simulink model "simulator_prototype_v2"  (R2021b)
(part 6 of 12)

t2391 = ct{934};
t2393 = ct{935};
t2394 = ct{936};
t2395 = ct{937};
t2396 = ct{938};
t2397 = ct{939};
t2398 = ct{940};
t2399 = ct{941};
t24 = ct{942};
t2400 = ct{943};
t2401 = ct{944};
t2402 = ct{945};
t2403 = ct{946};
t2404 = ct{947};
t2405 = ct{948};
t2408 = ct{949};
t2409 = ct{950};
t241 = ct{951};
t2410 = ct{952};
t2411 = ct{953};
t2412 = ct{954};
t2413 = ct{955};
t2414 = ct{956};
t2416 = ct{957};
t2417 = ct{958};
t2418 = ct{959};
t2419 = ct{960};
t2421 = ct{961};
t2422 = ct{962};
t2423 = ct{963};
t2425 = ct{964};
t2426 = ct{965};
t2427 = ct{966};
t2431 = ct{967};
t2432 = ct{968};
t2433 = ct{969};
t2434 = ct{970};
t2438 = ct{971};
t2440 = ct{972};
t2441 = ct{973};
t2444 = ct{974};
t2446 = ct{975};
t2447 = ct{976};
t2448 = ct{977};
t2449 = ct{978};
t2450 = ct{979};
t2451 = ct{980};
t2455 = ct{981};
t2457 = ct{982};
t2458 = ct{983};
t2459 = ct{984};
t2460 = ct{985};
t2461 = ct{986};
t2463 = ct{987};
t2465 = ct{988};
t2466 = ct{989};
t2467 = ct{990};
t2468 = ct{991};
t2470 = ct{992};
t2471 = ct{993};
t2472 = ct{994};
t2473 = ct{995};
t2474 = ct{996};
t2476 = ct{997};
t2477 = ct{998};
t2478 = ct{999};
t2479 = ct{1000};
t2480 = ct{1001};
t2481 = ct{1002};
t2484 = ct{1003};
t2485 = ct{1004};
t2487 = ct{1005};
t2488 = ct{1006};
t2489 = ct{1007};
t2490 = ct{1008};
t2491 = ct{1009};
t2492 = ct{1010};
t2493 = ct{1011};
t2494 = ct{1012};
t2496 = ct{1013};
t2497 = ct{1014};
t2498 = ct{1015};
t2499 = ct{1016};
t25 = ct{1017};
t2500 = ct{1018};
t2502 = ct{1019};
t2503 = ct{1020};
t2504 = ct{1021};
t2505 = ct{1022};
t2507 = ct{1023};
t2508 = ct{1024};
t2509 = ct{1025};
t2510 = ct{1026};
t2511 = ct{1027};
t2512 = ct{1028};
t2514 = ct{1029};
t2515 = ct{1030};
t2516 = ct{1031};
t2517 = ct{1032};
t2520 = ct{1033};
t2521 = ct{1034};
t2522 = ct{1035};
t2524 = ct{1036};
t2525 = ct{1037};
t2526 = ct{1038};
t2527 = ct{1039};
t2528 = ct{1040};
t2529 = ct{1041};
t2530 = ct{1042};
t2531 = ct{1043};
t2532 = ct{1044};
t2534 = ct{1045};
t2535 = ct{1046};
t2539 = ct{1047};
t2541 = ct{1048};
t2542 = ct{1049};
t2548 = ct{1050};
t2549 = ct{1051};
t2550 = ct{1052};
t2552 = ct{1053};
t2554 = ct{1054};
t2555 = ct{1055};
t2556 = ct{1056};
t2557 = ct{1057};
t2558 = ct{1058};
t2559 = ct{1059};
t2560 = ct{1060};
t2564 = ct{1061};
t2565 = ct{1062};
t2566 = ct{1063};
t2569 = ct{1064};
t257 = ct{1065};
t2570 = ct{1066};
t2571 = ct{1067};
t2572 = ct{1068};
t2575 = ct{1069};
t2577 = ct{1070};
t2578 = ct{1071};
t2579 = ct{1072};
t2580 = ct{1073};
t2581 = ct{1074};
t2582 = ct{1075};
t2583 = ct{1076};
t2584 = ct{1077};
t2585 = ct{1078};
t2586 = ct{1079};
t2587 = ct{1080};
t2589 = ct{1081};
t259 = ct{1082};
t2595 = ct{1083};
t2597 = ct{1084};
t2599 = ct{1085};
t26 = ct{1086};
t2600 = ct{1087};
t2601 = ct{1088};
t2603 = ct{1089};
t2604 = ct{1090};
t2605 = ct{1091};
t2606 = ct{1092};
t261 = ct{1093};
t2610 = ct{1094};
t2611 = ct{1095};
t2612 = ct{1096};
t2613 = ct{1097};
t2614 = ct{1098};
t2616 = ct{1099};
t2618 = ct{1100};
t2619 = ct{1101};
t262 = ct{1102};
t2620 = ct{1103};
t2621 = ct{1104};
t2622 = ct{1105};
t2623 = ct{1106};
t2624 = ct{1107};
t2626 = ct{1108};
t2627 = ct{1109};
t2628 = ct{1110};
t2629 = ct{1111};
t2630 = ct{1112};
t2632 = ct{1113};
t2633 = ct{1114};
t2634 = ct{1115};
t2635 = ct{1116};
t2638 = ct{1117};
t264 = ct{1118};
t2640 = ct{1119};
t2641 = ct{1120};
t2642 = ct{1121};
t2643 = ct{1122};
t2644 = ct{1123};
t2645 = ct{1124};
t2646 = ct{1125};
t2647 = ct{1126};
t2648 = ct{1127};
t2649 = ct{1128};
t2650 = ct{1129};
t2651 = ct{1130};
t2652 = ct{1131};
t2653 = ct{1132};
t2654 = ct{1133};
t2655 = ct{1134};
t2657 = ct{1135};
t2658 = ct{1136};
t2659 = ct{1137};
t2660 = ct{1138};
t2661 = ct{1139};
t2662 = ct{1140};
t2664 = ct{1141};
t2665 = ct{1142};
t2666 = ct{1143};
t2667 = ct{1144};
t2668 = ct{1145};
t2670 = ct{1146};
t2671 = ct{1147};
t2672 = ct{1148};
t2673 = ct{1149};
t2674 = ct{1150};
t2675 = ct{1151};
t2676 = ct{1152};
t2678 = ct{1153};
t2679 = ct{1154};
t2680 = ct{1155};
t2681 = ct{1156};
t2682 = ct{1157};
t2683 = ct{1158};
t2684 = ct{1159};
t2685 = ct{1160};
t2686 = ct{1161};
t2687 = ct{1162};
t2688 = ct{1163};
t2691 = ct{1164};
t2692 = ct{1165};
t2694 = ct{1166};
t2695 = ct{1167};
t2697 = ct{1168};
t2698 = ct{1169};
t2699 = ct{1170};
t27 = ct{1171};
t2701 = ct{1172};
t2703 = ct{1173};
t2707 = ct{1174};
t2708 = ct{1175};
t2709 = ct{1176};
t271 = ct{1177};
t2710 = ct{1178};
t2711 = ct{1179};
t2712 = ct{1180};
t2714 = ct{1181};
t2716 = ct{1182};
t2732 = ct{1183};
t2733 = ct{1184};
t2735 = ct{1185};
t2736 = ct{1186};
t2737 = ct{1187};
t2738 = ct{1188};
t2739 = ct{1189};
t2740 = ct{1190};
t2742 = ct{1191};
t2743 = ct{1192};
t2744 = ct{1193};
t2745 = ct{1194};
t2748 = ct{1195};
t2749 = ct{1196};
t2750 = ct{1197};
t2753 = ct{1198};
t2754 = ct{1199};
t2757 = ct{1200};
t2759 = ct{1201};
t276 = ct{1202};
t2762 = ct{1203};
t2765 = ct{1204};
t2769 = ct{1205};
t2771 = ct{1206};
t2773 = ct{1207};
t2774 = ct{1208};
t2775 = ct{1209};
t2777 = ct{1210};
t2778 = ct{1211};
t2779 = ct{1212};
t2781 = ct{1213};
t2785 = ct{1214};
t2786 = ct{1215};
t2787 = ct{1216};
t2788 = ct{1217};
t279 = ct{1218};
t2790 = ct{1219};
t2791 = ct{1220};
t2792 = ct{1221};
t2793 = ct{1222};
t2795 = ct{1223};
t2796 = ct{1224};
t2797 = ct{1225};
t2798 = ct{1226};
t2799 = ct{1227};
t28 = ct{1228};
t280 = ct{1229};
t2801 = ct{1230};
t2802 = ct{1231};
t2803 = ct{1232};
t2804 = ct{1233};
t2805 = ct{1234};
t2806 = ct{1235};
t2807 = ct{1236};
t2808 = ct{1237};
t2810 = ct{1238};
t2811 = ct{1239};
t2812 = ct{1240};
t2813 = ct{1241};
t2814 = ct{1242};
t2817 = ct{1243};
t2818 = ct{1244};
t2819 = ct{1245};
t2820 = ct{1246};
t2823 = ct{1247};
t2825 = ct{1248};
t2831 = ct{1249};
t2832 = ct{1250};
t2835 = ct{1251};
t2838 = ct{1252};
t2850 = ct{1253};
t2851 = ct{1254};
t2857 = ct{1255};
t2858 = ct{1256};
t2859 = ct{1257};
t286 = ct{1258};
t2865 = ct{1259};
t2867 = ct{1260};
t2868 = ct{1261};
t2870 = ct{1262};
t2875 = ct{1263};
t2883 = ct{1264};
t2884 = ct{1265};
t2886 = ct{1266};
t2890 = ct{1267};
t2893 = ct{1268};
t2894 = ct{1269};
t2895 = ct{1270};
t2898 = ct{1271};
t29 = ct{1272};
t2900 = ct{1273};
t2901 = ct{1274};
t2903 = ct{1275};
t2905 = ct{1276};
t2909 = ct{1277};
t2911 = ct{1278};
t2914 = ct{1279};
t2917 = ct{1280};
t2918 = ct{1281};
t2919 = ct{1282};
t2920 = ct{1283};
t2922 = ct{1284};
t2923 = ct{1285};
t2925 = ct{1286};
t2926 = ct{1287};
t2927 = ct{1288};
t293 = ct{1289};
t2930 = ct{1290};
t2931 = ct{1291};
t2933 = ct{1292};
t2935 = ct{1293};
t2937 = ct{1294};
t2941 = ct{1295};
t2942 = ct{1296};
t2943 = ct{1297};
t2944 = ct{1298};
t2947 = ct{1299};
t2948 = ct{1300};
t2949 = ct{1301};
t2950 = ct{1302};
t2951 = ct{1303};
t2952 = ct{1304};
t2955 = ct{1305};
t2956 = ct{1306};
t2961 = ct{1307};
t2962 = ct{1308};
t2963 = ct{1309};
t2964 = ct{1310};
t2965 = ct{1311};
t2966 = ct{1312};
t2969 = ct{1313};
t2970 = ct{1314};
t2971 = ct{1315};
t2972 = ct{1316};
t2973 = ct{1317};
t2975 = ct{1318};
t2976 = ct{1319};
t2977 = ct{1320};
t2978 = ct{1321};
t2979 = ct{1322};
t2981 = ct{1323};
t2982 = ct{1324};
t2983 = ct{1325};
t2984 = ct{1326};
t2986 = ct{1327};
t2987 = ct{1328};
t2990 = ct{1329};
t2991 = ct{1330};
t2993 = ct{1331};
t2999 = ct{1332};
t30 = ct{1333};
t3000 = ct{1334};
t3004 = ct{1335};
t3005 = ct{1336};
t3008 = ct{1337};
t3010 = ct{1338};
t3011 = ct{1339};
t3012 = ct{1340};
t3015 = ct{1341};
t3017 = ct{1342};
t3018 = ct{1343};
t3019 = ct{1344};
t3022 = ct{1345};
t3023 = ct{1346};
t3026 = ct{1347};
t3027 = ct{1348};
t3029 = ct{1349};
t3030 = ct{1350};
t3036 = ct{1351};
t3037 = ct{1352};
t3042 = ct{1353};
t3043 = ct{1354};
t3044 = ct{1355};
t3045 = ct{1356};
t3049 = ct{1357};
t305 = ct{1358};
t3050 = ct{1359};
t3051 = ct{1360};
t3054 = ct{1361};
t3057 = ct{1362};
t3058 = ct{1363};
t306 = ct{1364};
t3064 = ct{1365};
t3065 = ct{1366};
t3066 = ct{1367};
t3067 = ct{1368};
t3068 = ct{1369};
t3069 = ct{1370};
t3072 = ct{1371};
t3074 = ct{1372};
t3075 = ct{1373};
t3076 = ct{1374};
t3077 = ct{1375};
t3079 = ct{1376};
t308 = ct{1377};
t3080 = ct{1378};
t3081 = ct{1379};
t3082 = ct{1380};
t3083 = ct{1381};
t3085 = ct{1382};
t3086 = ct{1383};
t3087 = ct{1384};
t3088 = ct{1385};
t31 = ct{1386};
t310 = ct{1387};
t3119 = ct{1388};
t312 = ct{1389};
t3120 = ct{1390};
t313 = ct{1391};
t3130 = ct{1392};
t314 = ct{1393};
t3154 = ct{1394};
t3155 = ct{1395};
t316 = ct{1396};
t3160 = ct{1397};
t3166 = ct{1398};
t3172 = ct{1399};
t3173 = ct{1400};
t319 = ct{1401};
t32 = ct{1402};
t321 = ct{1403};
t322 = ct{1404};
t326 = ct{1405};
t328 = ct{1406};
t329 = ct{1407};
t33 = ct{1408};
t330 = ct{1409};
t331 = ct{1410};
t3313 = ct{1411};
t3315 = ct{1412};
t332 = ct{1413};
t3320 = ct{1414};
t3327 = ct{1415};
t333 = ct{1416};
t335 = ct{1417};
t336 = ct{1418};
t338 = ct{1419};
t3381 = ct{1420};
t3382 = ct{1421};
t3384 = ct{1422};
t3385 = ct{1423};
t339 = ct{1424};
t3390 = ct{1425};
t3391 = ct{1426};
t34 = ct{1427};
t341 = ct{1428};
t343 = ct{1429};
t346 = ct{1430};
t347 = ct{1431};
t3470 = ct{1432};
t3471 = ct{1433};
t35 = ct{1434};
t350 = ct{1435};
t351 = ct{1436};
t352 = ct{1437};
t3523 = ct{1438};
t3533 = ct{1439};
t354 = ct{1440};
t356 = ct{1441};
t358 = ct{1442};
t359 = ct{1443};
t36 = ct{1444};
t360 = ct{1445};
t362 = ct{1446};
t363 = ct{1447};
t3638 = ct{1448};
t364 = ct{1449};
t3649 = ct{1450};
t365 = ct{1451};
t366 = ct{1452};
t369 = ct{1453};
t370 = ct{1454};
t371 = ct{1455};
t372 = ct{1456};
t3767 = ct{1457};
t378 = ct{1458};
t38 = ct{1459};
t380 = ct{1460};
t3806 = ct{1461};
t3807 = ct{1462};
t382 = ct{1463};
t3837 = ct{1464};
t3838 = ct{1465};
t387 = ct{1466};
t3875 = ct{1467};
t3876 = ct{1468};
t3877 = ct{1469};
t3878 = ct{1470};
t3879 = ct{1471};
t39 = ct{1472};
t393 = ct{1473};
t3974 = ct{1474};
t3995 = ct{1475};
t4035 = ct{1476};
t410 = ct{1477};
t4147 = ct{1478};
t4153 = ct{1479};
t4154 = ct{1480};
t42 = ct{1481};
t4260 = ct{1482};
t428 = ct{1483};
t429 = ct{1484};
t43 = ct{1485};
t4314 = ct{1486};
t4325 = ct{1487};
t4327 = ct{1488};
t4334 = ct{1489};
t4338 = ct{1490};
t4343 = ct{1491};
t4476 = ct{1492};
t4563 = ct{1493};
t46 = ct{1494};
t461 = ct{1495};
t4683 = ct{1496};
t47 = ct{1497};
t4705 = ct{1498};
t4716 = ct{1499};
t473 = ct{1500};
t474 = ct{1501};
t4762 = ct{1502};
t4763 = ct{1503};
t480 = ct{1504};
t4847 = ct{1505};
t4850 = ct{1506};
t498 = ct{1507};
t50 = ct{1508};
t5025 = ct{1509};
t5027 = ct{1510};
t503 = ct{1511};
t5036 = ct{1512};
t504 = ct{1513};
t506 = ct{1514};
t510 = ct{1515};
t514 = ct{1516};
t516 = ct{1517};
t521 = ct{1518};
t522 = ct{1519};
t523 = ct{1520};
t524 = ct{1521};
t528 = ct{1522};
t5296 = ct{1523};
t530 = ct{1524};
t535 = ct{1525};
t5370 = ct{1526};
t538 = ct{1527};
t539 = ct{1528};
t542 = ct{1529};
t543 = ct{1530};
t5437 = ct{1531};
t549 = ct{1532};
t56 = ct{1533};
t562 = ct{1534};
t563 = ct{1535};
t564 = ct{1536};
t573 = ct{1537};
t575 = ct{1538};
t577 = ct{1539};
t579 = ct{1540};
t58 = ct{1541};
t580 = ct{1542};
t581 = ct{1543};
t587 = ct{1544};
t59 = ct{1545};
t593 = ct{1546};
t594 = ct{1547};
t598 = ct{1548};
t60 = ct{1549};
t610 = ct{1550};
t611 = ct{1551};
t612 = ct{1552};
t614 = ct{1553};
t615 = ct{1554};
t616 = ct{1555};
t623 = ct{1556};
t624 = ct{1557};
t628 = ct{1558};
t635 = ct{1559};
t636 = ct{1560};
t638 = ct{1561};
t640 = ct{1562};
t641 = ct{1563};
t642 = ct{1564};
t643 = ct{1565};
t644 = ct{1566};
t645 = ct{1567};
t646 = ct{1568};
t648 = ct{1569};
t649 = ct{1570};
t654 = ct{1571};
t655 = ct{1572};
t656 = ct{1573};
t657 = ct{1574};
t658 = ct{1575};
t659 = ct{1576};
t660 = ct{1577};
t662 = ct{1578};
t663 = ct{1579};
t664 = ct{1580};
t665 = ct{1581};
t666 = ct{1582};
t667 = ct{1583};
t668 = ct{1584};
t669 = ct{1585};
t67 = ct{1586};
t670 = ct{1587};
t672 = ct{1588};
t673 = ct{1589};
t674 = ct{1590};
t675 = ct{1591};
t676 = ct{1592};
t677 = ct{1593};
t678 = ct{1594};
t679 = ct{1595};
t68 = ct{1596};
t680 = ct{1597};
t681 = ct{1598};
t682 = ct{1599};
t683 = ct{1600};
t684 = ct{1601};
t685 = ct{1602};
t686 = ct{1603};
t687 = ct{1604};
t689 = ct{1605};
t691 = ct{1606};
t692 = ct{1607};
t693 = ct{1608};
t694 = ct{1609};
t696 = ct{1610};
t698 = ct{1611};
t70 = ct{1612};
t702 = ct{1613};
t704 = ct{1614};
t705 = ct{1615};
t707 = ct{1616};
t708 = ct{1617};
t71 = ct{1618};
t710 = ct{1619};
t711 = ct{1620};
t712 = ct{1621};
t713 = ct{1622};
t714 = ct{1623};
t715 = ct{1624};
t716 = ct{1625};
t717 = ct{1626};
t718 = ct{1627};
t719 = ct{1628};
t720 = ct{1629};
t721 = ct{1630};
t722 = ct{1631};
t723 = ct{1632};
t724 = ct{1633};
t725 = ct{1634};
t726 = ct{1635};
t728 = ct{1636};
t73 = ct{1637};
t733 = ct{1638};
t736 = ct{1639};
t738 = ct{1640};
t740 = ct{1641};
t741 = ct{1642};
t742 = ct{1643};
t743 = ct{1644};
t744 = ct{1645};
t745 = ct{1646};
t746 = ct{1647};
t747 = ct{1648};
t749 = ct{1649};
t750 = ct{1650};
t751 = ct{1651};
t755 = ct{1652};
t756 = ct{1653};
t757 = ct{1654};
t758 = ct{1655};
t759 = ct{1656};
t76 = ct{1657};
t762 = ct{1658};
t763 = ct{1659};
t764 = ct{1660};
t766 = ct{1661};
t767 = ct{1662};
t768 = ct{1663};
t770 = ct{1664};
t771 = ct{1665};
t772 = ct{1666};
t773 = ct{1667};
t774 = ct{1668};
t775 = ct{1669};
t776 = ct{1670};
t777 = ct{1671};
t778 = ct{1672};
t781 = ct{1673};
t782 = ct{1674};
t783 = ct{1675};
t784 = ct{1676};
t785 = ct{1677};
t786 = ct{1678};
t787 = ct{1679};
t789 = ct{1680};
t790 = ct{1681};
t791 = ct{1682};
t792 = ct{1683};
t793 = ct{1684};
t794 = ct{1685};
t796 = ct{1686};
t797 = ct{1687};
t798 = ct{1688};
t799 = ct{1689};
t8 = ct{1690};
t800 = ct{1691};
t801 = ct{1692};
t802 = ct{1693};
t806 = ct{1694};
t807 = ct{1695};
t808 = ct{1696};
t809 = ct{1697};
t812 = ct{1698};
t813 = ct{1699};
t816 = ct{1700};
t817 = ct{1701};
t818 = ct{1702};
t819 = ct{1703};
t820 = ct{1704};
t821 = ct{1705};
t822 = ct{1706};
t823 = ct{1707};
t824 = ct{1708};
t825 = ct{1709};
t826 = ct{1710};
t827 = ct{1711};
t828 = ct{1712};
t829 = ct{1713};
t830 = ct{1714};
t831 = ct{1715};
t832 = ct{1716};
t833 = ct{1717};
t850 = ct{1718};
t855 = ct{1719};
t856 = ct{1720};
t874 = ct{1721};
t878 = ct{1722};
t89 = ct{1723};
t893 = ct{1724};
t9 = ct{1725};
t90 = ct{1726};
t91 = ct{1727};
t911 = ct{1728};
t92 = ct{1729};
t925 = ct{1730};
t926 = ct{1731};
t936 = ct{1732};
t937 = ct{1733};
t940 = ct{1734};
t941 = ct{1735};
t942 = ct{1736};
t944 = ct{1737};
t945 = ct{1738};
t948 = ct{1739};
t949 = ct{1740};
t950 = ct{1741};
t951 = ct{1742};
t959 = ct{1743};
t961 = ct{1744};
t965 = ct{1745};
t966 = ct{1746};
t97 = ct{1747};
t974 = ct{1748};
t978 = ct{1749};
t983 = ct{1750};
t987 = ct{1751};
t989 = ct{1752};
t99 = ct{1753};
t990 = ct{1754};
t991 = ct{1755};
t992 = ct{1756};
t993 = ct{1757};
t995 = ct{1758};
t996 = ct{1759};
t998 = ct{1760};
t3121 = t35.*t991.*t2699.*2.196325630278387e-1;
t3122 = t36.*t991.*t2699.*2.196325630278387e-1;
t3126 = t50.*t202.*t2981.*4.771516396025243e-17;
t3127 = t50.*t202.*t2981.*9.543032792050485e-17;
t3131 = (t2307.*t2363)./1.0e+8;
t3132 = (t2297.*t2388)./1.0e+8;
t3134 = t2363.*t2554;
t3137 = t38.*t1022.*(t855-t878).*(-2.196325630278387e-1);
t3138 = t39.*t1022.*(t855-t878).*(-2.196325630278387e-1);
t3140 = (t2297.*t2419)./1.0e+8;
t3141 = (t2338.*t2363)./1.0e+8;
t3144 = t35.*t991.*t2699.*1.122398993609262e-1;
t3145 = t36.*t991.*t2699.*1.122398993609262e-1;
t3148 = t35.*t991.*t2699.*1.887873611596568e-1;
t3149 = t36.*t991.*t2699.*1.887873611596568e-1;
t3150 = t35.*t991.*t2699.*5.076068728976717e-3;
t3151 = t36.*t991.*t2699.*5.076068728976717e-3;
t3157 = t2307.*t2363.*6.2e-7;
t3158 = t2297.*t2388.*6.2e-7;
t3159 = t2363.*t2801;
t3163 = t2297.*t2419.*6.2e-7;
t3164 = t2338.*t2363.*6.2e-7;
t3165 = t2363.*t2831;
t3168 = t38.*t1022.*(t855-t878).*(-1.122398993609262e-1);
t3169 = t39.*t1022.*(t855-t878).*(-1.122398993609262e-1);
t3170 = t2363.*t2850;
t3171 = t2363.*t2851;
t3174 = t38.*t1022.*(t855-t878).*(-1.887873611596568e-1);
t3175 = t39.*t1022.*(t855-t878).*(-1.887873611596568e-1);
t3176 = t39.*t1022.*(t855-t878).*1.887873611596568e-1;
t3177 = t38.*t1022.*(t855-t878).*(-5.076068728976717e-3);
t3178 = t39.*t1022.*(t855-t878).*(-5.076068728976717e-3);
t3179 = t38.*t1022.*(t855-t878).*5.076068728976717e-3;
t3180 = t39.*t1022.*(t855-t878).*5.076068728976717e-3;
t3182 = t2363.*t2973;
t3183 = t2388.*t2971;
t3184 = t2388.*t2972;
t3186 = t2388.*t2973;
t3191 = t2399.*t2973;
t3204 = t2363.*t2976;
t3210 = t38.*t1022.*(t855-t878).*(-1.46680315462752e-4);
t3211 = t39.*t1022.*(t855-t878).*(-1.46680315462752e-4);
t3212 = t39.*t1022.*(t855-t878).*1.46680315462752e-4;
t3213 = t598+t1904+t2554;
t3274 = t35.*t941.*t948.*(t850-t874).*(-4.392651260556773e-1);
t3275 = t36.*t941.*t948.*(t850-t874).*(-4.392651260556773e-1);
t3276 = t35.*t941.*t948.*(t850-t874).*4.392651260556773e-1;
t3277 = t36.*t941.*t948.*(t850-t874).*4.392651260556773e-1;
t3318 = t201.*t3166.*4.297799892626299e-1;
t3319 = t201.*t3166.*8.595599785252598e-1;
t3322 = t535+t577+t1887+t1940;
t3369 = t564+t611+t1929+t1967;
t3371 = t35.*t941.*t948.*(t850-t874).*(-2.244797987218524e-1);
t3372 = t36.*t941.*t948.*(t850-t874).*(-2.244797987218524e-1);
t3373 = t36.*t941.*t948.*(t850-t874).*(-3.775747223193135e-1);
t3374 = t35.*t941.*t948.*(t850-t874).*(-3.775747223193135e-1);
t3375 = t36.*t941.*t948.*(t850-t874).*3.775747223193135e-1;
t3377 = t35.*t941.*t948.*(t850-t874).*(-1.015213745795343e-2);
t3378 = t36.*t941.*t948.*(t850-t874).*(-1.015213745795343e-2);
t3379 = t35.*t941.*t948.*(t850-t874).*1.015213745795343e-2;
t3380 = t36.*t941.*t948.*(t850-t874).*1.015213745795343e-2;
t3388 = -t3385;
t3393 = -t3390;
t3394 = -t3391;
t3427 = t50.*t202.*t3166.*9.543032792050485e-17;
t3472 = -t3471;
t3484 = t2363.*t3155;
t3485 = t2388.*t3155;
t3487 = t2419.*t3155;
t3499 = t998+t1036+t1059+t1481+t1519;
t3517 = t1019+t1060+t1072+t1503+t1537;
t3805 = t1021+t1024+t1053+t1490+t1498+t1512;
t3809 = t1582+t1647+t1769+t1961+t2034;
t3880 = t1619+t1739+t1774+t1991+t2057+t2079;
t3897 = t58+t59+t3878;
t3898 = t56+t73+t3879;
t3901 = t539+t577+t581+t593+t1909+t1937+t1939+t1940;
t3902 = t538+t573+t575+t579+t1924+t1935+t1936+t1957;
t3903 = t1038+t1043+t1056+t1057+t1501+t1507+t1517+t1531;
t3944 = -t20.*(t1941-t3315+t39.*t1022.*(t855-t878).*2.196325630278387e-1);
t3945 = -t26.*(t1941-t3315+t39.*t1022.*(t855-t878).*2.196325630278387e-1);
t3947 = -t21.*(t1959-t3313+t38.*t1022.*(t855-t878).*2.196325630278387e-1);
t3948 = -t27.*(t1959-t3313+t38.*t1022.*(t855-t878).*2.196325630278387e-1);
t3950 = t21.*(t1959-t3313+t38.*t1022.*(t855-t878).*2.196325630278387e-1).*(-3.0./5.0e+2);
t3982 = t27.*(t1959-t3313+t38.*t1022.*(t855-t878).*2.196325630278387e-1).*(-1.247162e-2);
t3989 = t20.*(t1941-t3315+t39.*t1022.*(t855-t878).*2.196325630278387e-1).*(-5.84482e-3);
t3990 = t27.*(t1959-t3313+t38.*t1022.*(t855-t878).*2.196325630278387e-1).*1.247162e-2;
t3994 = t20.*(t1941-t3315+t39.*t1022.*(t855-t878).*2.196325630278387e-1).*(-6.48e-5);
t4000 = t21.*(t1959-t3313+t38.*t1022.*(t855-t878).*2.196325630278387e-1).*(-3.131399999999998e-4);
t4003 = t26.*(t1941-t3315+t39.*t1022.*(t855-t878).*2.196325630278387e-1).*(-6.47e-6);
t4004 = t21.*(t1959-t3313+t38.*t1022.*(t855-t878).*2.196325630278387e-1).*(-4.36041e-5);
t4005 = t26.*(t1941-t3315+t39.*t1022.*(t855-t878).*2.196325630278387e-1).*6.47e-6;
t4008 = t1000+t1002+t1006+t1028+t1040+t1054+t1493+t1500+t1506;
t4038 = t20.*(t1941-t3315+t39.*t1022.*(t855-t878).*2.196325630278387e-1).*(-1.688944904408e-4);
t4040 = t21.*(t1959-t3313+t38.*t1022.*(t855-t878).*2.196325630278387e-1).*(-6.1855407534e-5);
t4043 = t27.*(t1959-t3313+t38.*t1022.*(t855-t878).*2.196325630278387e-1).*(-1.35652563578e-4);
t4044 = t20.*(t1941-t3315+t39.*t1022.*(t855-t878).*2.196325630278387e-1).*1.688944904408e-4;
t4050 = t20.*(t1941-t3315+t39.*t1022.*(t855-t878).*2.196325630278387e-1).*(-7.0482312e-7);
t4055 = t26.*(t1941-t3315+t39.*t1022.*(t855-t878).*2.196325630278387e-1).*(-1.869599668e-7);
t4057 = t20.*(t1941-t3315+t39.*t1022.*(t855-t878).*2.196325630278387e-1).*7.0482312e-7;
t4167 = -t28.*(t1005+t20.*(t1941-t3315+t39.*t1022.*(t855-t878).*2.196325630278387e-1));
t4170 = -t22.*(t1005+t20.*(t1941-t3315+t39.*t1022.*(t855-t878).*2.196325630278387e-1));
t4177 = t22.*(t1005+t20.*(t1941-t3315+t39.*t1022.*(t855-t878).*2.196325630278387e-1));
t4222 = t28.*(t1005+t20.*(t1941-t3315+t39.*t1022.*(t855-t878).*2.196325630278387e-1)).*(-1.838876e-2);
t4232 = t50.*t189.*(t1941-t3315+t39.*t1022.*(t855-t878).*2.196325630278387e-1).*(-4.306286555174926e-24);
t4234 = t50.*t189.*(t1959-t3313+t38.*t1022.*(t855-t878).*2.196325630278387e-1).*(-7.660522649005482e-24);
t4255 = t28.*(t1005+t20.*(t1941-t3315+t39.*t1022.*(t855-t878).*2.196325630278387e-1)).*(-1.33637554986e-4);
t4273 = t1098+t1129+t1142+t1156+t2455+t2484+t2490+t2524;
t4274 = t1099+t1135+t1160+t1169+t2451+t2457+t2511+t2512;
t4275 = t1699+t1745+t1767+t1768+t2039+t2093+t2095+t2107;
t4313 = t312+t316+t4153;
t4315 = t314+t319+t4154;
t4324 = t1593+t1621+t1625+t1632+t1743+t1778+t1997+t2035+t2094;
t4326 = t1592+t1603+t1610+t1875+t1883+t1891+t1910+t1925+t1934;
t4348 = -t3166.*(t1959-t3313+t38.*t1022.*(t855-t878).*2.196325630278387e-1);
t4349 = t99+t107+t108+t124+t130+t139+t280+t286+t305+t310+t614+t623+t624+t658+t698+t767+t993+t995+t1011+t1033;
t4351 = t216+t230+t261+t276+t474+t480+t503+t510+t926+t936+t961+t987+t1432+t1439+t1464+t1465;
t4375 = t100+t101+t126+t128+t134+t257+t279+t293+t306+t308+t615+t616+t662+t696+t733+t978+t990+t992+t1034+t1037;
t4421 = -t3155.*(t1005+t20.*(t1941-t3315+t39.*t1022.*(t855-t878).*2.196325630278387e-1));
t4424 = t3155.*(t1005+t20.*(t1941-t3315+t39.*t1022.*(t855-t878).*2.196325630278387e-1));
t4501 = t2143+t2161+t2163+t2340+t2409+t2411+t2425+t2485+t2489;
t4502 = t1444+t1462+t1476+t1487+t1489+t1495+t1534+t1540+t1850+t1857+t1867+t1869;
t4652 = t680+t942+t965+t1103+t1133+t1200+t1211+t1510+t1551+t1555+t1556+t1557+t1574+t1575;
t4663 = (t3837.*t3876)./2.0;
t4664 = (t3838.*t3877)./2.0;
t4704 = (t3806.*t4147)./2.0;
t4707 = t3807.*(t1089-t1104-t1105-t1121-t2117+t2120+t2122+t2123).*(-1.0./2.0);
t4708 = (t3807.*(t1089-t1104-t1105-t1121-t2117+t2120+t2122+t2123))./2.0;
t4709 = t925+t1331+t1372+t1453+t1457+t1472+t1502+t1508+t1786+t1801+t1803+t1818+t1856+t1858;
t4729 = t3807.*(t313-t314-t1108+t1115-t1158-t1159-t2117+t2120+t2122+t2123).*(-1.0./2.0);
t4730 = (t3807.*(t313-t314-t1108+t1115-t1158-t1159-t2117+t2120+t2122+t2123))./2.0;
t4900 = t3878.*(t313-t314-t1108+t1115-t1158-t1159-t2117+t2120+t2122+t2123).*(-1.0./2.0);
t4902 = (t3878.*(t313-t314-t1108+t1115-t1158-t1159-t2117+t2120+t2122+t2123))./2.0;
t5037 = t151+t182+t203+t231+t239+t259+t271+t393+t428+t461+t473+t498+t504+t506+t856+t893+t911+t937+t940+t959+t966+t1195+t1266+t1377+t1388+t1431+t1466+t1467;
t5278 = t704+t705+t726+t728+t755+t778+t781+t797+t1670+t1675+t1713+t1714+t1718+t1719+t1733+t1734+t1988+t1990+t2009+t2010+t2017+t2027+t2036+t2074;
t5279 = t719+t742+t747+t750+t751+t763+t773+t775+t1642+t1655+t1657+t1662+t1663+t1684+t1709+t1724+t1984+t2005+t2031+t2033+t2052+t2059+t2067+t2068;
t5282 = t236.*t241.*t4035.*t4705.*1.16903445774439e-94;
t5308 = t236.*t241.*t3974.*t4716.*1.16903445774439e-94;
t5309 = t236.*t241.*t3995.*t4716.*2.394182569460511e-91;
t5361 = t236.*t241.*t4314.*t4705.*2.156487945535858e-75;
t5363 = t236.*t241.*t4260.*t4716.*2.156487945535858e-75;
t5372 = t236.*t241.*t3995.*t4850.*2.658076613771277e-107;
t5381 = t236.*t241.*t4334.*t4705.*2.394182569460511e-91;
t5391 = t236.*t241.*t4325.*t4716.*2.394182569460511e-91;
t5395 = t236.*t241.*t4327.*t4716.*2.156487945535858e-75;
t5402 = t236.*t241.*t4343.*t4716.*2.156487945535858e-75;
t5404 = t236.*t241.*t4338.*t4716.*1.16903445774439e-94;
t5433 = t236.*t241.*t4334.*t4763.*2.658076613771277e-107;
t5434 = t236.*t241.*t4325.*t4850.*2.658076613771277e-107;
t5435 = t236.*t241.*t4035.*t5025.*6.337348493984406e-114;
t5439 = t236.*t241.*t4327.*t4850.*2.394182569460511e-91;
t5450 = t236.*t241.*t3974.*t5036.*6.337348493984406e-114;
t5457 = t236.*t241.*t3995.*t5036.*1.297888971568006e-110;
t5459 = t236.*t241.*t4343.*t4850.*2.394182569460511e-91;
t5463 = t236.*t241.*t4338.*t4850.*1.297888971568006e-110;
t5481 = t236.*t241.*t4314.*t5025.*1.16903445774439e-94;
t5499 = t236.*t241.*t4260.*t5036.*1.16903445774439e-94;
t5540 = t1305+t1307+t1316+t1317+t1342+t1399+t1404+t1436+t2184+t2202+t2207+t2258+t2274+t2275+t2277+t2278+t2541+t2560+t2589+t2595+t2597+t2623+t2624+t2634;
t5541 = t1300+t1311+t1337+t1338+t1379+t1392+t1394+t1398+t2179+t2181+t2200+t2201+t2232+t2241+t2271+t2276+t2580+t2582+t2587+t2611+t2629+t2630+t2655+t2662;
t5542 = t236.*t241.*t4476.*t4850.*2.658076613771277e-107;
t5545 = t236.*t241.*t4327.*t5036.*1.16903445774439e-94;
t5550 = t236.*t241.*t4338.*t5036.*6.337348493984406e-114;
t5570 = t236.*t241.*t4683.*t4850.*1.297888971568006e-110;
t5604 = t236.*t241.*t4476.*t5036.*1.297888971568006e-110;
t5684 = t236.*t241.*t4683.*t5036.*6.337348493984406e-114;
t5782 = t1076+t1078+t1079+t1097+t1119+t1120+t1125+t1127+t1128+t1136+t1140+t1144+t1152+t1153+t1164+t1175+t2417+t2418+t2426+t2431+t2432+t2444+t2466+t2467+t2476+t2477+t2480+t2481+t2491+t2505+t2514+t2516;
t5783 = t1074+t1075+t1077+t1088+t1109+t1111+t1116+t1130+t1131+t1138+t1139+t1151+t1163+t1165+t1172+t1173+t2416+t2427+t2440+t2441+t2446+t2458+t2463+t2473+t2474+t2478+t2479+t2487+t2488+t2498+t2499+t2504;
t5901 = t1811+t1812+t1821+t1822+t1823+t1824+t1825+t1830+t1837+t1838+t1839+t1846+t1851+t1852+t1855+t1859+t2858+t2859+t2867+t2868+t2886+t2894+t2895+t2903+t2905+t2914+t2919+t2922+t2923+t2925+t2933+t2935;
t5902 = t1808+t1809+t1816+t1819+t1820+t1831+t1832+t1833+t1841+t1844+t1845+t1847+t1848+t1849+t1853+t1854+t2857+t2865+t2883+t2884+t2890+t2893+t2898+t2900+t2901+t2911+t2917+t2918+t2920+t2926+t2930+t2931;
t6011 = t711+t714+t743+t759+t771+t772+t783+t784+t789+t798+t816+t817+t820+t823+t824+t827+t1634+t1645+t1646+t1680+t1696+t1697+t1707+t1708+t1720+t1723+t1731+t1732+t1762+t1779+t1781+t1787+t1979+t1980+t1999+t2001+t2043+t2058+t2061+t2062+t2065+t2066+t2081+t2082+t2084+t2102+t2108+t2109;
t6013 = t720+t723+t744+t764+t774+t776+t785+t786+t794+t800+t806+t807+t809+t812+t831+t832+t1639+t1656+t1658+t1685+t1710+t1711+t1725+t1728+t1735+t1736+t1747+t1748+t1764+t1770+t1783+t1792+t1983+t2008+t2015+t2016+t2030+t2032+t2041+t2042+t2051+t2054+t2070+t2071+t2091+t2103+t2106+t2110;
t6014 = t712+t713+t757+t758+t766+t770+t782+t790+t791+t799+t818+t822+t825+t826+t828+t829+t1644+t1677+t1679+t1687+t1698+t1706+t1721+t1722+t1729+t1730+t1744+t1760+t1761+t1763+t1788+t1789+t1981+t2002+t2003+t2013+t2037+t2044+t2045+t2063+t2064+t2075+t2083+t2085+t2086+t2100+t2101+t2105;
t6016 = t721+t722+t745+t746+t749+t777+t787+t792+t793+t796+t801+t802+t808+t819+t830+t833+t1629+t1640+t1641+t1659+t1661+t1712+t1715+t1726+t1727+t1737+t1746+t1755+t1784+t1785+t1790+t1791+t1985+t2006+t2007+t2014+t2029+t2040+t2049+t2050+t2069+t2072+t2087+t2089+t2090+t2104+t2111+t2112;
t6255 = t1285+t1299+t1324+t1343+t1352+t1366+t1367+t1376+t1386+t1387+t1389+t1407+t1408+t1417+t1428+t1429+t2177+t2178+t2190+t2191+t2198+t2210+t2211+t2230+t2234+t2261+t2265+t2266+t2267+t2283+t2285+t2288+t2548+t2549+t2565+t2566+t2599+t2616+t2620+t2621+t2628+t2641+t2645+t2646+t2648+t2657+t2661+t2668;
t6256 = t1290+t1301+t1328+t1335+t1349+t1380+t1393+t1395+t1397+t1409+t1410+t1419+t1420+t1421+t1433+t1434+t2180+t2182+t2217+t2218+t2233+t2238+t2242+t2243+t2249+t2254+t2263+t2268+t2269+t2272+t2284+t2289+t2557+t2558+t2570+t2571+t2579+t2581+t2584+t2585+t2586+t2614+t2633+t2644+t2653+t2654+t2660+t2665;
t6257 = t1286+t1287+t1322+t1323+t1354+t1368+t1374+t1375+t1385+t1406+t1414+t1415+t1416+t1427+t1441+t1448+t2176+t2192+t2209+t2216+t2224+t2227+t2229+t2237+t2259+t2260+t2264+t2273+t2281+t2282+t2286+t2287+t2550+t2552+t2564+t2577+t2578+t2600+t2601+t2622+t2626+t2627+t2635+t2642+t2643+t2647+t2649+t2650;
t6258 = t1319+t1320+t1344+t1345+t1348+t1360+t1370+t1371+t1378+t1405+t1411+t1412+t1424+t1425+t1440+t1447+t2174+t2187+t2194+t2195+t2203+t2208+t2215+t2222+t2223+t2248+t2256+t2257+t2262+t2270+t2279+t2280+t2542+t2559+t2569+t2603+t2604+t2605+t2606+t2610+t2618+t2619+t2632+t2640+t2658+t2659+t2666+t2667;
t2424 = -t2376;
t2445 = -t2387;
t2501 = t2350.*(3.0./5.0e+2);
t2506 = t2355.*(3.0./5.0e+2);
t2523 = t2390.*(3.0./5.0e+2);
t2533 = -t2521;
t2536 = -t2527;
t2537 = -t2528;
t2547 = t2496.*(3.0./5.0e+2);
t2553 = t2502.*(3.0./5.0e+2);
t2602 = t2350./1.0e+8;
t2615 = t2355./1.0e+8;
t2636 = t2522.*(3.0./5.0e+2);
t2663 = t2387./1.0e+8;
t2677 = -t2674;
t2689 = -t2681;
t2690 = -t2684;
t2693 = -t2687;
t2696 = -t2688;
t2700 = -t2692;
t2702 = -t2694;
t2704 = -t2697;
t2705 = -t2698;
t2713 = -t2707;
t2715 = -t2709;
t2717 = -t2710;
t2719 = -t2711;
t2720 = -t2712;
t2721 = -t2714;
t2746 = t2351.*9.99471e-3;
t2747 = -t2737;
t2751 = t2356.*1.838876e-2;
t2752 = -t2740;
t2755 = t2350.*1.247162e-2;
t2756 = t2355.*1.247162e-2;
t2760 = t2387.*1.247162e-2;
t2761 = t2376.*9.99471e-3;
t2764 = t2373.*1.838876e-2;
t2768 = t2350.*5.68686e-3;
t2770 = t2355.*5.68686e-3;
t2776 = t2390.*5.68686e-3;
t2784 = t2410.*9.99471e-3;
t2789 = t2412.*1.838876e-2;
t2815 = t2350.*3.131399999999998e-4;
t2816 = t2355.*3.131399999999998e-4;
t2821 = t2350.*5.7e-7;
t2822 = t2390.*3.131399999999998e-4;
t2824 = t2355.*5.7e-7;
t2826 = t2351.*9.3e-7;
t2827 = t2350.*1.02e-6;
t2828 = t2355.*1.02e-6;
t2829 = t2356.*1.02e-6;
t2830 = -t2813;
t2833 = t2497.*9.99471e-3;
t2834 = -t2817;
t2836 = t2503.*1.838876e-2;
t2837 = -t2820;
t2839 = t2373.*1.02e-6;
t2840 = t2376.*9.3e-7;
t2843 = t2350.*2.4e-7;
t2844 = t2496.*1.247162e-2;
t2845 = t2390.*5.7e-7;
t2846 = t2355.*2.4e-7;
t2847 = t2502.*1.247162e-2;
t2848 = t2387.*1.02e-6;
t2852 = t2521.*1.247162e-2;
t2854 = t2351.*9.0e-8;
t2855 = t2356.*9.0e-8;
t2856 = -t2838;
t2861 = t2410.*9.3e-7;
t2864 = t2412.*1.02e-6;
t2866 = t2496.*5.68686e-3;
t2869 = t2502.*5.68686e-3;
t2871 = t2350.*4.0e-8;
t2873 = t2387.*2.4e-7;
t2874 = t2355.*4.0e-8;
t2877 = t2373.*9.0e-8;
t2878 = t2376.*9.0e-8;
t2881 = t2522.*5.68686e-3;
t2882 = t2387.*4.0e-8;
t2885 = t2390.*4.0e-8;
t2888 = t2527.*9.99471e-3;
t2889 = t2528.*9.99471e-3;
t2897 = t2526.*1.838876e-2;
t2902 = t2531.*1.838876e-2;
t2928 = t2410.*9.0e-8;
t2929 = t2412.*9.0e-8;
t2932 = t2496.*3.131399999999998e-4;
t2934 = t2502.*3.131399999999998e-4;
t2936 = t2522.*3.131399999999998e-4;
t2945 = -t2943;
t2946 = -t2944;
t2953 = -t2947;
t2954 = -t2949;
t2957 = -t2952;
t2985 = -t2983;
t2992 = t514+t2390;
t2998 = t521+t2522;
t3001 = -t2999;
t3002 = -t3000;
t3006 = -t3005;
t3013 = -t3011;
t3014 = -t3012;
t3016 = -t3015;
t3024 = -t3022;
t3025 = -t3023;
t3028 = -t3026;
t3031 = -t3030;
t3038 = -t3036;
t3039 = -t3037;
t3046 = -t3042;
t3047 = t1458+t2350;
t3048 = t1471+t2355;
t3052 = -t12.*(t1456-t2355);
t3053 = -t17.*(t1456-t2355);
t3055 = t1478+t2496;
t3056 = t1485+t2502;
t3059 = -t22.*(t1477-t2502);
t3060 = -t28.*(t1477-t2502);
t3061 = t22.*(t1477-t2502);
t3073 = -t3067;
t3078 = -t3072;
t3091 = t12.*(t1456-t2355).*(-9.99471e-3);
t3092 = t17.*(t1456-t2355).*(-9.99471e-3);
t3093 = t12.*(t1456-t2355).*(-1.838876e-2);
t3094 = t17.*(t1456-t2355).*(-1.838876e-2);
t3095 = t12.*(t1456-t2355).*9.99471e-3;
t3096 = t17.*(t1456-t2355).*9.99471e-3;
t3097 = t12.*(t1456-t2355).*1.838876e-2;
t3100 = t12.*(t1456-t2355).*(-9.3e-7);
t3101 = t12.*(t1456-t2355).*(-1.02e-6);
t3102 = t17.*(t1456-t2355).*(-9.3e-7);
t3103 = t17.*(t1456-t2355).*(-1.02e-6);
t3106 = t12.*(t1456-t2355).*9.3e-7;
t3107 = t12.*(t1456-t2355).*(-9.0e-8);
t3108 = t17.*(t1456-t2355).*(-9.0e-8);
t3109 = t12.*(t1456-t2355).*9.0e-8;
t3113 = t28.*(t1477-t2502).*(-9.99471e-3);
t3115 = t28.*(t1477-t2502).*(-1.838876e-2);
t3117 = t28.*(t1477-t2502).*9.99471e-3;
t3123 = t2356+t2373;
t3124 = -t3121;
t3125 = -t3122;
t3129 = -t3126;
t3135 = -t3131;
t3136 = -t3132;
t3142 = t2503+t2526;
t3146 = -t3144;
t3147 = -t3145;
t3152 = -t3148;
t3153 = -t3150;
t3161 = -t3157;
t3162 = -t3158;
t3188 = t201.*(t1456-t2355).*(-4.899491877593981e-7);
t3193 = t3182./2.0;
t3194 = t3183./2.0;
t3195 = t3184./2.0;
t3197 = t201.*(t1456-t2355).*(-3.438239914101039e-8);
t3202 = t201.*(t1456-t2355).*3.438239914101039e-8;
t3205 = t3191./2.0;
t3207 = -t3204;
t3208 = t3204./2.0;
t3214 = t2825+t2850;
t3215 = t2133+t3000;
t3216 = t2134+t2999;
t3220 = t50.*t202.*(t1456-t2355).*(-9.543032792050485e-25);
t3225 = t50.*t202.*(t1456-t2355).*9.543032792050485e-25;
t3235 = t2171+t3011;
t3236 = t2172+t3012;
t3262 = t50.*t202.*(t1456-t2355).*(-9.733893447891495e-23);
t3264 = t50.*t202.*(t1456-t2355).*(-5.439528691468777e-23);
t3266 = t50.*t202.*(t1456-t2355).*9.733893447891495e-23;
t3268 = t50.*t202.*(t1456-t2355).*(-2.290327870092116e-23);
t3269 = t50.*t202.*(t1456-t2355).*5.439528691468777e-23;
t3270 = t50.*t202.*(t1456-t2355).*(-3.817213116820194e-24);
t3273 = t50.*t202.*(t1456-t2355).*3.817213116820194e-24;
t3321 = t50.*t202.*t3120.*4.771516396025243e-17;
t3323 = t50.*t202.*t3120.*9.543032792050485e-17;
t3387 = t2363.*(t1456-t2355).*(-1.0e-8);
t3429 = -t3427;
t3435 = t2363.*(t1456-t2355).*(-5.7e-7);
t3438 = t2363.*(t1456-t2355).*(-1.02e-6);
t3442 = t2388.*(t1456-t2355).*(-5.7e-7);
t3443 = t2363.*(t1456-t2355).*5.7e-7;
t3447 = t2363.*(t1456-t2355).*(-2.4e-7);
t3449 = t2388.*(t1456-t2355).*5.7e-7;
t3454 = t2363.*(t1456-t2355).*(-4.0e-8);
t3459 = t2419.*(t1456-t2355).*(-5.7e-7);
t3460 = t2388.*(t1456-t2355).*(-4.0e-8);
t3461 = t2363.*(t1456-t2355).*4.0e-8;
t3465 = t2419.*(t1456-t2355).*5.7e-7;
t3466 = t2419.*(t1456-t2355).*(-4.0e-8);
t3469 = t2419.*(t1456-t2355).*4.0e-8;
t3473 = t2363.*t3119;
t3486 = -t3485;
t3488 = t3485./2.0;
t3491 = -t3487;
t3494 = t3487./2.0;
t3545 = t201.*(t2337+t12.*(t1456-t2355)).*(-8.76751178095765e-7);
t3552 = t201.*(t2337+t12.*(t1456-t2355)).*(-7.736039806727338e-8);
t3579 = t2363.*t3213;
t3620 = t347+t1539+t2831+t2875;
t3691 = t50.*t202.*(t2337+t12.*(t1456-t2355)).*(-8.875020496606951e-23);
t3693 = t50.*t202.*(t2337+t12.*(t1456-t2355)).*8.875020496606951e-23;
t3694 = t50.*t202.*(t2337+t12.*(t1456-t2355)).*(-9.733893447891495e-23);
t3696 = t50.*t202.*(t2337+t12.*(t1456-t2355)).*9.733893447891495e-23;
t3698 = t50.*t202.*(t2337+t12.*(t1456-t2355)).*(-8.588729512845436e-24);
t3699 = t50.*t202.*(t2337+t12.*(t1456-t2355)).*8.588729512845436e-24;
t3712 = t530+t1918+t2743+t2771;
t3755 = t563+t1964+t2832+t2870;
t3776 = t2363.*(t2337+t12.*(t1456-t2355)).*(-9.3e-7);
t3777 = t2363.*(t2337+t12.*(t1456-t2355)).*(-1.02e-6);
t3779 = t2363.*(t2337+t12.*(t1456-t2355)).*9.3e-7;
t3780 = t2388.*(t2337+t12.*(t1456-t2355)).*(-1.02e-6);
t3784 = t2363.*(t2337+t12.*(t1456-t2355)).*(-9.0e-8);
t3785 = t2388.*(t2337+t12.*(t1456-t2355)).*1.02e-6;
t3787 = t2388.*(t2337+t12.*(t1456-t2355)).*(-9.0e-8);
t3788 = t2363.*(t2337+t12.*(t1456-t2355)).*9.0e-8;
t3793 = t2419.*(t2337+t12.*(t1456-t2355)).*(-1.02e-6);
t3794 = t2388.*(t2337+t12.*(t1456-t2355)).*9.0e-8;
t3796 = t2419.*(t2337+t12.*(t1456-t2355)).*1.02e-6;
t3800 = t2419.*(t2337+t12.*(t1456-t2355)).*(-9.0e-8);
t3802 = t2419.*(t2337+t12.*(t1456-t2355)).*9.0e-8;
t3812 = (t1477-t2502).*(t2801-t2850);
t3856 = (t2337+t12.*(t1456-t2355)).*(t1477-t2502).*1.02e-6;
t3863 = (t2337+t12.*(t1456-t2355)).*(t1477-t2502).*9.0e-8;
t3913 = t1880+t3122+t3277;
t3915 = t1902+t3121+t3276;
t3916 = -t10.*(-t1881+t3121+t3276);
t3918 = -t15.*(-t1881+t3121+t3276);
t3921 = -t11.*(-t1901+t3122+t3277);
t3923 = -t16.*(-t1901+t3122+t3277);
t3927 = t11.*(-t1901+t3122+t3277).*(-3.0./5.0e+2);
t3931 = t1943+t3137+t3313;
t3936 = t1955+t3138+t3315;
t3937 = t1958+t3138+t3315;
t3938 = t1972+t3137+t3313;
t3955 = t16.*(-t1901+t3122+t3277).*(-1.247162e-2);
t3956 = t10.*(-t1881+t3121+t3276).*(-5.84482e-3);
t3961 = t16.*(-t1901+t3122+t3277).*1.247162e-2;
t3963 = t11.*(-t1901+t3122+t3277).*(-5.68686e-3);
t3964 = t10.*(-t1881+t3121+t3276).*(-6.48e-5);
t3965 = t10.*(-t1881+t3121+t3276).*5.84482e-3;
t3968 = t10.*(-t1881+t3121+t3276).*6.48e-5;
t3969 = t15.*(-t1881+t3121+t3276).*(-6.47e-6);
t3972 = t11.*(-t1901+t3122+t3277).*(-3.131399999999998e-4);
t4130 = -t11.*((t237.*(t42-t43))./9.007199254740992e+15+t15.*(-t1881+t3121+t3276));
t4132 = -t16.*((t237.*(t42-t43))./9.007199254740992e+15+t15.*(-t1881+t3121+t3276));
t4137 = -t12.*(t951+t10.*(-t1881+t3121+t3276));
t4138 = -t17.*(t951+t10.*(-t1881+t3121+t3276));
t4141 = t16.*((t237.*(t42-t43))./9.007199254740992e+15+t15.*(-t1881+t3121+t3276));
t4142 = t17.*(t951+t10.*(-t1881+t3121+t3276));
t4149 = t1004+t3945;
t4152 = t1026+t3944;
t4194 = t11.*((t237.*(t42-t43))./9.007199254740992e+15+t15.*(-t1881+t3121+t3276)).*(-1.247162e-2);
t4196 = t12.*(t951+t10.*(-t1881+t3121+t3276)).*(-9.99471e-3);
t4198 = t11.*((t237.*(t42-t43))./9.007199254740992e+15+t15.*(-t1881+t3121+t3276)).*1.247162e-2;
t4212 = t123.*t188.*(t2694-t2701+t3036-t3043).*(-2.442490654175345e-23);
t4220 = t4177.*(-9.99471e-3);
t4223 = t4177.*9.99471e-3;
t4250 = t4177.*(-7.26350557185e-5);
t4252 = t50.*t123.*t189.*(t2694-t2701+t3036-t3043).*(-2.711709361697228e-39);
t4256 = t4177.*7.26350557185e-5;
t4261 = (t3499.*t3523)./2.0;
t4287 = (t3327.*t3809)./2.0;
t4468 = (t3533.*t3901)./2.0;
t4558 = (t3533.*t4008)./2.0;
t4644 = (t3320.*t4274)./2.0;
t4665 = -t4664;
t4677 = (t3837.*t3897)./2.0;
t4678 = (t3320.*t4324)./2.0;
t4679 = (t3838.*t3898)./2.0;
t4703 = (t3875.*t3901)./2.0;
t4713 = (t3767.*t4274)./2.0;
t4721 = (t3875.*t4008)./2.0;
t4724 = (t3880.*t4008)./2.0;
t4728 = (t3806.*t4313)./2.0;
t4740 = (t3767.*t4324)./2.0;
t4760 = (t3805.*t4324)./2.0;
t4828 = (t3897.*t4154)./2.0;
t4831 = (t3898.*t4153)./2.0;
t4895 = (t3879.*t4313)./2.0;
t4915 = t2346+t2382+t3169+t3174+t3382+t3384;
t4920 = t2345+t2408+t3168+t3176+t3381+t3388;
t4923 = (t3901.*t4275)./2.0;
t4924 = (t3903.*t4274)./2.0;
t5283 = -t5282;
t5302 = t3369.*t3638.*(t2674-t2676+t3022-t3027).*(t2694-t2701+t3036-t3043).*1.444822e-2;
t5304 = t3322.*t3649.*(t2674-t2676+t3022-t3027).*(t2694-t2701+t3036-t3043).*1.444822e-2;
t5392 = -t5391;
t5393 = t236.*t241.*t4349.*t4705.*2.156487945535858e-75;
t5397 = -t5395;
t5399 = t236.*t241.*t4351.*t4705.*1.16903445774439e-94;
t5400 = t236.*t241.*t4375.*t4705.*2.156487945535858e-75;
t5403 = -t5402;
t5436 = -t5435;
t5438 = t236.*t241.*t4349.*t4763.*2.394182569460511e-91;
t5452 = -t5450;
t5456 = t236.*t241.*t4351.*t4763.*1.297888971568006e-110;
t5458 = t236.*t241.*t4375.*t4763.*2.394182569460511e-91;
t5460 = -t5459;
t5464 = -t5463;
t5482 = -t5481;
t5537 = t236.*t241.*t4502.*t4763.*2.658076613771277e-107;
t5544 = t236.*t241.*t4349.*t5025.*1.16903445774439e-94;
t5548 = t236.*t241.*t4351.*t5025.*6.337348493984406e-114;
t5569 = t236.*t241.*t4709.*t4763.*1.297888971568006e-110;
t5586 = t236.*t241.*t4502.*t5025.*1.297888971568006e-110;
t5607 = -t5604;
t5678 = t236.*t241.*t4709.*t5025.*6.337348493984406e-114;
t5693 = t2125+t2142+t2750+t2762+t2796+t2811+t2812+t3210+t3470+t4044+t4055;
et9 = -t2125-t2142+t2745-t2750+t2774+t2785+t2786-t3470+t4038+t26.*(t1941-t3315+t39.*t1022.*(t855-t878).*2.196325630278387e-1).*1.869599668e-7;
et10 = t38.*t1022.*(t855-t878).*1.46680315462752e-4;
t5990 = (t3638.*(et9+et10).*(t2674-t2676+t3022-t3027))./2.0;
t6622 = (t5541.*t6011)./2.0;
et11 = t707+t708-t721-t722-t749+t762+t768-t777-t792-t793-t801-t802-t808+t813-t819+t821-t1629+t1637-t1640-t1641-t1659-t1661+t1666+t1667+t1683+t1692+t1705-t1712+t1758+t1759+t1775+t1776+t1973+t1993+t1994+t2023+t2053+t2060-t2089-t2090+t2098+t2099-t8.*t9.*t15.*t50.*t189.*3.670836568391568e-22;
et12 = t10.*t13.*t14.*t50.*t189.*(-3.279367663374749e-19)-t8.*t9.*t11.*t15.*t50.*t189.*7.075931802640439e-19;
et13 = t8.*t11.*t14.*t15.*t50.*t189.*(-1.190170786299927e-18)-t9.*t11.*t13.*t15.*t50.*t189.*1.190170786299927e-18;
et14 = t13.*t14.*t15.*t16.*t50.*t189.*(-3.226512155691387e-19);
t6623 = t5540.*(et11+et12+et13+et14).*(-1.0./2.0);
t6745 = (t5279.*t6255)./2.0;
et15 = t1288+t1289+t1302+t1303-t1319-t1320+t1336-t1348+t1350+t1351-t1360+t1369-t1378+t1396-t1425+t1435-t2174+t2183-t2187+t2193-t2194-t2195+t2199-t2203-t2215+t2219-t2222-t2223+t2239+t2240-t2256-t2257+t2555+t2556+t2572+t2583-t2605-t2606+t2612+t2613-t2618-t2619+t2651+t2652;
et16 = t18.*t19.*t20.*t50.*t202.*(-3.566935413776081e-21);
tau_c = ft_7({dq1,dq2,dq3,dq4,dq5,dq6,et15,et16,t10,t1000,t1002,t1003,t1005,t1006,t1015,t1018,t1020,t1022,t1023,t1035,t1040,t1044,t1045,t1046,t1048,t1049,t1050,t1051,t1058,t1063,t1065,t1067,t1068,t1071,t1083,t1084,t1089,t1093,t11,t1104,t1105,t1108,t1115,t1121,t1158,t1159,t1190,t1193,t1194,t1196,t12,t1205,t1207,t1208,t1210,t1212,t1214,t1217,t1218,t1219,t1220,t1221,t1222,t123,t1230,t1235,t1236,t1237,t1238,t1288,t1289,t13,t1302,t1303,t1319,t1320,t1336,t1348,t1350,t1351,t1360,t1369,t1378,t1396,t14,t140,t1425,t1435,t1456,t1477,t1488,t1492,t1493,t1494,t15,t1504,t1505,t1513,t1514,t1515,t1516,t1522,t1526,t1527,t1529,t1538,t1539,t1543,t1544,t1545,t1546,t1547,t1548,t1549,t1550,t1553,t1554,t1558,t1559,t1564,t1565,t1576,t1577,t1578,t1579,t1581,t1584,t1585,t1586,t1587,t1591,t1595,t1596,t1598,t1599,t16,t1600,t1601,t1602,t1604,t1605,t1606,t1607,t1608,t1609,t1612,t1613,t1614,t1615,t1616,t1626,t1627,t1628,t1629,t1631,t1637,t1640,t1641,t1648,t1649,t1659,t1660,t1661,t1666,t1667,t1683,t1686,t1690,t1692,t17,t1700,t1701,t1703,t1704,t1705,t1712,t1717,t1738,t1741,t1742,t1750,t1752,t1753,t1754,t1758,t1759,t1775,t1776,t18,t1860,t1861,t1864,t1865,t1868,t1870,t1874,t1876,t1879,t188,t1881,t1882,t1884,t1886,t1888,t1889,t189,t1890,t1893,t1896,t19,t1900,t1901,t1903,t1905,t1906,t1911,t1912,t1913,t1918,t1923,t1926,t1927,t1930,t1931,t1933,t1941,t1945,t1946,t1948,t1951,t1952,t1953,t1954,t1956,t1957,t1959,t1962,t1963,t1964,t1966,t1969,t1971,t1973,t1978,t1992,t1993,t1994,t1998,t20,t2004,t201,t202,t2023,t2024,t2028,t2053,t2060,t2073,t2089,t2090,t2098,t2099,t21,t2117,t2120,t2122,t2123,t2125,t2130,t2132,t2135,t2137,t2138,t2139,t2140,t2141,t2142,t2145,t2146,t2147,t2149,t2150,t2151,t2152,t2153,t2154,t2155,t2156,t2157,t2159,t2160,t2162,t2164,t2165,t2166,t2167,t2168,t2169,t2170,t2173,t2174,t2183,t2187,t2193,t2194,t2195,t2199,t22,t2203,t2215,t2219,t2222,t2223,t2239,t2240,t2256,t2257,t2290,t2291,t2292,t2293,t2294,t2295,t2296,t2297,t2298,t2299,t2300,t2301,t2302,t2303,t2304,t2305,t2306,t2307,t2308,t2309,t2310,t2311,t2312,t2313,t2317,t2320,t2322,t2323,t2324,t2325,t2326,t2327,t2328,t2329,t2335,t2336,t2337,t2338,t2339,t2341,t2342,t2343,t2344,t2351,t2352,t2353,t2354,t2355,t2357,t2358,t2359,t236,t2360,t2361,t2362,t2363,t2364,t2365,t2366,t2367,t2368,t2369,t237,t2370,t2371,t2374,t2375,t2377,t2378,t2379,t238,t2380,t2381,t2384,t2385,t2386,t2388,t2389,t2391,t2393,t2394,t2395,t2396,t2397,t2398,t2399,t24,t2400,t2401,t2402,t2403,t2404,t2405,t241,t2410,t2412,t2413,t2414,t2419,t2421,t2422,t2423,t2424,t2433,t2434,t2438,t2445,t2447,t2448,t2449,t2450,t2459,t2460,t2461,t2465,t2468,t2470,t2471,t2472,t2492,t2493,t2494,t2497,t25,t2500,t2501,t2502,t2506,t2507,t2508,t2509,t2510,t2515,t2517,t2520,t2523,t2525,t2527,t2529,t2530,t2531,t2532,t2533,t2534,t2535,t2536,t2537,t2539,t2547,t2553,t2555,t2556,t2572,t2575,t2583,t26,t2602,t2605,t2606,t2612,t2613,t2615,t2618,t2619,t262,t2636,t2638,t264,t2651,t2652,t2663,t2664,t2670,t2671,t2672,t2673,t2674,t2675,t2676,t2677,t2678,t2679,t2680,t2681,t2682,t2683,t2684,t2685,t2686,t2687,t2689,t2690,t2691,t2692,t2693,t2694,t2695,t2696,t2697,t2698,t27,t2700,t2701,t2702,t2703,t2704,t2705,t2707,t2708,t2709,t2711,t2712,t2713,t2715,t2716,t2717,t2719,t2720,t2721,t2732,t2733,t2735,t2736,t2737,t2738,t2739,t2740,t2742,t2743,t2744,t2745,t2746,t2747,t2748,t2749,t2750,t2751,t2752,t2753,t2754,t2755,t2756,t2757,t2759,t2760,t2761,t2764,t2765,t2768,t2769,t2770,t2773,t2774,t2775,t2776,t2777,t2778,t2779,t2781,t2784,t2785,t2786,t2787,t2788,t2789,t2790,t2791,t2792,t2793,t2795,t2797,t2798,t2799,t28,t2801,t2802,t2803,t2804,t2805,t2806,t2807,t2808,t2810,t2813,t2814,t2815,t2816,t2817,t2818,t2819,t2820,t2821,t2822,t2823,t2824,t2826,t2827,t2828,t2829,t2830,t2831,t2832,t2833,t2834,t2835,t2836,t2837,t2838,t2839,t2840,t2843,t2844,t2845,t2846,t2847,t2848,t2850,t2851,t2852,t2854,t2855,t2856,t2861,t2864,t2866,t2869,t2871,t2873,t2874,t2877,t2878,t2881,t2882,t2885,t2888,t2889,t2897,t29,t2902,t2909,t2927,t2928,t2929,t2932,t2934,t2936,t2937,t2941,t2942,t2945,t2946,t2947,t2948,t2950,t2951,t2953,t2954,t2955,t2956,t2957,t2961,t2962,t2963,t2964,t2965,t2966,t2969,t2970,t2971,t2972,t2973,t2975,t2976,t2977,t2978,t2979,t2981,t2982,t2984,t2985,t2986,t2987,t2990,t2991,t2992,t2993,t2998,t30,t3001,t3002,t3004,t3006,t3008,t3010,t3013,t3014,t3015,t3016,t3017,t3018,t3019,t3022,t3024,t3025,t3027,t3028,t3029,t3030,t3031,t3036,t3038,t3039,t3043,t3044,t3045,t3046,t3047,t3049,t3050,t3051,t3052,t3053,t3054,t3055,t3057,t3058,t3060,t3061,t3064,t3065,t3066,t3067,t3068,t3069,t3072,t3073,t3074,t3075,t3076,t3077,t3078,t3079,t3080,t3081,t3082,t3083,t3085,t3086,t3087,t3088,t3092,t3093,t3094,t3095,t3096,t3097,t31,t3101,t3102,t3103,t3106,t3107,t3108,t3109,t3113,t3115,t3117,t3119,t3120,t3121,t3122,t3123,t3124,t3125,t3126,t3127,t3129,t313,t3130,t3131,t3132,t3134,t3135,t3136,t314,t3140,t3141,t3142,t3145,t3146,t3147,t3148,t3149,t3150,t3151,t3152,t3153,t3154,t3155,t3157,t3158,t3159,t3160,t3161,t3162,t3163,t3164,t3165,t3166,t3171,t3172,t3173,t3179,t3180,t3182,t3183,t3184,t3186,t3188,t3191,t3193,t3194,t3195,t32,t3202,t3205,t3207,t3208,t321,t3211,t3212,t3213,t3215,t3216,t322,t3225,t3235,t3236,t326,t3266,t3268,t3269,t3270,t3273,t3274,t3275,t3276,t3277,t328,t329,t33,t330,t331,t3313,t3315,t3318,t3319,t332,t3321,t3322,t3323,t333,t335,t336,t3369,t3371,t3372,t3374,t3375,t3377,t3379,t338,t3380,t3387,t339,t3393,t3394,t34,t341,t3429,t343,t3435,t3438,t3443,t3447,t3449,t3454,t346,t3460,t3461,t3465,t3469,t3470,t3471,t3472,t3473,t3484,t3486,t3488,t3491,t3494,t3499,t35,t350,t351,t3517,t352,t354,t3545,t3552,t356,t3579,t358,t359,t36,t360,t362,t363,t3638,t364,t3649,t365,t366,t369,t3693,t3696,t3699,t370,t371,t3712,t372,t3755,t3777,t3779,t378,t3784,t3785,t3788,t3793,t3794,t3796,t38,t380,t3800,t3802,t3805,t3809,t3812,t382,t3856,t3863,t387,t3876,t3877,t3878,t3879,t3880,t3897,t3898,t39,t3901,t3902,t3903,t3913,t3915,t3916,t3918,t3921,t3923,t3927,t3931,t3937,t3947,t3948,t3950,t3955,t3961,t3963,t3964,t3965,t3968,t3969,t3972,t3974,t3989,t3990,t3994,t4000,t4004,t4005,t4008,t4035,t4038,t4040,t4043,t4050,t4057,t410,t4130,t4137,t4141,t4142,t4147,t4149,t4153,t4154,t4167,t4177,t4194,t4196,t4198,t42,t4212,t4222,t4223,t4232,t4234,t4252,t4255,t4256,t4260,t4261,t4273,t4274,t4275,t4287,t429,t43,t4313,t4314,t4324,t4325,t4326,t4334,t4343,t4348,t4375,t4421,t4424,t4468,t4476,t4501,t4502,t4558,t4563,t46,t4644,t4652,t4663,t4665,t4677,t4678,t4679,t4683,t47,t4703,t4704,t4705,t4708,t4709,t4713,t4716,t4721,t4724,t4728,t4730,t4740,t4760,t4762,t4763,t4828,t4831,t4847,t4850,t4895,t4902,t4915,t4920,t4923,t4924,t50,t5025,t5027,t5036,t5037,t516,t522,t523,t524,t5278,t5279,t528,t5283,t5296,t530,t5302,t5304,t5308,t5309,t5361,t5363,t5370,t5372,t5381,t5391,t5392,t5393,t5395,t5399,t5400,t5402,t5403,t5404,t542,t543,t5433,t5434,t5436,t5437,t5438,t5439,t5452,t5456,t5457,t5458,t5459,t5460,t5464,t5481,t549,t5499,t5537,t5540,t5541,t5542,t5544,t5545,t5548,t5550,t5569,t5570,t5586,t56,t5604,t5607,t562,t563,t5678,t5684,t575,t5782,t5783,t58,t580,t587,t59,t5901,t5902,t594,t5990,t60,t6011,t6013,t6014,t610,t612,t6255,t6256,t6257,t628,t635,t636,t638,t640,t641,t642,t643,t644,t645,t646,t648,t649,t654,t655,t656,t657,t659,t660,t6622,t6623,t663,t664,t665,t666,t667,t668,t669,t67,t670,t672,t673,t674,t6745,t675,t676,t677,t678,t679,t68,t681,t682,t683,t684,t685,t686,t687,t689,t691,t692,t693,t694,t70,t702,t707,t708,t71,t710,t715,t716,t717,t718,t721,t722,t724,t725,t73,t736,t738,t740,t741,t749,t756,t76,t762,t768,t777,t792,t793,t8,t801,t802,t808,t813,t819,t821,t850,t855,t874,t878,t89,t9,t90,t91,t92,t941,t944,t945,t948,t949,t950,t951,t97,t974,t983,t989,t996});
end
function tau_c = ft_7(ct)
dq1 = ct{1};
dq2 = ct{2};
dq3 = ct{3};
dq4 = ct{4};
dq5 = ct{5};
dq6 = ct{6};
et15 = ct{7};
et16 = ct{8};
t10 = ct{9};
t1000 = ct{10};
t1002 = ct{11};
t1003 = ct{12};
t1005 = ct{13};
t1006 = ct{14};
t1015 = ct{15};
t1018 = ct{16};
t1020 = ct{17};
t1022 = ct{18};
t1023 = ct{19};
t1035 = ct{20};
t1040 = ct{21};
t1044 = ct{22};
t1045 = ct{23};
t1046 = ct{24};
t1048 = ct{25};
t1049 = ct{26};
t1050 = ct{27};
t1051 = ct{28};
t1058 = ct{29};
t1063 = ct{30};
t1065 = ct{31};
t1067 = ct{32};
t1068 = ct{33};
t1071 = ct{34};
t1083 = ct{35};
t1084 = ct{36};
t1089 = ct{37};
t1093 = ct{38};
t11 = ct{39};
t1104 = ct{40};
t1105 = ct{41};
t1108 = ct{42};
t1115 = ct{43};
t1121 = ct{44};
t1158 = ct{45};
t1159 = ct{46};
t1190 = ct{47};
t1193 = ct{48};
t1194 = ct{49};
t1196 = ct{50};
t12 = ct{51};
t1205 = ct{52};
t1207 = ct{53};
t1208 = ct{54};
t1210 = ct{55};
t1212 = ct{56};
t1214 = ct{57};
t1217 = ct{58};
t1218 = ct{59};
t1219 = ct{60};
t1220 = ct{61};
t1221 = ct{62};
t1222 = ct{63};
t123 = ct{64};
t1230 = ct{65};
t1235 = ct{66};
t1236 = ct{67};
t1237 = ct{68};
t1238 = ct{69};
t1288 = ct{70};
t1289 = ct{71};
t13 = ct{72};
t1302 = ct{73};
t1303 = ct{74};
t1319 = ct{75};
t1320 = ct{76};
t1336 = ct{77};
t1348 = ct{78};
t1350 = ct{79};
t1351 = ct{80};
t1360 = ct{81};
t1369 = ct{82};
t1378 = ct{83};
t1396 = ct{84};
t14 = ct{85};
t140 = ct{86};
t1425 = ct{87};
t1435 = ct{88};
t1456 = ct{89};
t1477 = ct{90};
t1488 = ct{91};
t1492 = ct{92};
t1493 = ct{93};
t1494 = ct{94};
t15 = ct{95};
t1504 = ct{96};
t1505 = ct{97};
t1513 = ct{98};
t1514 = ct{99};
t1515 = ct{100};
t1516 = ct{101};
t1522 = ct{102};
t1526 = ct{103};
t1527 = ct{104};
t1529 = ct{105};
t1538 = ct{106};
t1539 = ct{107};
t1543 = ct{108};
t1544 = ct{109};
t1545 = ct{110};
t1546 = ct{111};
t1547 = ct{112};
t1548 = ct{113};
t1549 = ct{114};
t1550 = ct{115};
t1553 = ct{116};
t1554 = ct{117};
t1558 = ct{118};
t1559 = ct{119};
t1564 = ct{120};
t1565 = ct{121};
t1576 = ct{122};
t1577 = ct{123};
t1578 = ct{124};
t1579 = ct{125};
t1581 = ct{126};
t1584 = ct{127};
t1585 = ct{128};
t1586 = ct{129};
t1587 = ct{130};
t1591 = ct{131};
t1595 = ct{132};
t1596 = ct{133};
t1598 = ct{134};
t1599 = ct{135};
t16 = ct{136};
t1600 = ct{137};
t1601 = ct{138};
t1602 = ct{139};
t1604 = ct{140};
t1605 = ct{141};
t1606 = ct{142};
t1607 = ct{143};
t1608 = ct{144};
t1609 = ct{145};
t1612 = ct{146};
t1613 = ct{147};
t1614 = ct{148};
t1615 = ct{149};
t1616 = ct{150};
t1626 = ct{151};
t1627 = ct{152};
t1628 = ct{153};
t1629 = ct{154};
t1631 = ct{155};
t1637 = ct{156};
t1640 = ct{157};
t1641 = ct{158};
t1648 = ct{159};
t1649 = ct{160};
t1659 = ct{161};
t1660 = ct{162};
t1661 = ct{163};
t1666 = ct{164};
t1667 = ct{165};
t1683 = ct{166};
t1686 = ct{167};
t1690 = ct{168};
t1692 = ct{169};
t17 = ct{170};
t1700 = ct{171};
t1701 = ct{172};
t1703 = ct{173};
t1704 = ct{174};
t1705 = ct{175};
t1712 = ct{176};
t1717 = ct{177};
t1738 = ct{178};
t1741 = ct{179};
t1742 = ct{180};
t1750 = ct{181};
t1752 = ct{182};
t1753 = ct{183};
t1754 = ct{184};
t1758 = ct{185};
t1759 = ct{186};
t1775 = ct{187};
t1776 = ct{188};
t18 = ct{189};
t1860 = ct{190};
t1861 = ct{191};
t1864 = ct{192};
t1865 = ct{193};
t1868 = ct{194};
t1870 = ct{195};
t1874 = ct{196};
t1876 = ct{197};
t1879 = ct{198};
t188 = ct{199};
t1881 = ct{200};
t1882 = ct{201};
t1884 = ct{202};
t1886 = ct{203};
t1888 = ct{204};
t1889 = ct{205};
t189 = ct{206};
t1890 = ct{207};
t1893 = ct{208};
t1896 = ct{209};
t19 = ct{210};
t1900 = ct{211};
t1901 = ct{212};
t1903 = ct{213};
t1905 = ct{214};
t1906 = ct{215};
t1911 = ct{216};
t1912 = ct{217};
t1913 = ct{218};
t1918 = ct{219};
t1923 = ct{220};
t1926 = ct{221};
t1927 = ct{222};
t1930 = ct{223};
t1931 = ct{224};
t1933 = ct{225};
t1941 = ct{226};
t1945 = ct{227};
t1946 = ct{228};
t1948 = ct{229};
t1951 = ct{230};
t1952 = ct{231};
t1953 = ct{232};
t1954 = ct{233};
t1956 = ct{234};
t1957 = ct{235};
t1959 = ct{236};
t1962 = ct{237};
t1963 = ct{238};
t1964 = ct{239};
t1966 = ct{240};
t1969 = ct{241};
t1971 = ct{242};
t1973 = ct{243};
t1978 = ct{244};
t1992 = ct{245};
t1993 = ct{246};
t1994 = ct{247};
t1998 = ct{248};
t20 = ct{249};
t2004 = ct{250};
t201 = ct{251};
t202 = ct{252};
t2023 = ct{253};
t2024 = ct{254};
t2028 = ct{255};
t2053 = ct{256};
t2060 = ct{257};
t2073 = ct{258};
t2089 = ct{259};
t2090 = ct{260};
t2098 = ct{261};
t2099 = ct{262};
t21 = ct{263};
t2117 = ct{264};
t2120 = ct{265};
t2122 = ct{266};
t2123 = ct{267};
t2125 = ct{268};
t2130 = ct{269};
t2132 = ct{270};
t2135 = ct{271};
t2137 = ct{272};
t2138 = ct{273};
t2139 = ct{274};
t2140 = ct{275};
t2141 = ct{276};
t2142 = ct{277};
t2145 = ct{278};
t2146 = ct{279};
t2147 = ct{280};
t2149 = ct{281};
t2150 = ct{282};
t2151 = ct{283};
t2152 = ct{284};
t2153 = ct{285};
t2154 = ct{286};
t2155 = ct{287};
t2156 = ct{288};
t2157 = ct{289};
t2159 = ct{290};
t2160 = ct{291};
t2162 = ct{292};
t2164 = ct{293};
t2165 = ct{294};
t2166 = ct{295};
t2167 = ct{296};
t2168 = ct{297};
t2169 = ct{298};
t2170 = ct{299};
t2173 = ct{300};
t2174 = ct{301};
t2183 = ct{302};
t2187 = ct{303};
t2193 = ct{304};
t2194 = ct{305};
t2195 = ct{306};
t2199 = ct{307};
t22 = ct{308};
t2203 = ct{309};
t2215 = ct{310};
t2219 = ct{311};
t2222 = ct{312};
t2223 = ct{313};
t2239 = ct{314};
t2240 = ct{315};
t2256 = ct{316};
t2257 = ct{317};
t2290 = ct{318};
t2291 = ct{319};
t2292 = ct{320};
t2293 = ct{321};
t2294 = ct{322};
t2295 = ct{323};
t2296 = ct{324};
t2297 = ct{325};
t2298 = ct{326};
t2299 = ct{327};
t2300 = ct{328};
t2301 = ct{329};
t2302 = ct{330};
t2303 = ct{331};
t2304 = ct{332};
t2305 = ct{333};
t2306 = ct{334};
t2307 = ct{335};
t2308 = ct{336};
t2309 = ct{337};
t2310 = ct{338};
t2311 = ct{339};
t2312 = ct{340};
t2313 = ct{341};
t2317 = ct{342};
t2320 = ct{343};
t2322 = ct{344};
t2323 = ct{345};
t2324 = ct{346};
t2325 = ct{347};
t2326 = ct{348};
t2327 = ct{349};
t2328 = ct{350};
t2329 = ct{351};
t2335 = ct{352};
t2336 = ct{353};
t2337 = ct{354};
t2338 = ct{355};
t2339 = ct{356};
t2341 = ct{357};
t2342 = ct{358};
t2343 = ct{359};
t2344 = ct{360};
t2351 = ct{361};
t2352 = ct{362};
t2353 = ct{363};
t2354 = ct{364};
t2355 = ct{365};
t2357 = ct{366};
t2358 = ct{367};
t2359 = ct{368};
t236 = ct{369};
t2360 = ct{370};
t2361 = ct{371};
t2362 = ct{372};
t2363 = ct{373};
t2364 = ct{374};
t2365 = ct{375};
t2366 = ct{376};
t2367 = ct{377};
t2368 = ct{378};
t2369 = ct{379};
t237 = ct{380};
t2370 = ct{381};
t2371 = ct{382};
t2374 = ct{383};
t2375 = ct{384};
t2377 = ct{385};
t2378 = ct{386};
t2379 = ct{387};
t238 = ct{388};
t2380 = ct{389};
t2381 = ct{390};
t2384 = ct{391};
t2385 = ct{392};
t2386 = ct{393};
t2388 = ct{394};
t2389 = ct{395};
t2391 = ct{396};
t2393 = ct{397};
t2394 = ct{398};
t2395 = ct{399};
t2396 = ct{400};
t2397 = ct{401};
t2398 = ct{402};
t2399 = ct{403};
t24 = ct{404};
t2400 = ct{405};
t2401 = ct{406};
t2402 = ct{407};
t2403 = ct{408};
t2404 = ct{409};
t2405 = ct{410};
t241 = ct{411};
t2410 = ct{412};
t2412 = ct{413};
t2413 = ct{414};
t2414 = ct{415};
t2419 = ct{416};
t2421 = ct{417};
t2422 = ct{418};
t2423 = ct{419};
t2424 = ct{420};
t2433 = ct{421};
t2434 = ct{422};
t2438 = ct{423};
t2445 = ct{424};
t2447 = ct{425};
t2448 = ct{426};
t2449 = ct{427};
t2450 = ct{428};
t2459 = ct{429};
t2460 = ct{430};
t2461 = ct{431};
t2465 = ct{432};
t2468 = ct{433};
t2470 = ct{434};
t2471 = ct{435};
t2472 = ct{436};
t2492 = ct{437};
t2493 = ct{438};
t2494 = ct{439};
t2497 = ct{440};
t25 = ct{441};
t2500 = ct{442};
t2501 = ct{443};
t2502 = ct{444};
t2506 = ct{445};
t2507 = ct{446};
t2508 = ct{447};
t2509 = ct{448};
t2510 = ct{449};
t2515 = ct{450};
t2517 = ct{451};
t2520 = ct{452};
t2523 = ct{453};
t2525 = ct{454};
t2527 = ct{455};
t2529 = ct{456};
t2530 = ct{457};
t2531 = ct{458};
t2532 = ct{459};
t2533 = ct{460};
t2534 = ct{461};
t2535 = ct{462};
t2536 = ct{463};
t2537 = ct{464};
t2539 = ct{465};
t2547 = ct{466};
t2553 = ct{467};
t2555 = ct{468};
t2556 = ct{469};
t2572 = ct{470};
t2575 = ct{471};
t2583 = ct{472};
t26 = ct{473};
t2602 = ct{474};
t2605 = ct{475};
t2606 = ct{476};
t2612 = ct{477};
t2613 = ct{478};
t2615 = ct{479};
t2618 = ct{480};
t2619 = ct{481};
t262 = ct{482};
t2636 = ct{483};
t2638 = ct{484};
t264 = ct{485};
t2651 = ct{486};
t2652 = ct{487};
t2663 = ct{488};
t2664 = ct{489};
t2670 = ct{490};
t2671 = ct{491};
t2672 = ct{492};
t2673 = ct{493};
t2674 = ct{494};
t2675 = ct{495};
t2676 = ct{496};
t2677 = ct{497};
t2678 = ct{498};
t2679 = ct{499};
t2680 = ct{500};
t2681 = ct{501};
t2682 = ct{502};
t2683 = ct{503};
t2684 = ct{504};
t2685 = ct{505};
t2686 = ct{506};
t2687 = ct{507};
t2689 = ct{508};
t2690 = ct{509};
t2691 = ct{510};
t2692 = ct{511};
t2693 = ct{512};
t2694 = ct{513};
t2695 = ct{514};
t2696 = ct{515};
t2697 = ct{516};
t2698 = ct{517};
t27 = ct{518};
t2700 = ct{519};
t2701 = ct{520};
t2702 = ct{521};
t2703 = ct{522};
t2704 = ct{523};
t2705 = ct{524};
t2707 = ct{525};
t2708 = ct{526};
t2709 = ct{527};
t2711 = ct{528};
t2712 = ct{529};
t2713 = ct{530};
t2715 = ct{531};
t2716 = ct{532};
t2717 = ct{533};
t2719 = ct{534};
t2720 = ct{535};
t2721 = ct{536};
t2732 = ct{537};
t2733 = ct{538};
t2735 = ct{539};
t2736 = ct{540};
t2737 = ct{541};
t2738 = ct{542};
t2739 = ct{543};
t2740 = ct{544};
t2742 = ct{545};
t2743 = ct{546};
t2744 = ct{547};
t2745 = ct{548};
t2746 = ct{549};
t2747 = ct{550};
t2748 = ct{551};
t2749 = ct{552};
t2750 = ct{553};
t2751 = ct{554};
t2752 = ct{555};
t2753 = ct{556};
t2754 = ct{557};
t2755 = ct{558};
t2756 = ct{559};
t2757 = ct{560};
t2759 = ct{561};
t2760 = ct{562};
t2761 = ct{563};
t2764 = ct{564};
t2765 = ct{565};
t2768 = ct{566};
t2769 = ct{567};
t2770 = ct{568};
t2773 = ct{569};
t2774 = ct{570};
t2775 = ct{571};
t2776 = ct{572};
t2777 = ct{573};
t2778 = ct{574};
t2779 = ct{575};
t2781 = ct{576};
t2784 = ct{577};
t2785 = ct{578};
t2786 = ct{579};
t2787 = ct{580};
t2788 = ct{581};
t2789 = ct{582};
t2790 = ct{583};
t2791 = ct{584};
t2792 = ct{585};
t2793 = ct{586};
t2795 = ct{587};
t2797 = ct{588};
t2798 = ct{589};
t2799 = ct{590};
t28 = ct{591};
t2801 = ct{592};
t2802 = ct{593};
t2803 = ct{594};
t2804 = ct{595};
t2805 = ct{596};
t2806 = ct{597};
t2807 = ct{598};
t2808 = ct{599};
t2810 = ct{600};
t2813 = ct{601};
t2814 = ct{602};
t2815 = ct{603};
t2816 = ct{604};
t2817 = ct{605};
t2818 = ct{606};
t2819 = ct{607};
t2820 = ct{608};
t2821 = ct{609};
t2822 = ct{610};
t2823 = ct{611};
t2824 = ct{612};
t2826 = ct{613};
t2827 = ct{614};
t2828 = ct{615};
t2829 = ct{616};
t2830 = ct{617};
t2831 = ct{618};
t2832 = ct{619};
t2833 = ct{620};
t2834 = ct{621};
t2835 = ct{622};
t2836 = ct{623};
t2837 = ct{624};
t2838 = ct{625};
t2839 = ct{626};
t2840 = ct{627};
t2843 = ct{628};
t2844 = ct{629};
t2845 = ct{630};
t2846 = ct{631};
t2847 = ct{632};
t2848 = ct{633};
t2850 = ct{634};
t2851 = ct{635};
t2852 = ct{636};
t2854 = ct{637};
t2855 = ct{638};
t2856 = ct{639};
t2861 = ct{640};
t2864 = ct{641};
t2866 = ct{642};
t2869 = ct{643};
t2871 = ct{644};
t2873 = ct{645};
t2874 = ct{646};
t2877 = ct{647};
t2878 = ct{648};
t2881 = ct{649};
t2882 = ct{650};
t2885 = ct{651};
t2888 = ct{652};
t2889 = ct{653};
t2897 = ct{654};
t29 = ct{655};
t2902 = ct{656};
t2909 = ct{657};
t2927 = ct{658};
t2928 = ct{659};
t2929 = ct{660};
t2932 = ct{661};
t2934 = ct{662};
t2936 = ct{663};
t2937 = ct{664};
t2941 = ct{665};
t2942 = ct{666};
t2945 = ct{667};
t2946 = ct{668};
t2947 = ct{669};
t2948 = ct{670};
t2950 = ct{671};
t2951 = ct{672};
t2953 = ct{673};
t2954 = ct{674};
t2955 = ct{675};
t2956 = ct{676};
t2957 = ct{677};
t2961 = ct{678};
t2962 = ct{679};
t2963 = ct{680};
t2964 = ct{681};
t2965 = ct{682};
t2966 = ct{683};
t2969 = ct{684};
t2970 = ct{685};
t2971 = ct{686};
t2972 = ct{687};
t2973 = ct{688};
t2975 = ct{689};
t2976 = ct{690};
t2977 = ct{691};
t2978 = ct{692};
t2979 = ct{693};
t2981 = ct{694};
t2982 = ct{695};
t2984 = ct{696};
t2985 = ct{697};
t2986 = ct{698};
t2987 = ct{699};
t2990 = ct{700};
t2991 = ct{701};
t2992 = ct{702};
t2993 = ct{703};
t2998 = ct{704};
t30 = ct{705};
t3001 = ct{706};
t3002 = ct{707};
t3004 = ct{708};
t3006 = ct{709};
t3008 = ct{710};
t3010 = ct{711};
t3013 = ct{712};
t3014 = ct{713};
t3015 = ct{714};
t3016 = ct{715};
t3017 = ct{716};
t3018 = ct{717};
t3019 = ct{718};
t3022 = ct{719};
t3024 = ct{720};
t3025 = ct{721};
t3027 = ct{722};
t3028 = ct{723};
t3029 = ct{724};
t3030 = ct{725};
t3031 = ct{726};
t3036 = ct{727};
t3038 = ct{728};
t3039 = ct{729};
t3043 = ct{730};
t3044 = ct{731};
t3045 = ct{732};
t3046 = ct{733};
t3047 = ct{734};
t3049 = ct{735};
t3050 = ct{736};
t3051 = ct{737};
t3052 = ct{738};
t3053 = ct{739};
t3054 = ct{740};
t3055 = ct{741};
t3057 = ct{742};
t3058 = ct{743};
t3060 = ct{744};
t3061 = ct{745};
t3064 = ct{746};
t3065 = ct{747};
t3066 = ct{748};
t3067 = ct{749};
t3068 = ct{750};
t3069 = ct{751};
t3072 = ct{752};
t3073 = ct{753};
t3074 = ct{754};
t3075 = ct{755};
t3076 = ct{756};
t3077 = ct{757};
t3078 = ct{758};
t3079 = ct{759};
t3080 = ct{760};
t3081 = ct{761};
t3082 = ct{762};
t3083 = ct{763};
t3085 = ct{764};
t3086 = ct{765};
t3087 = ct{766};
t3088 = ct{767};
t3092 = ct{768};
t3093 = ct{769};
t3094 = ct{770};
t3095 = ct{771};
t3096 = ct{772};
t3097 = ct{773};
t31 = ct{774};
t3101 = ct{775};
t3102 = ct{776};
t3103 = ct{777};
t3106 = ct{778};
t3107 = ct{779};
t3108 = ct{780};
t3109 = ct{781};
t3113 = ct{782};
t3115 = ct{783};
t3117 = ct{784};
t3119 = ct{785};
t3120 = ct{786};
t3121 = ct{787};
t3122 = ct{788};
t3123 = ct{789};
t3124 = ct{790};
t3125 = ct{791};
t3126 = ct{792};
t3127 = ct{793};
t3129 = ct{794};
t313 = ct{795};
t3130 = ct{796};
t3131 = ct{797};
t3132 = ct{798};
t3134 = ct{799};
t3135 = ct{800};
t3136 = ct{801};
t314 = ct{802};
t3140 = ct{803};
t3141 = ct{804};
t3142 = ct{805};
t3145 = ct{806};
t3146 = ct{807};
t3147 = ct{808};
t3148 = ct{809};
t3149 = ct{810};
t3150 = ct{811};
t3151 = ct{812};
t3152 = ct{813};
t3153 = ct{814};
t3154 = ct{815};
t3155 = ct{816};
t3157 = ct{817};
t3158 = ct{818};
t3159 = ct{819};
t3160 = ct{820};
t3161 = ct{821};
t3162 = ct{822};
t3163 = ct{823};
t3164 = ct{824};
t3165 = ct{825};
t3166 = ct{826};
t3171 = ct{827};
t3172 = ct{828};
t3173 = ct{829};
t3179 = ct{830};
t3180 = ct{831};
t3182 = ct{832};
t3183 = ct{833};
t3184 = ct{834};
t3186 = ct{835};
t3188 = ct{836};
t3191 = ct{837};
t3193 = ct{838};
t3194 = ct{839};
t3195 = ct{840};
t32 = ct{841};
t3202 = ct{842};
t3205 = ct{843};
t3207 = ct{844};
t3208 = ct{845};
t321 = ct{846};
t3211 = ct{847};
t3212 = ct{848};
t3213 = ct{849};
t3215 = ct{850};
t3216 = ct{851};
t322 = ct{852};
t3225 = ct{853};
t3235 = ct{854};
t3236 = ct{855};
t326 = ct{856};
t3266 = ct{857};
t3268 = ct{858};
t3269 = ct{859};
t3270 = ct{860};
t3273 = ct{861};
t3274 = ct{862};
t3275 = ct{863};
t3276 = ct{864};
t3277 = ct{865};
t328 = ct{866};
t329 = ct{867};
t33 = ct{868};
t330 = ct{869};
t331 = ct{870};
t3313 = ct{871};
t3315 = ct{872};
t3318 = ct{873};
t3319 = ct{874};
t332 = ct{875};
t3321 = ct{876};
t3322 = ct{877};
t3323 = ct{878};
t333 = ct{879};
t335 = ct{880};
t336 = ct{881};
t3369 = ct{882};
t3371 = ct{883};
t3372 = ct{884};
t3374 = ct{885};
t3375 = ct{886};
t3377 = ct{887};
t3379 = ct{888};
t338 = ct{889};
t3380 = ct{890};
t3387 = ct{891};
t339 = ct{892};
t3393 = ct{893};
t3394 = ct{894};
t34 = ct{895};
t341 = ct{896};
t3429 = ct{897};
t343 = ct{898};
t3435 = ct{899};
t3438 = ct{900};
t3443 = ct{901};
t3447 = ct{902};
t3449 = ct{903};
t3454 = ct{904};
t346 = ct{905};
t3460 = ct{906};
t3461 = ct{907};
t3465 = ct{908};
t3469 = ct{909};
t3470 = ct{910};
t3471 = ct{911};
t3472 = ct{912};
t3473 = ct{913};
t3484 = ct{914};
t3486 = ct{915};
t3488 = ct{916};
t3491 = ct{917};
t3494 = ct{918};
t3499 = ct{919};
t35 = ct{920};
t350 = ct{921};
t351 = ct{922};
t3517 = ct{923};
t352 = ct{924};
t354 = ct{925};
t3545 = ct{926};
t3552 = ct{927};
t356 = ct{928};
t3579 = ct{929};
t358 = ct{930};
t359 = ct{931};
t36 = ct{932};
t360 = ct{933};
t362 = ct{934};
t363 = ct{935};
t3638 = ct{936};
t364 = ct{937};
t3649 = ct{938};
t365 = ct{939};
t366 = ct{940};
t369 = ct{941};
t3693 = ct{942};
t3696 = ct{943};
t3699 = ct{944};
t370 = ct{945};
t371 = ct{946};
t3712 = ct{947};
t372 = ct{948};
t3755 = ct{949};
t3777 = ct{950};
t3779 = ct{951};
t378 = ct{952};
t3784 = ct{953};
t3785 = ct{954};
t3788 = ct{955};
t3793 = ct{956};
t3794 = ct{957};
t3796 = ct{958};
t38 = ct{959};
t380 = ct{960};
t3800 = ct{961};
t3802 = ct{962};
t3805 = ct{963};
t3809 = ct{964};
t3812 = ct{965};
t382 = ct{966};
t3856 = ct{967};
t3863 = ct{968};
t387 = ct{969};
t3876 = ct{970};
t3877 = ct{971};
t3878 = ct{972};
t3879 = ct{973};
t3880 = ct{974};
t3897 = ct{975};
t3898 = ct{976};
t39 = ct{977};
t3901 = ct{978};
t3902 = ct{979};
t3903 = ct{980};
t3913 = ct{981};
t3915 = ct{982};
t3916 = ct{983};
t3918 = ct{984};
t3921 = ct{985};
t3923 = ct{986};
t3927 = ct{987};
t3931 = ct{988};
t3937 = ct{989};
t3947 = ct{990};
t3948 = ct{991};
t3950 = ct{992};
t3955 = ct{993};
t3961 = ct{994};
t3963 = ct{995};
t3964 = ct{996};
t3965 = ct{997};
t3968 = ct{998};
t3969 = ct{999};
t3972 = ct{1000};
t3974 = ct{1001};
t3989 = ct{1002};
t3990 = ct{1003};
t3994 = ct{1004};
t4000 = ct{1005};
t4004 = ct{1006};
t4005 = ct{1007};
t4008 = ct{1008};
t4035 = ct{1009};
t4038 = ct{1010};
t4040 = ct{1011};
t4043 = ct{1012};
t4050 = ct{1013};
t4057 = ct{1014};
t410 = ct{1015};
t4130 = ct{1016};
t4137 = ct{1017};
t4141 = ct{1018};
t4142 = ct{1019};
t4147 = ct{1020};
t4149 = ct{1021};
t4153 = ct{1022};
t4154 = ct{1023};
t4167 = ct{1024};
t4177 = ct{1025};
t4194 = ct{1026};
t4196 = ct{1027};
t4198 = ct{1028};
t42 = ct{1029};
t4212 = ct{1030};
t4222 = ct{1031};
t4223 = ct{1032};
t4232 = ct{1033};
t4234 = ct{1034};
t4252 = ct{1035};
t4255 = ct{1036};
t4256 = ct{1037};
t4260 = ct{1038};
t4261 = ct{1039};
t4273 = ct{1040};
t4274 = ct{1041};
t4275 = ct{1042};
t4287 = ct{1043};
t429 = ct{1044};
t43 = ct{1045};
t4313 = ct{1046};
t4314 = ct{1047};
t4324 = ct{1048};
t4325 = ct{1049};
t4326 = ct{1050};
t4334 = ct{1051};
t4343 = ct{1052};
t4348 = ct{1053};
t4375 = ct{1054};
t4421 = ct{1055};
t4424 = ct{1056};
t4468 = ct{1057};
t4476 = ct{1058};
t4501 = ct{1059};
t4502 = ct{1060};
t4558 = ct{1061};
t4563 = ct{1062};
t46 = ct{1063};
t4644 = ct{1064};
t4652 = ct{1065};
t4663 = ct{1066};
t4665 = ct{1067};
t4677 = ct{1068};
t4678 = ct{1069};
t4679 = ct{1070};
t4683 = ct{1071};
t47 = ct{1072};
t4703 = ct{1073};
t4704 = ct{1074};
t4705 = ct{1075};
t4708 = ct{1076};
t4709 = ct{1077};
t4713 = ct{1078};
t4716 = ct{1079};
t4721 = ct{1080};
t4724 = ct{1081};
t4728 = ct{1082};
t4730 = ct{1083};
t4740 = ct{1084};
t4760 = ct{1085};
t4762 = ct{1086};
t4763 = ct{1087};
t4828 = ct{1088};
t4831 = ct{1089};
t4847 = ct{1090};
t4850 = ct{1091};
t4895 = ct{1092};
t4902 = ct{1093};
t4915 = ct{1094};
t4920 = ct{1095};
t4923 = ct{1096};
t4924 = ct{1097};
t50 = ct{1098};
t5025 = ct{1099};
t5027 = ct{1100};
t5036 = ct{1101};
t5037 = ct{1102};
t516 = ct{1103};
t522 = ct{1104};
t523 = ct{1105};
t524 = ct{1106};
t5278 = ct{1107};
t5279 = ct{1108};
t528 = ct{1109};
t5283 = ct{1110};
t5296 = ct{1111};
t530 = ct{1112};
t5302 = ct{1113};
t5304 = ct{1114};
t5308 = ct{1115};
t5309 = ct{1116};
t5361 = ct{1117};
t5363 = ct{1118};
t5370 = ct{1119};
t5372 = ct{1120};
t5381 = ct{1121};
t5391 = ct{1122};
t5392 = ct{1123};
t5393 = ct{1124};
t5395 = ct{1125};
t5399 = ct{1126};
t5400 = ct{1127};
t5402 = ct{1128};
t5403 = ct{1129};
t5404 = ct{1130};
t542 = ct{1131};
t543 = ct{1132};
t5433 = ct{1133};
t5434 = ct{1134};
t5436 = ct{1135};
t5437 = ct{1136};
t5438 = ct{1137};
t5439 = ct{1138};
t5452 = ct{1139};
t5456 = ct{1140};
t5457 = ct{1141};
t5458 = ct{1142};
t5459 = ct{1143};
t5460 = ct{1144};
t5464 = ct{1145};
t5481 = ct{1146};
t549 = ct{1147};
t5499 = ct{1148};
t5537 = ct{1149};
t5540 = ct{1150};
t5541 = ct{1151};
t5542 = ct{1152};
t5544 = ct{1153};
t5545 = ct{1154};
t5548 = ct{1155};
t5550 = ct{1156};
t5569 = ct{1157};
t5570 = ct{1158};
t5586 = ct{1159};
t56 = ct{1160};
t5604 = ct{1161};
t5607 = ct{1162};
t562 = ct{1163};
t563 = ct{1164};
t5678 = ct{1165};
t5684 = ct{1166};
t575 = ct{1167};
t5782 = ct{1168};
t5783 = ct{1169};
t58 = ct{1170};
t580 = ct{1171};
t587 = ct{1172};
t59 = ct{1173};
t5901 = ct{1174};
t5902 = ct{1175};
t594 = ct{1176};
t5990 = ct{1177};
t60 = ct{1178};
t6011 = ct{1179};
t6013 = ct{1180};
t6014 = ct{1181};
t610 = ct{1182};
t612 = ct{1183};
t6255 = ct{1184};
t6256 = ct{1185};
t6257 = ct{1186};
t628 = ct{1187};
t635 = ct{1188};
t636 = ct{1189};
t638 = ct{1190};
t640 = ct{1191};
t641 = ct{1192};
t642 = ct{1193};
t643 = ct{1194};
t644 = ct{1195};
t645 = ct{1196};
t646 = ct{1197};
t648 = ct{1198};
t649 = ct{1199};
t654 = ct{1200};
t655 = ct{1201};
t656 = ct{1202};
t657 = ct{1203};
t659 = ct{1204};
t660 = ct{1205};
t6622 = ct{1206};
t6623 = ct{1207};
t663 = ct{1208};
t664 = ct{1209};
t665 = ct{1210};
t666 = ct{1211};
t667 = ct{1212};
t668 = ct{1213};
t669 = ct{1214};
t67 = ct{1215};
t670 = ct{1216};
t672 = ct{1217};
t673 = ct{1218};
t674 = ct{1219};
t6745 = ct{1220};
t675 = ct{1221};
t676 = ct{1222};
t677 = ct{1223};
t678 = ct{1224};
t679 = ct{1225};
t68 = ct{1226};
t681 = ct{1227};
t682 = ct{1228};
t683 = ct{1229};
t684 = ct{1230};
t685 = ct{1231};
t686 = ct{1232};
t687 = ct{1233};
t689 = ct{1234};
t691 = ct{1235};
t692 = ct{1236};
t693 = ct{1237};
t694 = ct{1238};
t70 = ct{1239};
t702 = ct{1240};
t707 = ct{1241};
t708 = ct{1242};
t71 = ct{1243};
t710 = ct{1244};
t715 = ct{1245};
t716 = ct{1246};
t717 = ct{1247};
t718 = ct{1248};
t721 = ct{1249};
t722 = ct{1250};
t724 = ct{1251};
t725 = ct{1252};
t73 = ct{1253};
t736 = ct{1254};
t738 = ct{1255};
t740 = ct{1256};
t741 = ct{1257};
t749 = ct{1258};
t756 = ct{1259};
t76 = ct{1260};
t762 = ct{1261};
t768 = ct{1262};
t777 = ct{1263};
t792 = ct{1264};
t793 = ct{1265};
t8 = ct{1266};
t801 = ct{1267};
t802 = ct{1268};
t808 = ct{1269};
t813 = ct{1270};
t819 = ct{1271};
t821 = ct{1272};
t850 = ct{1273};
t855 = ct{1274};
t874 = ct{1275};
t878 = ct{1276};
t89 = ct{1277};
t9 = ct{1278};
t90 = ct{1279};
t91 = ct{1280};
t92 = ct{1281};
t941 = ct{1282};
t944 = ct{1283};
t945 = ct{1284};
t948 = ct{1285};
t949 = ct{1286};
t950 = ct{1287};
t951 = ct{1288};
t97 = ct{1289};
t974 = ct{1290};
t983 = ct{1291};
t989 = ct{1292};
t996 = ct{1293};
et17 = t24.*t25.*t26.*t50.*t202.*(-3.992732227073824e-24);
et18 = t18.*t19.*t26.*t27.*t50.*t202.*(-3.509445006623964e-21);
et19 = t21.*t24.*t25.*t26.*t50.*t202.*(-7.696420262413979e-21);
t6749 = t5278.*(et15+et16+et17+et18+et19).*(-1.0./2.0);
et20 = t1288+t1289+t1302+t1303-t1319-t1320+t1336-t1348+t1350+t1351-t1360+t1369-t1378+t1396-t1425+t1435-t2174+t2183-t2187+t2193-t2194-t2195+t2199-t2203-t2215+t2219-t2222-t2223+t2239+t2240-t2256-t2257+t2555+t2556+t2572+t2583-t2605-t2606+t2612+t2613-t2618-t2619+t2651+t2652;
et21 = t18.*t19.*t20.*t50.*t202.*(-3.566935413776081e-21);
et22 = t24.*t25.*t26.*t50.*t202.*(-3.992732227073824e-24);
et23 = t18.*t19.*t26.*t27.*t50.*t202.*(-3.509445006623964e-21);
et24 = t21.*t24.*t25.*t26.*t50.*t202.*(-7.696420262413979e-21);
t6751 = (t5278.*(et20+et21+et22+et23+et24))./2.0;
t6919 = (t5901.*t6011)./2.0;
et25 = t707+t708-t721-t722-t749+t762+t768-t777-t792-t793-t801-t802-t808+t813-t819+t821-t1629+t1637-t1640-t1641-t1659-t1661+t1666+t1667+t1683+t1692+t1705-t1712+t1758+t1759+t1775+t1776+t1973+t1993+t1994+t2023+t2053+t2060-t2089-t2090+t2098+t2099-t8.*t9.*t15.*t50.*t189.*3.670836568391568e-22;
et26 = t10.*t13.*t14.*t50.*t189.*(-3.279367663374749e-19)-t8.*t9.*t11.*t15.*t50.*t189.*7.075931802640439e-19;
et27 = t8.*t11.*t14.*t15.*t50.*t189.*(-1.190170786299927e-18)-t9.*t11.*t13.*t15.*t50.*t189.*1.190170786299927e-18;
et28 = t13.*t14.*t15.*t16.*t50.*t189.*(-3.226512155691387e-19);
t6920 = t5902.*(et25+et26+et27+et28).*(-1.0./2.0);
t6987 = (t5782.*t6255)./2.0;
et29 = t1288+t1289+t1302+t1303-t1319-t1320+t1336-t1348+t1350+t1351-t1360+t1369-t1378+t1396-t1425+t1435-t2174+t2183-t2187+t2193-t2194-t2195+t2199-t2203-t2215+t2219-t2222-t2223+t2239+t2240-t2256-t2257+t2555+t2556+t2572+t2583-t2605-t2606+t2612+t2613-t2618-t2619+t2651+t2652;
et30 = t18.*t19.*t20.*t50.*t202.*(-3.566935413776081e-21);
et31 = t24.*t25.*t26.*t50.*t202.*(-3.992732227073824e-24);
et32 = t18.*t19.*t26.*t27.*t50.*t202.*(-3.509445006623964e-21);
et33 = t21.*t24.*t25.*t26.*t50.*t202.*(-7.696420262413979e-21);
t6988 = t5783.*(et29+et30+et31+et32+et33).*(-1.0./2.0);
t2519 = -t2506;
t2598 = -t2553;
t2669 = -t2663;
t2763 = -t2746;
t2766 = -t2756;
t2772 = -t2760;
t2794 = -t2770;
t2809 = -t2784;
t2841 = -t2824;
t2842 = -t2826;
t2853 = -t2833;
t2862 = -t2847;
t2863 = -t2848;
t2876 = -t2852;
t2880 = -t2854;
t2904 = -t2861;
t2910 = -t2869;
t2912 = -t2873;
t2913 = -t2874;
t2916 = -t2882;
t2921 = -t2888;
t2938 = -t2928;
t2994 = t516+t2445;
t2995 = t12.*t2992;
t2996 = t17.*t2992;
t3003 = t522+t2533;
t3007 = t22.*t2998;
t3009 = t28.*t2998;
t3062 = t1550+t2615;
t3089 = t17.*t3047.*9.99471e-3;
t3090 = t12.*t3047.*1.838876e-2;
t3098 = t12.*t3047.*1.02e-6;
t3099 = t17.*t3047.*9.3e-7;
t3104 = t12.*t3047.*9.0e-8;
t3105 = t17.*t3047.*9.0e-8;
t3110 = t28.*t3055.*9.99471e-3;
t3111 = t22.*t3055.*1.838876e-2;
t3112 = t3061.*(-9.99471e-3);
t3114 = t3061.*(-1.838876e-2);
t3116 = t3061.*9.99471e-3;
t3118 = t3061.*1.838876e-2;
t3128 = t2351+t2424;
t3133 = t1956+t2827;
t3139 = t1969+t2828;
t3143 = t2497+t2537;
t3156 = t201.*t3047.*8.595599785252598e-9;
t3181 = t201.*t3047.*8.76751178095765e-7;
t3185 = t50.*t202.*t2992.*5.439528691468777e-23;
t3187 = t201.*t3047.*2.062943948460623e-7;
t3190 = t201.*t3047.*3.438239914101039e-8;
t3192 = t50.*t202.*t2992.*3.817213116820194e-24;
t3200 = -t3193;
t3201 = -t3194;
t3209 = -t3208;
t3217 = t2132+t3002;
t3218 = t2135+t3001;
t3219 = t50.*t202.*t3047.*9.543032792050485e-25;
t3221 = t10.*t3215;
t3222 = t11.*t3216;
t3223 = t15.*t3215;
t3224 = t16.*t3216;
t3237 = t2170+t3013;
t3238 = t2173+t3014;
t3239 = t20.*t3235;
t3240 = t21.*t3236;
t3241 = t26.*t3235;
t3242 = t27.*t3236;
t3259 = t50.*t202.*t3047.*9.733893447891495e-23;
t3260 = t17.*t50.*t202.*t3047.*8.875020496606951e-23;
t3261 = t50.*t202.*t3047.*5.439528691468777e-23;
t3263 = t50.*t202.*t3047.*2.290327870092116e-23;
t3267 = t50.*t202.*t3047.*3.817213116820194e-24;
t3271 = t12.*t50.*t202.*t3047.*8.588729512845436e-24;
t3272 = t17.*t50.*t202.*t3047.*8.588729512845436e-24;
t3324 = -t3321;
t3325 = -t3323;
t3326 = t2363.*t2992.*5.7e-7;
t3336 = t2363.*t2992.*4.0e-8;
t3370 = t2335+t3053;
t3376 = t2381+t3052;
t3383 = (t2363.*t3047)./1.0e+8;
t3386 = (t2388.*t3047)./1.0e+8;
t3392 = (t2419.*t3047)./1.0e+8;
t3395 = t2465+t3060;
t3396 = t2468+t3061;
t3397 = -t2363.*(t1545-t2615);
t3416 = t2363.*(t1545-t2615).*(-1.0./2.0);
t3426 = t50.*t202.*t3123.*9.733893447891495e-23;
t3432 = t50.*t202.*t3123.*8.588729512845436e-24;
t3433 = t2363.*t3047.*5.7e-7;
t3434 = t2363.*t3047.*1.02e-6;
t3437 = t2388.*t3047.*1.02e-6;
t3439 = t2363.*t3047.*2.4e-7;
t3446 = t2388.*t3047.*2.4e-7;
t3448 = t2363.*t3047.*4.0e-8;
t3452 = t2419.*t3047.*1.02e-6;
t3453 = t2388.*t3047.*4.0e-8;
t3455 = t2419.*t3047.*2.4e-7;
t3458 = t21.*t2363.*t3047.*(-1.02e-6);
t3462 = t2419.*t3047.*4.0e-8;
t3463 = t11.*t2297.*t3055.*5.1e-7;
t3464 = t11.*t2297.*t3055.*1.02e-6;
t3474 = t3473./2.0;
t3476 = t188.*t3236.*6.899985389504867e-8;
t3477 = t188.*t3235.*3.878758105047274e-8;
t3483 = t580+t1546+t1903+t2602;
t3489 = t2363.*t3123.*1.02e-6;
t3490 = -t3488;
t3492 = t2363.*t3123.*9.0e-8;
t3496 = -t3494;
t3536 = t50.*t189.*t3235.*4.306286555174926e-24;
t3539 = t50.*t189.*t3236.*7.660522649005482e-24;
t3585 = -t3579;
t3588 = t3579./2.0;
t3700 = t3047.*t3055.*1.02e-6;
t3701 = t3055.*(t1456-t2355).*(-1.02e-6);
t3702 = t3047.*(t1477-t2502).*(-1.02e-6);
t3705 = t12.*t3047.*t3055.*(-1.02e-6);
t3706 = t17.*t3047.*t3055.*(-9.3e-7);
t3709 = t12.*t3047.*t3055.*(-9.0e-8);
t3710 = t17.*t3047.*t3055.*(-9.0e-8);
t3757 = -t3055.*(t1953-t2828);
t3761 = t2981.*t3236;
t3762 = t3055.*(t1953-t2828);
t3790 = t3055.*t3123.*1.02e-6;
t3792 = t21.*t3777;
t3797 = t3055.*t3123.*9.0e-8;
t3798 = t21.*t3784;
t3808 = t1884+t1906+t2756+t2768;
t3810 = t1926+t1946+t2847+t2866;
t3814 = t1952+t2073+t2821+t2874;
t3817 = t3812./2.0;
t3819 = t1978+t2028+t2846+t2871;
t3831 = t3120.*t3236;
t3848 = t3055.*(t2337+t12.*(t1456-t2355)).*(-9.3e-7);
t3849 = t3055.*(t2337+t12.*(t1456-t2355)).*(-1.02e-6);
t3855 = t3055.*(t2337+t12.*(t1456-t2355)).*1.02e-6;
t3857 = t3055.*(t2337+t12.*(t1456-t2355)).*(-9.0e-8);
t3861 = t3166.*t3236;
t3862 = t3055.*(t2337+t12.*(t1456-t2355)).*9.0e-8;
t3881 = t3216.*t3236.*3.24e-6;
t3882 = t3216.*t3236.*3.11e-6;
t3892 = -t3055.*(t335-t1539-t2831+t2851);
t3894 = t3055.*(t335-t1539-t2831+t2851);
t3910 = t2672+t2679+t3025+t3028;
t3911 = t2676+t2677+t3024+t3027;
t3912 = t1881+t3124+t3274;
t3914 = t1901+t3125+t3275;
t3917 = t10.*t3913;
t3919 = t15.*t3913;
t3920 = t11.*t3915;
t3922 = t16.*t3915;
t3934 = t2691+t2703+t3039+t3046;
t3935 = t2701+t2702+t3038+t3043;
t3940 = t20.*t3931;
t3941 = t26.*t3931;
t3942 = t27.*t3937;
t3946 = t21.*t3937;
t4119 = t950+t3918;
t4123 = t974+t3916;
t4143 = t4141.*(-3.0./5.0e+2);
t4145 = t4141.*(3.0./5.0e+2);
t4146 = t2738+t2739+t3094+t3095;
t4155 = t27.*t4149;
t4160 = t2810+t2835+t3106+t3108;
t4161 = t2804+t2856+t3102+t3107;
t4162 = t2830+t2835+t3101+t3108;
t4163 = t2806+t2838+t3103+t3109;
t4165 = t21.*t4149;
t4197 = t4142.*(-1.838876e-2);
t4201 = t4141.*(-5.68686e-3);
t4203 = t4142.*1.838876e-2;
t4206 = t4141.*5.68686e-3;
t4209 = t4141.*(-3.131399999999998e-4);
t4211 = t4141.*3.131399999999998e-4;
t4231 = t50.*t189.*t3931.*4.306286555174926e-24;
t4233 = t50.*t189.*t3937.*7.660522649005482e-24;
t4263 = -t4261;
t4288 = -t4287;
t4328 = t2973.*t4149;
t4347 = t3166.*t3937;
t4365 = -t22.*t3055.*(t2813-t2835+t12.*(t1456-t2355).*1.02e-6+t17.*(t1456-t2355).*9.0e-8);
t4366 = -t28.*t3055.*(-t2804+t2838+t3109+t17.*(t1456-t2355).*9.3e-7);
t4369 = t22.*t3055.*(t2813-t2835+t12.*(t1456-t2355).*1.02e-6+t17.*(t1456-t2355).*9.0e-8).*(-1.0./2.0);
t4370 = t28.*t3055.*(-t2804+t2838+t3109+t17.*(t1456-t2355).*9.3e-7).*(-1.0./2.0);
t4372 = (t22.*t3055.*(t2813-t2835+t12.*(t1456-t2355).*1.02e-6+t17.*(t1456-t2355).*9.0e-8))./2.0;
t4373 = (t28.*t3055.*(-t2804+t2838+t3109+t17.*(t1456-t2355).*9.3e-7))./2.0;
t4377 = t3236.*t3915.*3.24e-6;
t4378 = t3236.*t3915.*3.11e-6;
t4381 = t3216.*(t2694-t2701+t3036-t3043).*(-1.1e-7);
t4382 = t3216.*(t2694-t2701+t3036-t3043).*(-3.24e-6);
t4384 = t3216.*(t2694-t2701+t3036-t3043).*1.1e-7;
t4385 = t3216.*(t2694-t2701+t3036-t3043).*(-3.11e-6);
t4387 = t3216.*(t2694-t2701+t3036-t3043).*3.24e-6;
t4389 = t3216.*(t2694-t2701+t3036-t3043).*3.11e-6;
t4390 = t3215.*(t2694-t2701+t3036-t3043).*(-5.0e-8);
t4391 = t3216.*(t2694-t2701+t3036-t3043).*(-5.0e-8);
t4392 = t3215.*(t2694-t2701+t3036-t3043).*(-1.6e-7);
t4393 = t3216.*(t1959-t3313+t38.*t1022.*(t855-t878).*2.196325630278387e-1).*(-3.11e-6);
t4395 = t3216.*(t1959-t3313+t38.*t1022.*(t855-t878).*2.196325630278387e-1).*(-3.24e-6);
t4398 = t3216.*(t2694-t2701+t3036-t3043).*5.0e-8;
t4401 = t3216.*(t1959-t3313+t38.*t1022.*(t855-t878).*2.196325630278387e-1).*3.11e-6;
t4402 = t3216.*(t1959-t3313+t38.*t1022.*(t855-t878).*2.196325630278387e-1).*3.24e-6;
t4410 = -t3142.*(t2813-t2835+t12.*(t1456-t2355).*1.02e-6+t17.*(t1456-t2355).*9.0e-8);
t4413 = t3142.*(t2813-t2835+t12.*(t1456-t2355).*1.02e-6+t17.*(t1456-t2355).*9.0e-8).*(-1.0./2.0);
t4415 = (t3142.*(t2813-t2835+t12.*(t1456-t2355).*1.02e-6+t17.*(t1456-t2355).*9.0e-8))./2.0;
t4437 = t3186+t3429+t3484;
t4469 = t1504+t1888+t2506+t2737+t2752+t3092+t3093;
t4559 = -t4558;
t4680 = -t4679;
t4706 = -t4703;
t4722 = -t4721;
t4725 = -t4724;
t4741 = -t4740;
t4744 = t3915.*(t2694-t2701+t3036-t3043).*(-1.1e-7);
t4746 = t3915.*(t2694-t2701+t3036-t3043).*(-3.24e-6);
t4749 = t3915.*(t2694-t2701+t3036-t3043).*1.1e-7;
t4750 = t3913.*(t2694-t2701+t3036-t3043).*(-5.0e-8);
t4751 = t3915.*(t2694-t2701+t3036-t3043).*(-3.11e-6);
t4754 = t3913.*(t2694-t2701+t3036-t3043).*(-1.6e-7);
t4755 = t3915.*(t2694-t2701+t3036-t3043).*3.24e-6;
t4756 = t3915.*(t2694-t2701+t3036-t3043).*3.11e-6;
t4757 = t3915.*(t2694-t2701+t3036-t3043).*(-5.0e-8);
t4759 = t3915.*(t2694-t2701+t3036-t3043).*5.0e-8;
t4761 = -t4760;
t4814 = t549+t1890+t1911+t1962+t2737+t2752+t2755+t2816+t3092+t3093;
t4833 = -t4831;
t4836 = t3923+t4130;
t4837 = t3921+t4141;
t4873 = t2306+t2317+t3147+t3152+t3372+t3374;
t4879 = t2305+t2336+t3146+t3149+t3371+t3375;
t4951 = t3127+t3182+t3183+t3207+t3486;
t5015 = t50.*t189.*t4915.*(t42-t43).*(-2.711709361697228e-39);
t5016 = t50.*t123.*t189.*t4920.*2.711709361697228e-39;
t5087 = t3216.*t4920.*1.1e-7;
t5091 = t3216.*t4920.*3.24e-6;
t5093 = t3216.*t4920.*3.11e-6;
t5096 = t3215.*t4920.*5.0e-8;
t5097 = t3216.*t4920.*5.0e-8;
t5098 = t3215.*t4920.*1.6e-7;
t5394 = -t5393;
t5401 = -t5400;
t5561 = t1549+t1565+t2327+t2328+t2357+t2375+t2377+t3151+t3380+t3965+t3969;
t5991 = -t5990;
t2997 = -t2996;
t3020 = t2996.*9.99471e-3;
t3021 = t2995.*1.838876e-2;
t3032 = t2995.*1.02e-6;
t3033 = t2996.*9.3e-7;
t3034 = t2995.*9.0e-8;
t3035 = t2996.*9.0e-8;
t3040 = t3009.*9.99471e-3;
t3041 = t3007.*1.838876e-2;
t3063 = t1058+t2863;
t3167 = t50.*t202.*t2994.*9.543032792050485e-25;
t3189 = -t3185;
t3196 = -t3190;
t3198 = t50.*t202.*t2994.*9.733893447891495e-23;
t3199 = t50.*t202.*t2994.*2.290327870092116e-23;
t3203 = t50.*t202.*t2994.*3.817213116820194e-24;
t3226 = t10.*t3218;
t3227 = t11.*t3217;
t3228 = t15.*t3218;
t3229 = t16.*t3217;
t3230 = t3222.*(3.0./5.0e+2);
t3231 = t3224.*(3.0./5.0e+2);
t3243 = t2412+t2995;
t3244 = t20.*t3238;
t3245 = t21.*t3237;
t3246 = t26.*t3238;
t3247 = t27.*t3237;
t3248 = -t3242;
t3250 = t3240.*(3.0./5.0e+2);
t3251 = t3242.*(3.0./5.0e+2);
t3256 = (t2363.*t2994)./1.0e+8;
t3257 = t2531+t3007;
t3258 = t2536+t3009;
t3265 = t12.*t3259;
t3278 = t3222.*1.247162e-2;
t3279 = t3224.*1.247162e-2;
t3280 = t3221.*5.84482e-3;
t3281 = t3223.*5.84482e-3;
t3285 = t3222.*5.68686e-3;
t3286 = t3224.*5.68686e-3;
t3287 = t3221.*6.48e-5;
t3290 = t3223.*6.48e-5;
t3303 = t3222.*3.131399999999998e-4;
t3304 = t3224.*3.131399999999998e-4;
t3306 = t3221.*6.47e-6;
t3307 = t3223.*6.47e-6;
t3328 = t3240.*1.247162e-2;
t3329 = t3242.*1.247162e-2;
t3330 = t3239.*5.84482e-3;
t3331 = t3241.*5.84482e-3;
t3337 = t3239.*6.48e-5;
t3340 = t3241.*6.48e-5;
t3343 = t2363.*t2994.*1.02e-6;
t3344 = t3242.*3.131399999999998e-4;
t3345 = t2363.*t2994.*2.4e-7;
t3351 = t3240.*3.131399999999998e-4;
t3354 = t2363.*t2994.*4.0e-8;
t3356 = t3239.*6.47e-6;
t3357 = t3241.*6.47e-6;
t3358 = t3240.*4.36041e-5;
t3359 = t3242.*4.36041e-5;
t3389 = -t3386;
t3398 = t3240.*1.35652563578e-4;
t3399 = t3242.*1.35652563578e-4;
t3400 = t3239.*1.688944904408e-4;
t3401 = t3241.*1.688944904408e-4;
t3402 = t3240.*6.1855407534e-5;
t3403 = t3242.*6.1855407534e-5;
t3412 = t3239.*7.0482312e-7;
t3413 = t3241.*7.0482312e-7;
t3417 = t3239.*1.869599668e-7;
t3418 = t3241.*1.869599668e-7;
t3428 = t50.*t202.*t3128.*8.875020496606951e-23;
t3431 = t648+t1048+t1522+t2669;
t3436 = t50.*t202.*t3128.*8.588729512845436e-24;
t3440 = t2363.*t3098;
t3441 = t2363.*t3099;
t3445 = -t3437;
t3450 = t21.*t3434;
t3451 = -t3446;
t3456 = t2363.*t3104;
t3457 = t2363.*t3105;
t3467 = -t3464;
t3468 = -t3463;
t3475 = t21.*t2363.*t3133;
t3478 = t188.*t3237.*6.899985389504867e-8;
t3479 = t188.*t3238.*3.878758105047274e-8;
t3493 = t2363.*t3128.*9.3e-7;
t3497 = t2363.*t3128.*9.0e-8;
t3500 = t1860+t3223;
t3501 = t1864+t3221;
t3508 = -t12.*(t1861-t3221);
t3509 = -t17.*(t1861-t3221);
t3524 = t12.*t16.*(t1861-t3221);
t3530 = t16.*(t1861-t3221).*(-3.0./5.0e+2);
t3538 = t50.*t189.*t3238.*4.306286555174926e-24;
t3540 = t50.*t189.*t3237.*7.660522649005482e-24;
t3541 = t201.*t3370.*7.993907800284916e-7;
t3543 = t1893+t3241;
t3544 = t1912+t3239;
t3546 = t201.*t3370.*7.736039806727338e-8;
t3559 = -t22.*(t1896-t3239);
t3560 = -t28.*(t1896-t3239);
t3566 = t22.*(t1896-t3239);
t3577 = t2994.*t3055.*1.02e-6;
t3578 = t3003.*t3047.*1.02e-6;
t3580 = t27.*(t1896-t3239).*(-3.0./5.0e+2);
t3590 = -t3588;
t3597 = t12.*(t1861-t3221).*(-9.99471e-3);
t3598 = t17.*(t1861-t3221).*(-9.99471e-3);
t3599 = t12.*(t1861-t3221).*(-1.838876e-2);
t3600 = t17.*(t1861-t3221).*(-1.838876e-2);
t3602 = t11.*(t1861-t3221).*(-1.247162e-2);
t3604 = t16.*(t1861-t3221).*(-5.68686e-3);
t3605 = t12.*(t1861-t3221).*9.99471e-3;
t3609 = t17.*(t1861-t3221).*1.838876e-2;
t3611 = t11.*(t1861-t3221).*1.247162e-2;
t3628 = t16.*(t1861-t3221).*(-3.131399999999998e-4);
t3644 = t28.*(t1896-t3239).*(-9.99471e-3);
t3646 = t28.*(t1896-t3239).*(-1.838876e-2);
t3648 = t21.*(t1896-t3239).*(-1.247162e-2);
t3655 = t28.*(t1896-t3239).*1.838876e-2;
t3666 = t27.*(t1896-t3239).*(-3.131399999999998e-4);
t3676 = t27.*(t1896-t3239).*(-4.36041e-5);
t3683 = t3003.*t3133;
t3687 = t50.*t202.*t3370.*8.875020496606951e-23;
t3692 = t50.*t202.*t3370.*9.733893447891495e-23;
t3695 = t50.*t202.*t3370.*8.588729512845436e-24;
t3703 = t3055.*t3098;
t3704 = t3055.*t3099;
t3707 = t3055.*t3104;
t3708 = t3055.*t3105;
t3711 = t1065+t1084+t2845+t2916;
t3720 = t21.*(t1896-t3239).*(-1.35652563578e-4);
t3723 = t28.*(t1896-t3239).*(-1.33637554986e-4);
t3726 = t28.*(t1896-t3239).*(-7.26350557185e-5);
t3727 = t27.*(t1896-t3239).*(-6.1855407534e-5);
t3730 = t21.*(t1896-t3239).*1.35652563578e-4;
t3756 = t3055.*t3133;
t3758 = -t3133.*(t1477-t2502);
t3759 = t3099+t3104;
t3760 = t3098+t3105;
t3763 = t3133.*(t1477-t2502);
t3764 = t2981.*t3237;
t3765 = t3762.*(-1.0./2.0);
t3771 = t2363.*t3370.*9.3e-7;
t3772 = t2363.*t3370.*1.02e-6;
t3773 = t2388.*t3370.*9.3e-7;
t3774 = t2363.*t3370.*9.0e-8;
t3778 = t2388.*t3370.*9.0e-8;
t3782 = t2419.*t3370.*9.3e-7;
t3791 = t2419.*t3370.*9.0e-8;
t3799 = t3055.*t3128.*9.3e-7;
t3803 = t3055.*t3128.*9.0e-8;
t3811 = t2363.*t3483;
t3813 = t2388.*t3483;
t3815 = t1951+t2028+t2841+t2871;
t3816 = t2419.*t3483;
t3820 = -t3817;
t3824 = t3003.*t3370.*9.3e-7;
t3827 = t3003.*t3370.*9.0e-8;
t3828 = t3003.*(t2337+t12.*(t1456-t2355)).*(-1.02e-6);
t3833 = t3003.*(t2337+t12.*(t1456-t2355)).*(-9.0e-8);
t3834 = t3120.*t3237;
t3836 = -t3831;
t3839 = t3055.*t3370.*9.3e-7;
t3840 = t3055.*t3370.*1.02e-6;
t3844 = t3370.*(t1477-t2502).*(-9.3e-7);
t3846 = t3055.*t3370.*9.0e-8;
t3851 = t3370.*(t1477-t2502).*(-9.0e-8);
t3852 = -t2973.*(t1896-t3239);
t3865 = t3166.*t3237;
t3869 = -t2976.*(t1896-t3239);
t3871 = t2976.*(t1896-t3239);
t3872 = t612+t989+t1071+t1083+t2885+t2912;
t3873 = t2840+t2842+t2855+t2877;
t3874 = t2829+t2839+t2878+t2880;
t3883 = t3217.*t3237.*3.24e-6;
t3884 = t3217.*t3237.*3.11e-6;
t3885 = (t1545-t2615).*(t1896-t3239);
t3893 = t336+t1538+t1966+t2024+t2843+t2913;
t3895 = t3894.*(-1.0./2.0);
t3896 = t3894./2.0;
t3899 = -t3119.*(t1896-t3239);
t3907 = -t21.*t3133.*(t1896-t3239);
t3909 = t21.*t3133.*(t1896-t3239);
t3924 = t1000+t1002+t1006+t1040+t1493+t2772+t2776;
t3925 = t1492+t2501+t3089+t3090;
t3926 = t3920.*(3.0./5.0e+2);
t3929 = -t3155.*(t1896-t3239);
t3933 = t3155.*(t1896-t3239);
t3943 = t1003+t1035+t1044+t1063+t1515+t2876+t2881;
t3949 = t3946.*(3.0./5.0e+2);
t3951 = t1514+t2547+t3110+t3111;
t3953 = t3917.*5.84482e-3;
t3954 = t3922.*1.247162e-2;
t3957 = t3917.*6.48e-5;
t3962 = t3920.*5.68686e-3;
t3970 = t3919.*6.47e-6;
t3971 = t3920.*3.131399999999998e-4;
t3975 = t2470+t2751+t2761+t2763+t2764;
t3978 = t3942.*1.247162e-2;
t3981 = t3940.*5.84482e-3;
t3986 = t3940.*6.48e-5;
t3987 = -t3213.*(t1896-t3239);
t3996 = t3946.*3.131399999999998e-4;
t3998 = t3941.*6.47e-6;
t3999 = t3946.*4.36041e-5;
t4010 = t3236.*(t1861-t3221).*(-1.0e-8);
t4018 = t2535+t2836+t2853+t2889+t2897;
t4022 = -t3814.*(t1477-t2502);
t4027 = t3055.*t3819;
t4028 = t3814.*(t1477-t2502);
t4032 = t3940.*1.688944904408e-4;
t4034 = t3946.*6.1855407534e-5;
t4036 = t3942.*1.35652563578e-4;
t4042 = t3940.*7.0482312e-7;
t4047 = t3941.*1.869599668e-7;
t4061 = t3236.*(t1861-t3221).*(-9.840000000000001e-6);
t4071 = t3236.*(t1861-t3221).*(-6.2e-7);
t4076 = t3236.*(t1861-t3221).*(-3.24e-6);
t4078 = t3236.*(t1861-t3221).*(-7.83e-6);
t4083 = t3236.*(t1861-t3221).*3.24e-6;
t4084 = t3236.*(t1861-t3221).*7.83e-6;
t4086 = t16.*t3236.*(t1861-t3221).*(-5.7e-7);
t4087 = t11.*t3236.*(t1861-t3221).*(-1.02e-6);
t4092 = t16.*t3236.*(t1861-t3221).*5.7e-7;
t4094 = t11.*t3236.*(t1861-t3221).*(-2.4e-7);
t4096 = t11.*t3236.*(t1861-t3221).*(-4.0e-8);
t4098 = t16.*t3236.*(t1861-t3221).*(-4.0e-8);
t4101 = t11.*t3236.*(t1861-t3221).*2.4e-7;
tau_c = ft_8({dq1,dq2,dq3,dq4,dq5,dq6,t10,t1000,t1003,t1005,t1015,t1018,t1020,t1022,t1023,t1045,t1046,t1049,t1050,t1051,t1067,t1068,t1089,t1093,t11,t1104,t1105,t1108,t1115,t1121,t1158,t1159,t1190,t1193,t1194,t1196,t12,t1205,t1207,t1208,t1210,t1212,t1214,t1217,t1218,t1219,t1220,t1221,t1222,t123,t1230,t1235,t1236,t1237,t1238,t1288,t1289,t13,t1302,t1303,t1319,t1320,t1336,t1348,t1350,t1351,t1360,t1369,t1378,t1396,t14,t140,t1425,t1435,t1456,t1477,t1488,t1494,t15,t1505,t1513,t1516,t1526,t1527,t1529,t1539,t1543,t1544,t1545,t1547,t1548,t1549,t1553,t1554,t1558,t1559,t1564,t1565,t1576,t1577,t1578,t1579,t1581,t1584,t1585,t1586,t1587,t1591,t1595,t1596,t1598,t1599,t16,t1600,t1601,t1602,t1604,t1605,t1606,t1607,t1608,t1609,t1612,t1613,t1614,t1615,t1616,t1626,t1627,t1628,t1629,t1631,t1637,t1640,t1641,t1648,t1649,t1659,t1660,t1661,t1666,t1667,t1683,t1686,t1690,t1692,t17,t1700,t1701,t1703,t1704,t1705,t1712,t1717,t1738,t1741,t1742,t1750,t1752,t1753,t1754,t1758,t1759,t1775,t1776,t18,t1861,t1865,t1868,t1870,t1874,t1876,t1879,t188,t1881,t1882,t1886,t1889,t189,t1890,t1896,t19,t1900,t1901,t1905,t1911,t1913,t1918,t1923,t1927,t1930,t1931,t1933,t1941,t1945,t1948,t1953,t1954,t1957,t1959,t1963,t1964,t1971,t1973,t1992,t1993,t1994,t1998,t20,t2004,t201,t202,t2023,t2053,t2060,t2089,t2090,t2098,t2099,t21,t2117,t2120,t2122,t2123,t2125,t2130,t2137,t2138,t2139,t2140,t2141,t2142,t2145,t2146,t2147,t2149,t2150,t2151,t2152,t2153,t2154,t2155,t2156,t2157,t2159,t2160,t2162,t2164,t2165,t2166,t2167,t2168,t2169,t2174,t2183,t2187,t2193,t2194,t2195,t2199,t22,t2203,t2215,t2219,t2222,t2223,t2239,t2240,t2256,t2257,t2290,t2291,t2292,t2293,t2294,t2295,t2296,t2297,t2298,t2299,t2300,t2301,t2302,t2303,t2304,t2306,t2307,t2308,t2309,t2310,t2311,t2312,t2313,t2317,t2320,t2322,t2323,t2324,t2325,t2326,t2327,t2328,t2329,t2337,t2338,t2339,t2341,t2342,t2343,t2344,t2352,t2353,t2354,t2355,t2357,t2358,t2359,t236,t2360,t2361,t2362,t2363,t2364,t2365,t2366,t2367,t2368,t2369,t237,t2370,t2371,t2374,t2375,t2378,t2379,t238,t2380,t2384,t2385,t2386,t2388,t2389,t2391,t2393,t2394,t2395,t2396,t2397,t2398,t2399,t24,t2400,t2401,t2402,t2403,t2404,t2405,t241,t2410,t2413,t2414,t2419,t2421,t2422,t2423,t2433,t2434,t2438,t2447,t2448,t2449,t2450,t2459,t2460,t2461,t2471,t2472,t2492,t2493,t2494,t25,t2500,t2502,t2507,t2508,t2509,t2510,t2515,t2517,t2519,t2520,t2523,t2525,t2527,t2529,t2530,t2532,t2534,t2539,t2553,t2555,t2556,t2572,t2575,t2583,t2598,t26,t2605,t2606,t2612,t2613,t2615,t2618,t2619,t262,t2636,t2638,t264,t2651,t2652,t2664,t2670,t2671,t2673,t2674,t2675,t2676,t2678,t2680,t2681,t2682,t2683,t2684,t2685,t2686,t2687,t2689,t2690,t2692,t2693,t2694,t2695,t2696,t2697,t2698,t27,t2700,t2701,t2704,t2705,t2707,t2708,t2709,t2711,t2712,t2713,t2715,t2716,t2717,t2719,t2720,t2721,t2732,t2733,t2735,t2736,t2740,t2742,t2743,t2744,t2745,t2747,t2748,t2749,t2750,t2751,t2753,t2754,t2755,t2757,t2759,t2760,t2761,t2763,t2764,t2765,t2766,t2769,t2773,t2774,t2775,t2777,t2778,t2779,t2781,t2785,t2786,t2787,t2788,t2789,t2790,t2791,t2792,t2793,t2794,t2795,t2797,t2798,t2799,t28,t2801,t2802,t2803,t2804,t2805,t2807,t2808,t2809,t2813,t2814,t2815,t2817,t2818,t2819,t2820,t2822,t2823,t2828,t2831,t2832,t2834,t2835,t2836,t2837,t2838,t2844,t2850,t2851,t2852,t2853,t2862,t2864,t2889,t2897,t29,t2902,t2904,t2909,t2910,t2921,t2927,t2929,t2932,t2934,t2936,t2937,t2938,t2941,t2942,t2945,t2946,t2947,t2948,t2950,t2951,t2953,t2954,t2955,t2956,t2957,t2961,t2962,t2963,t2964,t2965,t2966,t2969,t2970,t2971,t2972,t2973,t2975,t2976,t2977,t2978,t2979,t2982,t2984,t2985,t2986,t2987,t2990,t2991,t2993,t2994,t2997,t2998,t30,t3003,t3004,t3006,t3008,t3009,t3010,t3015,t3016,t3017,t3018,t3019,t3020,t3021,t3022,t3027,t3029,t3030,t3031,t3032,t3033,t3034,t3035,t3036,t3040,t3041,t3043,t3044,t3045,t3047,t3049,t3050,t3051,t3054,t3055,t3057,t3058,t3063,t3064,t3065,t3066,t3067,t3068,t3069,t3072,t3073,t3074,t3075,t3076,t3077,t3078,t3079,t3080,t3081,t3082,t3083,t3085,t3086,t3087,t3088,t3089,t3090,t3096,t3097,t31,t3109,t3110,t3111,t3113,t3114,t3115,t3116,t3117,t3118,t3119,t3121,t3122,t3126,t3129,t313,t3130,t3131,t3132,t3133,t3134,t3135,t3136,t314,t3140,t3141,t3142,t3143,t3145,t3148,t3150,t3151,t3153,t3154,t3155,t3156,t3157,t3158,t3159,t3160,t3161,t3162,t3163,t3164,t3165,t3166,t3167,t3171,t3172,t3173,t3179,t3180,t3181,t3184,t3185,t3187,t3188,t3189,t3190,t3191,t3192,t3193,t3194,t3195,t3196,t3198,t3199,t32,t3200,t3201,t3202,t3203,t3205,t3208,t3209,t321,t3211,t3212,t3213,t3216,t3217,t3218,t3219,t322,t3221,t3222,t3224,t3225,t3226,t3227,t3228,t3229,t3230,t3231,t3235,t3236,t3237,t3238,t3239,t3240,t3242,t3243,t3244,t3245,t3246,t3247,t3248,t3250,t3251,t3256,t3257,t3259,t326,t3260,t3261,t3263,t3265,t3266,t3267,t3268,t3269,t3270,t3271,t3272,t3273,t3276,t3277,t3278,t3279,t328,t3280,t3281,t3285,t3286,t3287,t329,t3290,t33,t330,t3303,t3304,t3306,t3307,t331,t3313,t3315,t3318,t3319,t332,t3322,t3324,t3325,t3326,t3328,t3329,t333,t3330,t3331,t3336,t3337,t3340,t3343,t3344,t3345,t335,t3351,t3354,t3356,t3357,t3358,t3359,t3369,t3370,t3377,t3379,t338,t3380,t3383,t3386,t3387,t3389,t339,t3392,t3393,t3394,t3395,t3396,t3397,t3398,t3399,t34,t3400,t3401,t3402,t3403,t341,t3412,t3413,t3416,t3417,t3418,t3426,t3428,t343,t3431,t3432,t3433,t3434,t3435,t3436,t3438,t3439,t3440,t3441,t3443,t3445,t3446,t3447,t3448,t3449,t3451,t3452,t3453,t3454,t3455,t3456,t3457,t3458,t346,t3460,t3461,t3462,t3463,t3464,t3465,t3467,t3468,t3469,t3470,t3471,t3472,t3473,t3474,t3475,t3476,t3477,t3478,t3479,t3483,t3488,t3489,t3490,t3491,t3492,t3493,t3496,t3497,t3499,t35,t350,t3500,t3508,t3509,t351,t3517,t352,t3524,t3530,t3536,t3538,t3539,t354,t3540,t3541,t3543,t3545,t3546,t3552,t3559,t356,t3560,t3566,t3577,t3578,t358,t3580,t3585,t3588,t359,t3590,t3597,t3598,t3599,t36,t360,t3600,t3602,t3604,t3605,t3609,t3611,t362,t3628,t363,t3638,t364,t3644,t3646,t3648,t3649,t365,t3655,t366,t3666,t3676,t3683,t3687,t369,t3692,t3693,t3695,t3696,t3699,t370,t3700,t3701,t3702,t3703,t3704,t3705,t3706,t3707,t3708,t3709,t371,t3710,t3711,t3712,t372,t3723,t3726,t3727,t3730,t3755,t3756,t3759,t3760,t3761,t3762,t3763,t3764,t3765,t3771,t3772,t3773,t3774,t3777,t3778,t3779,t378,t3782,t3784,t3785,t3788,t3790,t3791,t3792,t3793,t3794,t3796,t3797,t3798,t3799,t38,t380,t3800,t3802,t3803,t3805,t3808,t3809,t3810,t3811,t3812,t3813,t3814,t3815,t3816,t3817,t3819,t382,t3820,t3824,t3827,t3828,t3831,t3833,t3834,t3836,t3839,t3840,t3844,t3846,t3848,t3851,t3852,t3855,t3856,t3857,t3861,t3862,t3863,t3865,t387,t3871,t3872,t3873,t3874,t3876,t3877,t3878,t3879,t3880,t3881,t3882,t3883,t3884,t3885,t3893,t3894,t3895,t3896,t3897,t3898,t3899,t39,t3901,t3902,t3903,t3909,t3910,t3913,t3915,t3917,t3919,t3920,t3922,t3924,t3925,t3926,t3927,t3931,t3933,t3934,t3937,t3940,t3941,t3942,t3943,t3946,t3947,t3948,t3949,t3950,t3951,t3953,t3954,t3955,t3957,t3961,t3962,t3963,t3964,t3965,t3968,t3969,t3970,t3971,t3972,t3974,t3975,t3978,t3981,t3986,t3987,t3989,t3990,t3994,t3996,t3998,t3999,t4000,t4004,t4005,t4008,t4010,t4018,t4027,t4028,t4032,t4034,t4035,t4036,t4038,t4040,t4042,t4043,t4047,t4050,t4057,t4061,t4071,t4083,t4084,t4086,t4087,t4092,t4096,t4098,t410,t4101,t4137,t4142,t4145,t4146,t4147,t4149,t4153,t4154,t4155,t4160,t4163,t4165,t4167,t4177,t4194,t4196,t4198,t42,t4201,t4203,t4206,t4211,t4212,t4222,t4223,t4231,t4232,t4233,t4234,t4252,t4255,t4256,t4260,t4261,t4263,t4273,t4274,t4275,t4287,t4288,t429,t43,t4313,t4314,t4324,t4325,t4326,t4328,t4334,t4343,t4347,t4348,t4365,t4366,t4372,t4373,t4375,t4377,t4378,t4384,t4387,t4389,t4390,t4392,t4398,t4401,t4402,t4410,t4413,t4415,t4421,t4424,t4437,t4468,t4476,t4501,t4502,t4559,t4563,t46,t4644,t4652,t4663,t4665,t4677,t4678,t4680,t4683,t47,t4703,t4704,t4705,t4708,t4709,t4713,t4716,t4722,t4724,t4725,t4728,t4730,t4741,t4744,t4746,t4749,t4750,t4751,t4754,t4755,t4756,t4757,t4759,t4760,t4761,t4762,t4763,t4814,t4828,t4833,t4837,t4847,t4850,t4879,t4895,t4902,t4915,t4920,t4923,t4924,t4951,t50,t5015,t5016,t5025,t5027,t5036,t5037,t5087,t5091,t5093,t5096,t5097,t5098,t523,t524,t5278,t5279,t528,t5283,t5296,t530,t5302,t5304,t5308,t5309,t5361,t5363,t5370,t5372,t5381,t5391,t5392,t5393,t5395,t5399,t5400,t5401,t5402,t5403,t5404,t542,t543,t5433,t5434,t5436,t5437,t5438,t5439,t5452,t5456,t5457,t5458,t5459,t5460,t5464,t5481,t549,t5499,t5537,t5540,t5541,t5542,t5544,t5545,t5548,t5550,t5561,t5569,t5570,t5586,t56,t5604,t5607,t562,t563,t5678,t5684,t575,t5782,t5783,t58,t587,t59,t5901,t5902,t594,t5990,t60,t6011,t6013,t6014,t610,t6255,t6256,t6257,t628,t635,t636,t638,t640,t641,t642,t643,t644,t645,t646,t649,t654,t655,t656,t657,t659,t660,t6622,t6623,t663,t664,t665,t666,t667,t668,t669,t67,t670,t672,t673,t674,t6745,t675,t6751,t676,t677,t678,t679,t68,t681,t682,t683,t684,t685,t686,t687,t689,t691,t6919,t692,t6920,t693,t694,t6987,t70,t702,t707,t708,t71,t710,t715,t716,t717,t718,t721,t722,t724,t725,t73,t736,t738,t740,t741,t749,t756,t76,t762,t768,t777,t792,t793,t8,t801,t802,t808,t813,t819,t821,t850,t855,t874,t878,t89,t9,t90,t91,t92,t941,t944,t945,t948,t949,t951,t97,t983,t996});
end
function tau_c = ft_8(ct)
dq1 = ct{1};
dq2 = ct{2};
dq3 = ct{3};
dq4 = ct{4};
dq5 = ct{5};
dq6 = ct{6};
t10 = ct{7};
t1000 = ct{8};
t1003 = ct{9};
t1005 = ct{10};
t1015 = ct{11};
t1018 = ct{12};
t1020 = ct{13};
t1022 = ct{14};
t1023 = ct{15};
t1045 = ct{16};
t1046 = ct{17};
t1049 = ct{18};
t1050 = ct{19};
t1051 = ct{20};
t1067 = ct{21};
t1068 = ct{22};
t1089 = ct{23};
t1093 = ct{24};
t11 = ct{25};
t1104 = ct{26};
t1105 = ct{27};
t1108 = ct{28};
t1115 = ct{29};
t1121 = ct{30};
t1158 = ct{31};
t1159 = ct{32};
t1190 = ct{33};
t1193 = ct{34};
t1194 = ct{35};
t1196 = ct{36};
t12 = ct{37};
t1205 = ct{38};
t1207 = ct{39};
t1208 = ct{40};
t1210 = ct{41};
t1212 = ct{42};
t1214 = ct{43};
t1217 = ct{44};
t1218 = ct{45};
t1219 = ct{46};
t1220 = ct{47};
t1221 = ct{48};
t1222 = ct{49};
t123 = ct{50};
t1230 = ct{51};
t1235 = ct{52};
t1236 = ct{53};
t1237 = ct{54};
t1238 = ct{55};
t1288 = ct{56};
t1289 = ct{57};
t13 = ct{58};
t1302 = ct{59};
t1303 = ct{60};
t1319 = ct{61};
t1320 = ct{62};
t1336 = ct{63};
t1348 = ct{64};
t1350 = ct{65};
t1351 = ct{66};
t1360 = ct{67};
t1369 = ct{68};
t1378 = ct{69};
t1396 = ct{70};
t14 = ct{71};
t140 = ct{72};
t1425 = ct{73};
t1435 = ct{74};
t1456 = ct{75};
t1477 = ct{76};
t1488 = ct{77};
t1494 = ct{78};
t15 = ct{79};
t1505 = ct{80};
t1513 = ct{81};
t1516 = ct{82};
t1526 = ct{83};
t1527 = ct{84};
t1529 = ct{85};
t1539 = ct{86};
t1543 = ct{87};
t1544 = ct{88};
t1545 = ct{89};
t1547 = ct{90};
t1548 = ct{91};
t1549 = ct{92};
t1553 = ct{93};
t1554 = ct{94};
t1558 = ct{95};
t1559 = ct{96};
t1564 = ct{97};
t1565 = ct{98};
t1576 = ct{99};
t1577 = ct{100};
t1578 = ct{101};
t1579 = ct{102};
t1581 = ct{103};
t1584 = ct{104};
t1585 = ct{105};
t1586 = ct{106};
t1587 = ct{107};
t1591 = ct{108};
t1595 = ct{109};
t1596 = ct{110};
t1598 = ct{111};
t1599 = ct{112};
t16 = ct{113};
t1600 = ct{114};
t1601 = ct{115};
t1602 = ct{116};
t1604 = ct{117};
t1605 = ct{118};
t1606 = ct{119};
t1607 = ct{120};
t1608 = ct{121};
t1609 = ct{122};
t1612 = ct{123};
t1613 = ct{124};
t1614 = ct{125};
t1615 = ct{126};
t1616 = ct{127};
t1626 = ct{128};
t1627 = ct{129};
t1628 = ct{130};
t1629 = ct{131};
t1631 = ct{132};
t1637 = ct{133};
t1640 = ct{134};
t1641 = ct{135};
t1648 = ct{136};
t1649 = ct{137};
t1659 = ct{138};
t1660 = ct{139};
t1661 = ct{140};
t1666 = ct{141};
t1667 = ct{142};
t1683 = ct{143};
t1686 = ct{144};
t1690 = ct{145};
t1692 = ct{146};
t17 = ct{147};
t1700 = ct{148};
t1701 = ct{149};
t1703 = ct{150};
t1704 = ct{151};
t1705 = ct{152};
t1712 = ct{153};
t1717 = ct{154};
t1738 = ct{155};
t1741 = ct{156};
t1742 = ct{157};
t1750 = ct{158};
t1752 = ct{159};
t1753 = ct{160};
t1754 = ct{161};
t1758 = ct{162};
t1759 = ct{163};
t1775 = ct{164};
t1776 = ct{165};
t18 = ct{166};
t1861 = ct{167};
t1865 = ct{168};
t1868 = ct{169};
t1870 = ct{170};
t1874 = ct{171};
t1876 = ct{172};
t1879 = ct{173};
t188 = ct{174};
t1881 = ct{175};
t1882 = ct{176};
t1886 = ct{177};
t1889 = ct{178};
t189 = ct{179};
t1890 = ct{180};
t1896 = ct{181};
t19 = ct{182};
t1900 = ct{183};
t1901 = ct{184};
t1905 = ct{185};
t1911 = ct{186};
t1913 = ct{187};
t1918 = ct{188};
t1923 = ct{189};
t1927 = ct{190};
t1930 = ct{191};
t1931 = ct{192};
t1933 = ct{193};
t1941 = ct{194};
t1945 = ct{195};
t1948 = ct{196};
t1953 = ct{197};
t1954 = ct{198};
t1957 = ct{199};
t1959 = ct{200};
t1963 = ct{201};
t1964 = ct{202};
t1971 = ct{203};
t1973 = ct{204};
t1992 = ct{205};
t1993 = ct{206};
t1994 = ct{207};
t1998 = ct{208};
t20 = ct{209};
t2004 = ct{210};
t201 = ct{211};
t202 = ct{212};
t2023 = ct{213};
t2053 = ct{214};
t2060 = ct{215};
t2089 = ct{216};
t2090 = ct{217};
t2098 = ct{218};
t2099 = ct{219};
t21 = ct{220};
t2117 = ct{221};
t2120 = ct{222};
t2122 = ct{223};
t2123 = ct{224};
t2125 = ct{225};
t2130 = ct{226};
t2137 = ct{227};
t2138 = ct{228};
t2139 = ct{229};
t2140 = ct{230};
t2141 = ct{231};
t2142 = ct{232};
t2145 = ct{233};
t2146 = ct{234};
t2147 = ct{235};
t2149 = ct{236};
t2150 = ct{237};
t2151 = ct{238};
t2152 = ct{239};
t2153 = ct{240};
t2154 = ct{241};
t2155 = ct{242};
t2156 = ct{243};
t2157 = ct{244};
t2159 = ct{245};
t2160 = ct{246};
t2162 = ct{247};
t2164 = ct{248};
t2165 = ct{249};
t2166 = ct{250};
t2167 = ct{251};
t2168 = ct{252};
t2169 = ct{253};
t2174 = ct{254};
t2183 = ct{255};
t2187 = ct{256};
t2193 = ct{257};
t2194 = ct{258};
t2195 = ct{259};
t2199 = ct{260};
t22 = ct{261};
t2203 = ct{262};
t2215 = ct{263};
t2219 = ct{264};
t2222 = ct{265};
t2223 = ct{266};
t2239 = ct{267};
t2240 = ct{268};
t2256 = ct{269};
t2257 = ct{270};
t2290 = ct{271};
t2291 = ct{272};
t2292 = ct{273};
t2293 = ct{274};
t2294 = ct{275};
t2295 = ct{276};
t2296 = ct{277};
t2297 = ct{278};
t2298 = ct{279};
t2299 = ct{280};
t2300 = ct{281};
t2301 = ct{282};
t2302 = ct{283};
t2303 = ct{284};
t2304 = ct{285};
t2306 = ct{286};
t2307 = ct{287};
t2308 = ct{288};
t2309 = ct{289};
t2310 = ct{290};
t2311 = ct{291};
t2312 = ct{292};
t2313 = ct{293};
t2317 = ct{294};
t2320 = ct{295};
t2322 = ct{296};
t2323 = ct{297};
t2324 = ct{298};
t2325 = ct{299};
t2326 = ct{300};
t2327 = ct{301};
t2328 = ct{302};
t2329 = ct{303};
t2337 = ct{304};
t2338 = ct{305};
t2339 = ct{306};
t2341 = ct{307};
t2342 = ct{308};
t2343 = ct{309};
t2344 = ct{310};
t2352 = ct{311};
t2353 = ct{312};
t2354 = ct{313};
t2355 = ct{314};
t2357 = ct{315};
t2358 = ct{316};
t2359 = ct{317};
t236 = ct{318};
t2360 = ct{319};
t2361 = ct{320};
t2362 = ct{321};
t2363 = ct{322};
t2364 = ct{323};
t2365 = ct{324};
t2366 = ct{325};
t2367 = ct{326};
t2368 = ct{327};
t2369 = ct{328};
t237 = ct{329};
t2370 = ct{330};
t2371 = ct{331};
t2374 = ct{332};
t2375 = ct{333};
t2378 = ct{334};
t2379 = ct{335};
t238 = ct{336};
t2380 = ct{337};
t2384 = ct{338};
t2385 = ct{339};
t2386 = ct{340};
t2388 = ct{341};
t2389 = ct{342};
t2391 = ct{343};
t2393 = ct{344};
t2394 = ct{345};
t2395 = ct{346};
t2396 = ct{347};
t2397 = ct{348};
t2398 = ct{349};
t2399 = ct{350};
t24 = ct{351};
t2400 = ct{352};
t2401 = ct{353};
t2402 = ct{354};
t2403 = ct{355};
t2404 = ct{356};
t2405 = ct{357};
t241 = ct{358};
t2410 = ct{359};
t2413 = ct{360};
t2414 = ct{361};
t2419 = ct{362};
t2421 = ct{363};
t2422 = ct{364};
t2423 = ct{365};
t2433 = ct{366};
t2434 = ct{367};
t2438 = ct{368};
t2447 = ct{369};
t2448 = ct{370};
t2449 = ct{371};
t2450 = ct{372};
t2459 = ct{373};
t2460 = ct{374};
t2461 = ct{375};
t2471 = ct{376};
t2472 = ct{377};
t2492 = ct{378};
t2493 = ct{379};
t2494 = ct{380};
t25 = ct{381};
t2500 = ct{382};
t2502 = ct{383};
t2507 = ct{384};
t2508 = ct{385};
t2509 = ct{386};
t2510 = ct{387};
t2515 = ct{388};
t2517 = ct{389};
t2519 = ct{390};
t2520 = ct{391};
t2523 = ct{392};
t2525 = ct{393};
t2527 = ct{394};
t2529 = ct{395};
t2530 = ct{396};
t2532 = ct{397};
t2534 = ct{398};
t2539 = ct{399};
t2553 = ct{400};
t2555 = ct{401};
t2556 = ct{402};
t2572 = ct{403};
t2575 = ct{404};
t2583 = ct{405};
t2598 = ct{406};
t26 = ct{407};
t2605 = ct{408};
t2606 = ct{409};
t2612 = ct{410};
t2613 = ct{411};
t2615 = ct{412};
t2618 = ct{413};
t2619 = ct{414};
t262 = ct{415};
t2636 = ct{416};
t2638 = ct{417};
t264 = ct{418};
t2651 = ct{419};
t2652 = ct{420};
t2664 = ct{421};
t2670 = ct{422};
t2671 = ct{423};
t2673 = ct{424};
t2674 = ct{425};
t2675 = ct{426};
t2676 = ct{427};
t2678 = ct{428};
t2680 = ct{429};
t2681 = ct{430};
t2682 = ct{431};
t2683 = ct{432};
t2684 = ct{433};
t2685 = ct{434};
t2686 = ct{435};
t2687 = ct{436};
t2689 = ct{437};
t2690 = ct{438};
t2692 = ct{439};
t2693 = ct{440};
t2694 = ct{441};
t2695 = ct{442};
t2696 = ct{443};
t2697 = ct{444};
t2698 = ct{445};
t27 = ct{446};
t2700 = ct{447};
t2701 = ct{448};
t2704 = ct{449};
t2705 = ct{450};
t2707 = ct{451};
t2708 = ct{452};
t2709 = ct{453};
t2711 = ct{454};
t2712 = ct{455};
t2713 = ct{456};
t2715 = ct{457};
t2716 = ct{458};
t2717 = ct{459};
t2719 = ct{460};
t2720 = ct{461};
t2721 = ct{462};
t2732 = ct{463};
t2733 = ct{464};
t2735 = ct{465};
t2736 = ct{466};
t2740 = ct{467};
t2742 = ct{468};
t2743 = ct{469};
t2744 = ct{470};
t2745 = ct{471};
t2747 = ct{472};
t2748 = ct{473};
t2749 = ct{474};
t2750 = ct{475};
t2751 = ct{476};
t2753 = ct{477};
t2754 = ct{478};
t2755 = ct{479};
t2757 = ct{480};
t2759 = ct{481};
t2760 = ct{482};
t2761 = ct{483};
t2763 = ct{484};
t2764 = ct{485};
t2765 = ct{486};
t2766 = ct{487};
t2769 = ct{488};
t2773 = ct{489};
t2774 = ct{490};
t2775 = ct{491};
t2777 = ct{492};
t2778 = ct{493};
t2779 = ct{494};
t2781 = ct{495};
t2785 = ct{496};
t2786 = ct{497};
t2787 = ct{498};
t2788 = ct{499};
t2789 = ct{500};
t2790 = ct{501};
t2791 = ct{502};
t2792 = ct{503};
t2793 = ct{504};
t2794 = ct{505};
t2795 = ct{506};
t2797 = ct{507};
t2798 = ct{508};
t2799 = ct{509};
t28 = ct{510};
t2801 = ct{511};
t2802 = ct{512};
t2803 = ct{513};
t2804 = ct{514};
t2805 = ct{515};
t2807 = ct{516};
t2808 = ct{517};
t2809 = ct{518};
t2813 = ct{519};
t2814 = ct{520};
t2815 = ct{521};
t2817 = ct{522};
t2818 = ct{523};
t2819 = ct{524};
t2820 = ct{525};
t2822 = ct{526};
t2823 = ct{527};
t2828 = ct{528};
t2831 = ct{529};
t2832 = ct{530};
t2834 = ct{531};
t2835 = ct{532};
t2836 = ct{533};
t2837 = ct{534};
t2838 = ct{535};
t2844 = ct{536};
t2850 = ct{537};
t2851 = ct{538};
t2852 = ct{539};
t2853 = ct{540};
t2862 = ct{541};
t2864 = ct{542};
t2889 = ct{543};
t2897 = ct{544};
t29 = ct{545};
t2902 = ct{546};
t2904 = ct{547};
t2909 = ct{548};
t2910 = ct{549};
t2921 = ct{550};
t2927 = ct{551};
t2929 = ct{552};
t2932 = ct{553};
t2934 = ct{554};
t2936 = ct{555};
t2937 = ct{556};
t2938 = ct{557};
t2941 = ct{558};
t2942 = ct{559};
t2945 = ct{560};
t2946 = ct{561};
t2947 = ct{562};
t2948 = ct{563};
t2950 = ct{564};
t2951 = ct{565};
t2953 = ct{566};
t2954 = ct{567};
t2955 = ct{568};
t2956 = ct{569};
t2957 = ct{570};
t2961 = ct{571};
t2962 = ct{572};
t2963 = ct{573};
t2964 = ct{574};
t2965 = ct{575};
t2966 = ct{576};
t2969 = ct{577};
t2970 = ct{578};
t2971 = ct{579};
t2972 = ct{580};
t2973 = ct{581};
t2975 = ct{582};
t2976 = ct{583};
t2977 = ct{584};
t2978 = ct{585};
t2979 = ct{586};
t2982 = ct{587};
t2984 = ct{588};
t2985 = ct{589};
t2986 = ct{590};
t2987 = ct{591};
t2990 = ct{592};
t2991 = ct{593};
t2993 = ct{594};
t2994 = ct{595};
t2997 = ct{596};
t2998 = ct{597};
t30 = ct{598};
t3003 = ct{599};
t3004 = ct{600};
t3006 = ct{601};
t3008 = ct{602};
t3009 = ct{603};
t3010 = ct{604};
t3015 = ct{605};
t3016 = ct{606};
t3017 = ct{607};
t3018 = ct{608};
t3019 = ct{609};
t3020 = ct{610};
t3021 = ct{611};
t3022 = ct{612};
t3027 = ct{613};
t3029 = ct{614};
t3030 = ct{615};
t3031 = ct{616};
t3032 = ct{617};
t3033 = ct{618};
t3034 = ct{619};
t3035 = ct{620};
t3036 = ct{621};
t3040 = ct{622};
t3041 = ct{623};
t3043 = ct{624};
t3044 = ct{625};
t3045 = ct{626};
t3047 = ct{627};
t3049 = ct{628};
t3050 = ct{629};
t3051 = ct{630};
t3054 = ct{631};
t3055 = ct{632};
t3057 = ct{633};
t3058 = ct{634};
t3063 = ct{635};
t3064 = ct{636};
t3065 = ct{637};
t3066 = ct{638};
t3067 = ct{639};
t3068 = ct{640};
t3069 = ct{641};
t3072 = ct{642};
t3073 = ct{643};
t3074 = ct{644};
t3075 = ct{645};
t3076 = ct{646};
t3077 = ct{647};
t3078 = ct{648};
t3079 = ct{649};
t3080 = ct{650};
t3081 = ct{651};
t3082 = ct{652};
t3083 = ct{653};
t3085 = ct{654};
t3086 = ct{655};
t3087 = ct{656};
t3088 = ct{657};
t3089 = ct{658};
t3090 = ct{659};
t3096 = ct{660};
t3097 = ct{661};
t31 = ct{662};
t3109 = ct{663};
t3110 = ct{664};
t3111 = ct{665};
t3113 = ct{666};
t3114 = ct{667};
t3115 = ct{668};
t3116 = ct{669};
t3117 = ct{670};
t3118 = ct{671};
t3119 = ct{672};
t3121 = ct{673};
t3122 = ct{674};
t3126 = ct{675};
t3129 = ct{676};
t313 = ct{677};
t3130 = ct{678};
t3131 = ct{679};
t3132 = ct{680};
t3133 = ct{681};
t3134 = ct{682};
t3135 = ct{683};
t3136 = ct{684};
t314 = ct{685};
t3140 = ct{686};
t3141 = ct{687};
t3142 = ct{688};
t3143 = ct{689};
t3145 = ct{690};
t3148 = ct{691};
t3150 = ct{692};
t3151 = ct{693};
t3153 = ct{694};
t3154 = ct{695};
t3155 = ct{696};
t3156 = ct{697};
t3157 = ct{698};
t3158 = ct{699};
t3159 = ct{700};
t3160 = ct{701};
t3161 = ct{702};
t3162 = ct{703};
t3163 = ct{704};
t3164 = ct{705};
t3165 = ct{706};
t3166 = ct{707};
t3167 = ct{708};
t3171 = ct{709};
t3172 = ct{710};
t3173 = ct{711};
t3179 = ct{712};
t3180 = ct{713};
t3181 = ct{714};
t3184 = ct{715};
t3185 = ct{716};
t3187 = ct{717};
t3188 = ct{718};
t3189 = ct{719};
t3190 = ct{720};
t3191 = ct{721};
t3192 = ct{722};
t3193 = ct{723};
t3194 = ct{724};
t3195 = ct{725};
t3196 = ct{726};
t3198 = ct{727};
t3199 = ct{728};
t32 = ct{729};
t3200 = ct{730};
t3201 = ct{731};
t3202 = ct{732};
t3203 = ct{733};
t3205 = ct{734};
t3208 = ct{735};
t3209 = ct{736};
t321 = ct{737};
t3211 = ct{738};
t3212 = ct{739};
t3213 = ct{740};
t3216 = ct{741};
t3217 = ct{742};
t3218 = ct{743};
t3219 = ct{744};
t322 = ct{745};
t3221 = ct{746};
t3222 = ct{747};
t3224 = ct{748};
t3225 = ct{749};
t3226 = ct{750};
t3227 = ct{751};
t3228 = ct{752};
t3229 = ct{753};
t3230 = ct{754};
t3231 = ct{755};
t3235 = ct{756};
t3236 = ct{757};
t3237 = ct{758};
t3238 = ct{759};
t3239 = ct{760};
t3240 = ct{761};
t3242 = ct{762};
t3243 = ct{763};
t3244 = ct{764};
t3245 = ct{765};
t3246 = ct{766};
t3247 = ct{767};
t3248 = ct{768};
t3250 = ct{769};
t3251 = ct{770};
t3256 = ct{771};
t3257 = ct{772};
t3259 = ct{773};
t326 = ct{774};
t3260 = ct{775};
t3261 = ct{776};
t3263 = ct{777};
t3265 = ct{778};
t3266 = ct{779};
t3267 = ct{780};
t3268 = ct{781};
t3269 = ct{782};
t3270 = ct{783};
t3271 = ct{784};
t3272 = ct{785};
t3273 = ct{786};
t3276 = ct{787};
t3277 = ct{788};
t3278 = ct{789};
t3279 = ct{790};
t328 = ct{791};
t3280 = ct{792};
t3281 = ct{793};
t3285 = ct{794};
t3286 = ct{795};
t3287 = ct{796};
t329 = ct{797};
t3290 = ct{798};
t33 = ct{799};
t330 = ct{800};
t3303 = ct{801};
t3304 = ct{802};
t3306 = ct{803};
t3307 = ct{804};
t331 = ct{805};
t3313 = ct{806};
t3315 = ct{807};
t3318 = ct{808};
t3319 = ct{809};
t332 = ct{810};
t3322 = ct{811};
t3324 = ct{812};
t3325 = ct{813};
t3326 = ct{814};
t3328 = ct{815};
t3329 = ct{816};
t333 = ct{817};
t3330 = ct{818};
t3331 = ct{819};
t3336 = ct{820};
t3337 = ct{821};
t3340 = ct{822};
t3343 = ct{823};
t3344 = ct{824};
t3345 = ct{825};
t335 = ct{826};
t3351 = ct{827};
t3354 = ct{828};
t3356 = ct{829};
t3357 = ct{830};
t3358 = ct{831};
t3359 = ct{832};
t3369 = ct{833};
t3370 = ct{834};
t3377 = ct{835};
t3379 = ct{836};
t338 = ct{837};
t3380 = ct{838};
t3383 = ct{839};
t3386 = ct{840};
t3387 = ct{841};
t3389 = ct{842};
t339 = ct{843};
t3392 = ct{844};
t3393 = ct{845};
t3394 = ct{846};
t3395 = ct{847};
t3396 = ct{848};
t3397 = ct{849};
t3398 = ct{850};
t3399 = ct{851};
t34 = ct{852};
t3400 = ct{853};
t3401 = ct{854};
t3402 = ct{855};
t3403 = ct{856};
t341 = ct{857};
t3412 = ct{858};
t3413 = ct{859};
t3416 = ct{860};
t3417 = ct{861};
t3418 = ct{862};
t3426 = ct{863};
t3428 = ct{864};
t343 = ct{865};
t3431 = ct{866};
t3432 = ct{867};
t3433 = ct{868};
t3434 = ct{869};
t3435 = ct{870};
t3436 = ct{871};
t3438 = ct{872};
t3439 = ct{873};
t3440 = ct{874};
t3441 = ct{875};
t3443 = ct{876};
t3445 = ct{877};
t3446 = ct{878};
t3447 = ct{879};
t3448 = ct{880};
t3449 = ct{881};
t3451 = ct{882};
t3452 = ct{883};
t3453 = ct{884};
t3454 = ct{885};
t3455 = ct{886};
t3456 = ct{887};
t3457 = ct{888};
t3458 = ct{889};
t346 = ct{890};
t3460 = ct{891};
t3461 = ct{892};
t3462 = ct{893};
t3463 = ct{894};
t3464 = ct{895};
t3465 = ct{896};
t3467 = ct{897};
t3468 = ct{898};
t3469 = ct{899};
t3470 = ct{900};
t3471 = ct{901};
t3472 = ct{902};
t3473 = ct{903};
t3474 = ct{904};
t3475 = ct{905};
t3476 = ct{906};
t3477 = ct{907};
t3478 = ct{908};
t3479 = ct{909};
t3483 = ct{910};
t3488 = ct{911};
t3489 = ct{912};
t3490 = ct{913};
t3491 = ct{914};
t3492 = ct{915};
t3493 = ct{916};
t3496 = ct{917};
t3497 = ct{918};
t3499 = ct{919};
t35 = ct{920};
t350 = ct{921};
t3500 = ct{922};
t3508 = ct{923};
t3509 = ct{924};
t351 = ct{925};
t3517 = ct{926};
t352 = ct{927};
t3524 = ct{928};
t3530 = ct{929};
t3536 = ct{930};
t3538 = ct{931};
t3539 = ct{932};
t354 = ct{933};
t3540 = ct{934};
t3541 = ct{935};
t3543 = ct{936};
t3545 = ct{937};
t3546 = ct{938};
t3552 = ct{939};
t3559 = ct{940};
t356 = ct{941};
t3560 = ct{942};
t3566 = ct{943};
t3577 = ct{944};
t3578 = ct{945};
t358 = ct{946};
t3580 = ct{947};
t3585 = ct{948};
t3588 = ct{949};
t359 = ct{950};
t3590 = ct{951};
t3597 = ct{952};
t3598 = ct{953};
t3599 = ct{954};
t36 = ct{955};
t360 = ct{956};
t3600 = ct{957};
t3602 = ct{958};
t3604 = ct{959};
t3605 = ct{960};
t3609 = ct{961};
t3611 = ct{962};
t362 = ct{963};
t3628 = ct{964};
t363 = ct{965};
t3638 = ct{966};
t364 = ct{967};
t3644 = ct{968};
t3646 = ct{969};
t3648 = ct{970};
t3649 = ct{971};
t365 = ct{972};
t3655 = ct{973};
t366 = ct{974};
t3666 = ct{975};
t3676 = ct{976};
t3683 = ct{977};
t3687 = ct{978};
t369 = ct{979};
t3692 = ct{980};
t3693 = ct{981};
t3695 = ct{982};
t3696 = ct{983};
t3699 = ct{984};
t370 = ct{985};
t3700 = ct{986};
t3701 = ct{987};
t3702 = ct{988};
t3703 = ct{989};
t3704 = ct{990};
t3705 = ct{991};
t3706 = ct{992};
t3707 = ct{993};
t3708 = ct{994};
t3709 = ct{995};
t371 = ct{996};
t3710 = ct{997};
t3711 = ct{998};
t3712 = ct{999};
t372 = ct{1000};
t3723 = ct{1001};
t3726 = ct{1002};
t3727 = ct{1003};
t3730 = ct{1004};
t3755 = ct{1005};
t3756 = ct{1006};
t3759 = ct{1007};
t3760 = ct{1008};
t3761 = ct{1009};
t3762 = ct{1010};
t3763 = ct{1011};
t3764 = ct{1012};
t3765 = ct{1013};
t3771 = ct{1014};
t3772 = ct{1015};
t3773 = ct{1016};
t3774 = ct{1017};
t3777 = ct{1018};
t3778 = ct{1019};
t3779 = ct{1020};
t378 = ct{1021};
t3782 = ct{1022};
t3784 = ct{1023};
t3785 = ct{1024};
t3788 = ct{1025};
t3790 = ct{1026};
t3791 = ct{1027};
t3792 = ct{1028};
t3793 = ct{1029};
t3794 = ct{1030};
t3796 = ct{1031};
t3797 = ct{1032};
t3798 = ct{1033};
t3799 = ct{1034};
t38 = ct{1035};
t380 = ct{1036};
t3800 = ct{1037};
t3802 = ct{1038};
t3803 = ct{1039};
t3805 = ct{1040};
t3808 = ct{1041};
t3809 = ct{1042};
t3810 = ct{1043};
t3811 = ct{1044};
t3812 = ct{1045};
t3813 = ct{1046};
t3814 = ct{1047};
t3815 = ct{1048};
t3816 = ct{1049};
t3817 = ct{1050};
t3819 = ct{1051};
t382 = ct{1052};
t3820 = ct{1053};
t3824 = ct{1054};
t3827 = ct{1055};
t3828 = ct{1056};
t3831 = ct{1057};
t3833 = ct{1058};
t3834 = ct{1059};
t3836 = ct{1060};
t3839 = ct{1061};
t3840 = ct{1062};
t3844 = ct{1063};
t3846 = ct{1064};
t3848 = ct{1065};
t3851 = ct{1066};
t3852 = ct{1067};
t3855 = ct{1068};
t3856 = ct{1069};
t3857 = ct{1070};
t3861 = ct{1071};
t3862 = ct{1072};
t3863 = ct{1073};
t3865 = ct{1074};
t387 = ct{1075};
t3871 = ct{1076};
t3872 = ct{1077};
t3873 = ct{1078};
t3874 = ct{1079};
t3876 = ct{1080};
t3877 = ct{1081};
t3878 = ct{1082};
t3879 = ct{1083};
t3880 = ct{1084};
t3881 = ct{1085};
t3882 = ct{1086};
t3883 = ct{1087};
t3884 = ct{1088};
t3885 = ct{1089};
t3893 = ct{1090};
t3894 = ct{1091};
t3895 = ct{1092};
t3896 = ct{1093};
t3897 = ct{1094};
t3898 = ct{1095};
t3899 = ct{1096};
t39 = ct{1097};
t3901 = ct{1098};
t3902 = ct{1099};
t3903 = ct{1100};
t3909 = ct{1101};
t3910 = ct{1102};
t3913 = ct{1103};
t3915 = ct{1104};
t3917 = ct{1105};
t3919 = ct{1106};
t3920 = ct{1107};
t3922 = ct{1108};
t3924 = ct{1109};
t3925 = ct{1110};
t3926 = ct{1111};
t3927 = ct{1112};
t3931 = ct{1113};
t3933 = ct{1114};
t3934 = ct{1115};
t3937 = ct{1116};
t3940 = ct{1117};
t3941 = ct{1118};
t3942 = ct{1119};
t3943 = ct{1120};
t3946 = ct{1121};
t3947 = ct{1122};
t3948 = ct{1123};
t3949 = ct{1124};
t3950 = ct{1125};
t3951 = ct{1126};
t3953 = ct{1127};
t3954 = ct{1128};
t3955 = ct{1129};
t3957 = ct{1130};
t3961 = ct{1131};
t3962 = ct{1132};
t3963 = ct{1133};
t3964 = ct{1134};
t3965 = ct{1135};
t3968 = ct{1136};
t3969 = ct{1137};
t3970 = ct{1138};
t3971 = ct{1139};
t3972 = ct{1140};
t3974 = ct{1141};
t3975 = ct{1142};
t3978 = ct{1143};
t3981 = ct{1144};
t3986 = ct{1145};
t3987 = ct{1146};
t3989 = ct{1147};
t3990 = ct{1148};
t3994 = ct{1149};
t3996 = ct{1150};
t3998 = ct{1151};
t3999 = ct{1152};
t4000 = ct{1153};
t4004 = ct{1154};
t4005 = ct{1155};
t4008 = ct{1156};
t4010 = ct{1157};
t4018 = ct{1158};
t4027 = ct{1159};
t4028 = ct{1160};
t4032 = ct{1161};
t4034 = ct{1162};
t4035 = ct{1163};
t4036 = ct{1164};
t4038 = ct{1165};
t4040 = ct{1166};
t4042 = ct{1167};
t4043 = ct{1168};
t4047 = ct{1169};
t4050 = ct{1170};
t4057 = ct{1171};
t4061 = ct{1172};
t4071 = ct{1173};
t4083 = ct{1174};
t4084 = ct{1175};
t4086 = ct{1176};
t4087 = ct{1177};
t4092 = ct{1178};
t4096 = ct{1179};
t4098 = ct{1180};
t410 = ct{1181};
t4101 = ct{1182};
t4137 = ct{1183};
t4142 = ct{1184};
t4145 = ct{1185};
t4146 = ct{1186};
t4147 = ct{1187};
t4149 = ct{1188};
t4153 = ct{1189};
t4154 = ct{1190};
t4155 = ct{1191};
t4160 = ct{1192};
t4163 = ct{1193};
t4165 = ct{1194};
t4167 = ct{1195};
t4177 = ct{1196};
t4194 = ct{1197};
t4196 = ct{1198};
t4198 = ct{1199};
t42 = ct{1200};
t4201 = ct{1201};
t4203 = ct{1202};
t4206 = ct{1203};
t4211 = ct{1204};
t4212 = ct{1205};
t4222 = ct{1206};
t4223 = ct{1207};
t4231 = ct{1208};
t4232 = ct{1209};
t4233 = ct{1210};
t4234 = ct{1211};
t4252 = ct{1212};
t4255 = ct{1213};
t4256 = ct{1214};
t4260 = ct{1215};
t4261 = ct{1216};
t4263 = ct{1217};
t4273 = ct{1218};
t4274 = ct{1219};
t4275 = ct{1220};
t4287 = ct{1221};
t4288 = ct{1222};
t429 = ct{1223};
t43 = ct{1224};
t4313 = ct{1225};
t4314 = ct{1226};
t4324 = ct{1227};
t4325 = ct{1228};
t4326 = ct{1229};
t4328 = ct{1230};
t4334 = ct{1231};
t4343 = ct{1232};
t4347 = ct{1233};
t4348 = ct{1234};
t4365 = ct{1235};
t4366 = ct{1236};
t4372 = ct{1237};
t4373 = ct{1238};
t4375 = ct{1239};
t4377 = ct{1240};
t4378 = ct{1241};
t4384 = ct{1242};
t4387 = ct{1243};
t4389 = ct{1244};
t4390 = ct{1245};
t4392 = ct{1246};
t4398 = ct{1247};
t4401 = ct{1248};
t4402 = ct{1249};
t4410 = ct{1250};
t4413 = ct{1251};
t4415 = ct{1252};
t4421 = ct{1253};
t4424 = ct{1254};
t4437 = ct{1255};
t4468 = ct{1256};
t4476 = ct{1257};
t4501 = ct{1258};
t4502 = ct{1259};
t4559 = ct{1260};
t4563 = ct{1261};
t46 = ct{1262};
t4644 = ct{1263};
t4652 = ct{1264};
t4663 = ct{1265};
t4665 = ct{1266};
t4677 = ct{1267};
t4678 = ct{1268};
t4680 = ct{1269};
t4683 = ct{1270};
t47 = ct{1271};
t4703 = ct{1272};
t4704 = ct{1273};
t4705 = ct{1274};
t4708 = ct{1275};
t4709 = ct{1276};
t4713 = ct{1277};
t4716 = ct{1278};
t4722 = ct{1279};
t4724 = ct{1280};
t4725 = ct{1281};
t4728 = ct{1282};
t4730 = ct{1283};
t4741 = ct{1284};
t4744 = ct{1285};
t4746 = ct{1286};
t4749 = ct{1287};
t4750 = ct{1288};
t4751 = ct{1289};
t4754 = ct{1290};
t4755 = ct{1291};
t4756 = ct{1292};
t4757 = ct{1293};
t4759 = ct{1294};
t4760 = ct{1295};
t4761 = ct{1296};
t4762 = ct{1297};
t4763 = ct{1298};
t4814 = ct{1299};
t4828 = ct{1300};
t4833 = ct{1301};
t4837 = ct{1302};
t4847 = ct{1303};
t4850 = ct{1304};
t4879 = ct{1305};
t4895 = ct{1306};
t4902 = ct{1307};
t4915 = ct{1308};
t4920 = ct{1309};
t4923 = ct{1310};
t4924 = ct{1311};
t4951 = ct{1312};
t50 = ct{1313};
t5015 = ct{1314};
t5016 = ct{1315};
t5025 = ct{1316};
t5027 = ct{1317};
t5036 = ct{1318};
t5037 = ct{1319};
t5087 = ct{1320};
t5091 = ct{1321};
t5093 = ct{1322};
t5096 = ct{1323};
t5097 = ct{1324};
t5098 = ct{1325};
t523 = ct{1326};
t524 = ct{1327};
t5278 = ct{1328};
t5279 = ct{1329};
t528 = ct{1330};
t5283 = ct{1331};
t5296 = ct{1332};
t530 = ct{1333};
t5302 = ct{1334};
t5304 = ct{1335};
t5308 = ct{1336};
t5309 = ct{1337};
t5361 = ct{1338};
t5363 = ct{1339};
t5370 = ct{1340};
t5372 = ct{1341};
t5381 = ct{1342};
t5391 = ct{1343};
t5392 = ct{1344};
t5393 = ct{1345};
t5395 = ct{1346};
t5399 = ct{1347};
t5400 = ct{1348};
t5401 = ct{1349};
t5402 = ct{1350};
t5403 = ct{1351};
t5404 = ct{1352};
t542 = ct{1353};
t543 = ct{1354};
t5433 = ct{1355};
t5434 = ct{1356};
t5436 = ct{1357};
t5437 = ct{1358};
t5438 = ct{1359};
t5439 = ct{1360};
t5452 = ct{1361};
t5456 = ct{1362};
t5457 = ct{1363};
t5458 = ct{1364};
t5459 = ct{1365};
t5460 = ct{1366};
t5464 = ct{1367};
t5481 = ct{1368};
t549 = ct{1369};
t5499 = ct{1370};
t5537 = ct{1371};
t5540 = ct{1372};
t5541 = ct{1373};
t5542 = ct{1374};
t5544 = ct{1375};
t5545 = ct{1376};
t5548 = ct{1377};
t5550 = ct{1378};
t5561 = ct{1379};
t5569 = ct{1380};
t5570 = ct{1381};
t5586 = ct{1382};
t56 = ct{1383};
t5604 = ct{1384};
t5607 = ct{1385};
t562 = ct{1386};
t563 = ct{1387};
t5678 = ct{1388};
t5684 = ct{1389};
t575 = ct{1390};
t5782 = ct{1391};
t5783 = ct{1392};
t58 = ct{1393};
t587 = ct{1394};
t59 = ct{1395};
t5901 = ct{1396};
t5902 = ct{1397};
t594 = ct{1398};
t5990 = ct{1399};
t60 = ct{1400};
t6011 = ct{1401};
t6013 = ct{1402};
t6014 = ct{1403};
t610 = ct{1404};
t6255 = ct{1405};
t6256 = ct{1406};
t6257 = ct{1407};
t628 = ct{1408};
t635 = ct{1409};
t636 = ct{1410};
t638 = ct{1411};
t640 = ct{1412};
t641 = ct{1413};
t642 = ct{1414};
t643 = ct{1415};
t644 = ct{1416};
t645 = ct{1417};
t646 = ct{1418};
t649 = ct{1419};
t654 = ct{1420};
t655 = ct{1421};
t656 = ct{1422};
t657 = ct{1423};
t659 = ct{1424};
t660 = ct{1425};
t6622 = ct{1426};
t6623 = ct{1427};
t663 = ct{1428};
t664 = ct{1429};
t665 = ct{1430};
t666 = ct{1431};
t667 = ct{1432};
t668 = ct{1433};
t669 = ct{1434};
t67 = ct{1435};
t670 = ct{1436};
t672 = ct{1437};
t673 = ct{1438};
t674 = ct{1439};
t6745 = ct{1440};
t675 = ct{1441};
t6751 = ct{1442};
t676 = ct{1443};
t677 = ct{1444};
t678 = ct{1445};
t679 = ct{1446};
t68 = ct{1447};
t681 = ct{1448};
t682 = ct{1449};
t683 = ct{1450};
t684 = ct{1451};
t685 = ct{1452};
t686 = ct{1453};
t687 = ct{1454};
t689 = ct{1455};
t691 = ct{1456};
t6919 = ct{1457};
t692 = ct{1458};
t6920 = ct{1459};
t693 = ct{1460};
t694 = ct{1461};
t6987 = ct{1462};
t70 = ct{1463};
t702 = ct{1464};
t707 = ct{1465};
t708 = ct{1466};
t71 = ct{1467};
t710 = ct{1468};
t715 = ct{1469};
t716 = ct{1470};
t717 = ct{1471};
t718 = ct{1472};
t721 = ct{1473};
t722 = ct{1474};
t724 = ct{1475};
t725 = ct{1476};
t73 = ct{1477};
t736 = ct{1478};
t738 = ct{1479};
t740 = ct{1480};
t741 = ct{1481};
t749 = ct{1482};
t756 = ct{1483};
t76 = ct{1484};
t762 = ct{1485};
t768 = ct{1486};
t777 = ct{1487};
t792 = ct{1488};
t793 = ct{1489};
t8 = ct{1490};
t801 = ct{1491};
t802 = ct{1492};
t808 = ct{1493};
t813 = ct{1494};
t819 = ct{1495};
t821 = ct{1496};
t850 = ct{1497};
t855 = ct{1498};
t874 = ct{1499};
t878 = ct{1500};
t89 = ct{1501};
t9 = ct{1502};
t90 = ct{1503};
t91 = ct{1504};
t92 = ct{1505};
t941 = ct{1506};
t944 = ct{1507};
t945 = ct{1508};
t948 = ct{1509};
t949 = ct{1510};
t951 = ct{1511};
t97 = ct{1512};
t983 = ct{1513};
t996 = ct{1514};
t4118 = t945+t3917;
t4120 = t949+t3919;
t4131 = -t11.*(t944-t3919);
t4133 = -t16.*(t944-t3919);
t4140 = t11.*(t944-t3919);
t4144 = t16.*(t944-t3919).*(-3.0./5.0e+2);
t4148 = t1023+t3941;
t4151 = t1045+t3940;
t4164 = t21.*(t3941-(t262.*(t46-t47))./9.007199254740992e+15);
t4166 = t27.*(t3941-(t262.*(t46-t47))./9.007199254740992e+15);
t4172 = t549+t1874+t1882+t1890+t1911+t2755+t2794;
t4175 = -t4165;
t4181 = t4155.*(3.0./5.0e+2);
t4187 = t2818+t2819+t3115+t3116;
t4202 = t16.*(t944-t3919).*(-5.68686e-3);
t4210 = t16.*(t944-t3919).*(-3.131399999999998e-4);
t4213 = t188.*t3934.*(t42-t43).*(-2.442490654175345e-23);
t4214 = t188.*t3934.*(t42-t43).*2.442490654175345e-23;
t4215 = t587+t1879+t1923+t1931+t1963+t2844+t2910;
t4217 = t4165.*1.247162e-2;
t4226 = t4155.*3.131399999999998e-4;
t4228 = t4155.*4.36041e-5;
t4235 = -t4233;
t4237 = -t3483.*(t1896-t3239);
t4246 = t4155.*6.1855407534e-5;
t4248 = t4165.*1.35652563578e-4;
t4257 = t50.*t189.*t3934.*(t42-t43).*(-2.711709361697228e-39);
t4259 = t50.*t189.*t3934.*(t42-t43).*2.711709361697228e-39;
t4278 = ((t1861-t3221).*(t1896-t3239))./1.0e+8;
t4295 = (t1861-t3221).*(t1896-t3239).*6.2e-7;
t4297 = t16.*(t1861-t3221).*(t1896-t3239).*5.7e-7;
t4298 = t11.*(t1861-t3221).*(t1896-t3239).*1.02e-6;
t4301 = t11.*(t1861-t3221).*(t1896-t3239).*2.4e-7;
t4302 = t11.*(t1861-t3221).*(t1896-t3239).*4.0e-8;
t4303 = t16.*(t1861-t3221).*(t1896-t3239).*4.0e-8;
t4329 = t2973.*(t3941-(t262.*(t46-t47))./9.007199254740992e+15);
t4350 = t1889+t1948+t2766+t2815+t3089+t3090;
t4360 = t2961+t3536+t3539;
t4371 = t1930+t1971+t2862+t2932+t3110+t3111;
t4379 = t3237.*(-t1901+t3122+t3277).*(-3.24e-6);
t4380 = t3237.*(-t1901+t3122+t3277).*(-3.11e-6);
t4383 = t3217.*t3934.*1.1e-7;
t4386 = t3217.*t3934.*3.24e-6;
t4388 = t3217.*t3934.*3.11e-6;
t4394 = t3217.*t3937.*3.11e-6;
t4396 = t3217.*t3937.*3.24e-6;
t4397 = t3217.*t3934.*5.0e-8;
t4399 = t3218.*t3934.*5.0e-8;
t4400 = t3218.*t3934.*1.6e-7;
t4412 = -t3143.*(-t2804+t2838+t3109+t17.*(t1456-t2355).*9.3e-7);
t4414 = t3143.*(-t2804+t2838+t3109+t17.*(t1456-t2355).*9.3e-7);
t4418 = t530+t1918+t2743+t2751+t2761+t2763+t2764+t2793;
t4452 = t563+t1964+t2832+t2836+t2853+t2889+t2897+t2909;
t4457 = t3216.*t4146;
t4459 = t3217.*t4146;
t4467 = t3237.*(t951+t10.*(-t1881+t3121+t3276)).*(-1.0e-8);
t4470 = t3236.*(t944-t3919).*(-9.840000000000001e-6);
t4471 = t3237.*((t237.*(t42-t43))./9.007199254740992e+15+t15.*(-t1881+t3121+t3276)).*(-9.840000000000001e-6);
t4472 = t3236.*(t944-t3919).*9.840000000000001e-6;
t4480 = t3237.*(t951+t10.*(-t1881+t3121+t3276)).*(-3.24e-6);
t4481 = t3237.*(t951+t10.*(-t1881+t3121+t3276)).*(-7.83e-6);
t4482 = t3237.*(t951+t10.*(-t1881+t3121+t3276)).*(-6.2e-7);
t4484 = (t2527-t3009).*(-t2804+t2838+t3109+t17.*(t1456-t2355).*9.3e-7);
t4489 = t188.*t4437.*4.297799892626299e-1;
t4490 = t1526+t1900+t2553+t2817+t2837+t3113+t3114;
t4494 = ((t1861-t3221).*(t2694-t2701+t3036-t3043))./1.0e+8;
t4496 = ((t1861-t3221).*(t1959-t3313+t38.*t1022.*(t855-t878).*2.196325630278387e-1))./1.0e+8;
t4504 = t3395.*t4160;
t4505 = -t3395.*(-t2804+t2838+t3109+t17.*(t1456-t2355).*9.3e-7);
t4506 = -t3395.*(t2813-t2835+t12.*(t1456-t2355).*1.02e-6+t17.*(t1456-t2355).*9.0e-8);
t4507 = (t1861-t3221).*(t2694-t2701+t3036-t3043).*9.840000000000001e-6;
t4512 = -t3396.*(-t2804+t2838+t3109+t17.*(t1456-t2355).*9.3e-7);
t4514 = -t3396.*(t2813-t2835+t12.*(t1456-t2355).*1.02e-6+t17.*(t1456-t2355).*9.0e-8);
t4515 = t3396.*t4163;
t4517 = (t1861-t3221).*(t2694-t2701+t3036-t3043).*6.2e-7;
t4519 = (t1861-t3221).*(t2694-t2701+t3036-t3043).*3.24e-6;
t4521 = (t1861-t3221).*(t2694-t2701+t3036-t3043).*7.83e-6;
t4522 = t3395.*(t2813-t2835+t12.*(t1456-t2355).*1.02e-6+t17.*(t1456-t2355).*9.0e-8).*(-1.0./2.0);
t4526 = t3396.*(t2813-t2835+t12.*(t1456-t2355).*1.02e-6+t17.*(t1456-t2355).*9.0e-8);
t4530 = (t1861-t3221).*(t1959-t3313+t38.*t1022.*(t855-t878).*2.196325630278387e-1).*7.83e-6;
t4532 = (t1861-t3221).*(t1959-t3313+t38.*t1022.*(t855-t878).*2.196325630278387e-1).*6.2e-7;
t4533 = t16.*(t1861-t3221).*(t2694-t2701+t3036-t3043).*5.7e-7;
t4535 = t11.*(t1861-t3221).*(t2694-t2701+t3036-t3043).*1.02e-6;
t4537 = t3396.*(-t2804+t2838+t3109+t17.*(t1456-t2355).*9.3e-7).*(-1.0./2.0);
t4540 = (t1861-t3221).*(t1959-t3313+t38.*t1022.*(t855-t878).*2.196325630278387e-1).*3.24e-6;
t4544 = t11.*(t1861-t3221).*(t2694-t2701+t3036-t3043).*2.4e-7;
t4546 = t11.*(t1861-t3221).*(t2694-t2701+t3036-t3043).*4.0e-8;
t4547 = t16.*(t1861-t3221).*(t2694-t2701+t3036-t3043).*4.0e-8;
t4637 = -t3483.*(t1005+t20.*(t1941-t3315+t39.*t1022.*(t855-t878).*2.196325630278387e-1));
t4650 = -t4146.*(t1861-t3221);
t4657 = ((t1005+t20.*(t1941-t3315+t39.*t1022.*(t855-t878).*2.196325630278387e-1)).*(t1861-t3221))./1.0e+8;
t4670 = (t1005+t20.*(t1941-t3315+t39.*t1022.*(t855-t878).*2.196325630278387e-1)).*(t1861-t3221).*6.2e-7;
t4745 = t3934.*(-t1901+t3122+t3277).*(-1.1e-7);
t4747 = t3934.*(-t1901+t3122+t3277).*(-3.24e-6);
t4748 = t3934.*(-t1881+t3121+t3276).*(-5.0e-8);
t4752 = t3934.*(-t1881+t3121+t3276).*(-1.6e-7);
t4753 = t3934.*(-t1901+t3122+t3277).*(-3.11e-6);
t4758 = t3934.*(-t1901+t3122+t3277).*(-5.0e-8);
t4765 = t524+t575+t1488+t1870+t1886+t1957+t2519+t2740+t2747+t3096+t3097;
t4834 = t543+t610+t1513+t1876+t1927+t1998+t2598+t2820+t2834+t3117+t3118;
t4841 = t12.*t4837;
t4842 = t17.*t4837;
t4849 = t3934.*(t951+t10.*(-t1881+t3121+t3276)).*(-1.0e-8);
t4853 = t587+t1931+t1963+t2004+t2817+t2837+t2844+t2934+t3113+t3114;
t4874 = t3947+t4155;
t4877 = t3934.*((t237.*(t42-t43))./9.007199254740992e+15+t15.*(-t1881+t3121+t3276)).*(-9.840000000000001e-6);
t4878 = (t944-t3919).*(t2694-t2701+t3036-t3043).*9.840000000000001e-6;
t4890 = t3934.*(t951+t10.*(-t1881+t3121+t3276)).*(-3.24e-6);
t4891 = t3934.*(t951+t10.*(-t1881+t3121+t3276)).*(-7.83e-6);
t4892 = t3934.*(t951+t10.*(-t1881+t3121+t3276)).*(-6.2e-7);
t5014 = t50.*t189.*t4951.*4.771516396025243e-17;
t5017 = -t5016;
t5052 = -t3133.*(t4165+t27.*(t1959-t3313+t38.*t1022.*(t855-t878).*2.196325630278387e-1));
t5053 = t3133.*(t4165+t27.*(t1959-t3313+t38.*t1022.*(t855-t878).*2.196325630278387e-1));
t5058 = t3237.*(t11.*((t237.*(t42-t43))./9.007199254740992e+15+t15.*(-t1881+t3121+t3276))+t16.*(-t1901+t3122+t3277)).*(-1.0e-8);
t5059 = (t3237.*(t11.*((t237.*(t42-t43))./9.007199254740992e+15+t15.*(-t1881+t3121+t3276))+t16.*(-t1901+t3122+t3277)))./1.0e+8;
t5065 = t3237.*(t11.*((t237.*(t42-t43))./9.007199254740992e+15+t15.*(-t1881+t3121+t3276))+t16.*(-t1901+t3122+t3277)).*(-1.02e-6);
t5066 = t3237.*(t11.*((t237.*(t42-t43))./9.007199254740992e+15+t15.*(-t1881+t3121+t3276))+t16.*(-t1901+t3122+t3277)).*1.02e-6;
t5068 = t3237.*(t11.*((t237.*(t42-t43))./9.007199254740992e+15+t15.*(-t1881+t3121+t3276))+t16.*(-t1901+t3122+t3277)).*(-2.4e-7);
t5070 = t3237.*t4837.*5.7e-7;
t5072 = t3237.*(t11.*((t237.*(t42-t43))./9.007199254740992e+15+t15.*(-t1881+t3121+t3276))+t16.*(-t1901+t3122+t3277)).*2.4e-7;
t5075 = t3237.*(t11.*((t237.*(t42-t43))./9.007199254740992e+15+t15.*(-t1881+t3121+t3276))+t16.*(-t1901+t3122+t3277)).*(-4.0e-8);
t5078 = t3237.*t4837.*4.0e-8;
t5084 = t3217.*t4915.*1.1e-7;
t5085 = t3217.*t4915.*3.24e-6;
t5086 = t3217.*t4915.*3.11e-6;
t5088 = t3217.*t4915.*5.0e-8;
t5089 = t3218.*t4915.*5.0e-8;
t5090 = t3218.*t4915.*1.6e-7;
t5092 = -t5087;
t5094 = -t5091;
t5095 = -t5093;
t5099 = -t5097;
t5111 = -t4814.*(t1861-t3221);
t5203 = t4920.*(t1861-t3221).*(-1.0e-8);
t5217 = t4920.*(t1861-t3221).*(-3.24e-6);
t5218 = t4920.*(t1861-t3221).*(-7.83e-6);
t5219 = t4920.*(t1861-t3221).*(-6.2e-7);
t5242 = t3184+t3191+t3319+t3325+t3473+t3491;
t5274 = t3934.*(t11.*((t237.*(t42-t43))./9.007199254740992e+15+t15.*(-t1881+t3121+t3276))+t16.*(-t1901+t3122+t3277)).*(-1.0e-8);
t5276 = (t3934.*(t11.*((t237.*(t42-t43))./9.007199254740992e+15+t15.*(-t1881+t3121+t3276))+t16.*(-t1901+t3122+t3277)))./1.0e+8;
t5285 = t3934.*(t11.*((t237.*(t42-t43))./9.007199254740992e+15+t15.*(-t1881+t3121+t3276))+t16.*(-t1901+t3122+t3277)).*(-1.02e-6);
t5286 = t3934.*(t11.*((t237.*(t42-t43))./9.007199254740992e+15+t15.*(-t1881+t3121+t3276))+t16.*(-t1901+t3122+t3277)).*(-2.4e-7);
t5287 = t3934.*t4837.*5.7e-7;
t5289 = t3934.*(t11.*((t237.*(t42-t43))./9.007199254740992e+15+t15.*(-t1881+t3121+t3276))+t16.*(-t1901+t3122+t3277)).*2.4e-7;
t5291 = t3934.*(t11.*((t237.*(t42-t43))./9.007199254740992e+15+t15.*(-t1881+t3121+t3276))+t16.*(-t1901+t3122+t3277)).*(-4.0e-8);
t5295 = t3934.*(t11.*((t237.*(t42-t43))./9.007199254740992e+15+t15.*(-t1881+t3121+t3276))+t16.*(-t1901+t3122+t3277)).*4.0e-8;
t5297 = t3934.*t4837.*4.0e-8;
t5301 = t3369.*t3638.*t3910.*t3934.*1.444822e-2;
t5303 = t3322.*t3649.*t3910.*t3934.*1.444822e-2;
t5311 = -t4814.*(t951+t10.*(-t1881+t3121+t3276));
t5312 = t4814.*(t951+t10.*(-t1881+t3121+t3276));
t5479 = t2507+t2517+t3476+t3477+t4232+t4234;
t5760 = t3910.*t3934.*t4146.*(t1513+t1879+t2598+t2820+t2834+t3117+t3118).*(-3.633675e-3);
t5761 = t4146.*(t2674-t2676+t3022-t3027).*(t2694-t2701+t3036-t3043).*(t1513+t1879+t2598+t2820+t2834+t3117+t3118).*(-3.633675e-3);
et34 = t2500-t2507-t3476-t3477+t50.*t189.*(t1941-t3315+t39.*t1022.*(t855-t878).*2.196325630278387e-1).*4.306286555174926e-24;
et35 = t50.*t189.*(t1959-t3313+t38.*t1022.*(t855-t878).*2.196325630278387e-1).*7.660522649005482e-24;
t5779 = ((et34+et35).*(t2674-t2676+t3022-t3027))./2.0;
t5896 = t3649.*t3934.*t5561.*1.444822e-2;
t6003 = t1558+t2385+t2386+t2393+t2396+t3955+t3963+t3964+t4194+t4206;
t6315 = t3810.*t6011.*(t2694-t2701+t3036-t3043).*(-5.43845e-3);
et36 = t707+t708-t721-t722-t749+t762+t768-t777-t792-t793-t801-t802-t808+t813-t819+t821-t1629+t1637-t1640-t1641-t1659-t1661+t1666+t1667+t1683+t1692+t1705-t1712+t1758+t1759+t1775+t1776+t1973+t1993+t1994+t2023+t2053+t2060-t2089-t2090+t2098+t2099-t8.*t9.*t15.*t50.*t189.*3.670836568391568e-22;
et37 = t10.*t13.*t14.*t50.*t189.*(-3.279367663374749e-19)-t8.*t9.*t11.*t15.*t50.*t189.*7.075931802640439e-19;
et38 = t8.*t11.*t14.*t15.*t50.*t189.*(-1.190170786299927e-18)-t9.*t11.*t13.*t15.*t50.*t189.*1.190170786299927e-18;
et39 = t13.*t14.*t15.*t16.*t50.*t189.*(-3.226512155691387e-19);
t6320 = t3810.*t3934.*(et36+et37+et38+et39).*(-5.43845e-3);
t6563 = t3808.*t6255.*(t2674-t2676+t3022-t3027).*(-1.0./2.0);
t6564 = (t3808.*t6255.*(t2674-t2676+t3022-t3027))./2.0;
et40 = t1288+t1289+t1302+t1303-t1319-t1320+t1336-t1348+t1350+t1351-t1360+t1369-t1378+t1396-t1425+t1435-t2174+t2183-t2187+t2193-t2194-t2195+t2199-t2203-t2215+t2219-t2222-t2223+t2239+t2240-t2256-t2257+t2555+t2556+t2572+t2583-t2605-t2606+t2612+t2613-t2618-t2619+t2651+t2652;
et41 = t18.*t19.*t20.*t50.*t202.*(-3.566935413776081e-21);
et42 = t24.*t25.*t26.*t50.*t202.*(-3.992732227073824e-24);
et43 = t18.*t19.*t26.*t27.*t50.*t202.*(-3.509445006623964e-21);
et44 = t21.*t24.*t25.*t26.*t50.*t202.*(-7.696420262413979e-21);
t6565 = t3808.*t3910.*(et40+et41+et42+et43+et44).*(-1.0./2.0);
et45 = t1288+t1289+t1302+t1303-t1319-t1320+t1336-t1348+t1350+t1351-t1360+t1369-t1378+t1396-t1425+t1435-t2174+t2183-t2187+t2193-t2194-t2195+t2199-t2203-t2215+t2219-t2222-t2223+t2239+t2240-t2256-t2257+t2555+t2556+t2572+t2583-t2605-t2606+t2612+t2613-t2618-t2619+t2651+t2652;
et46 = t18.*t19.*t20.*t50.*t202.*(-3.566935413776081e-21);
et47 = t24.*t25.*t26.*t50.*t202.*(-3.992732227073824e-24);
et48 = t18.*t19.*t26.*t27.*t50.*t202.*(-3.509445006623964e-21);
et49 = t21.*t24.*t25.*t26.*t50.*t202.*(-7.696420262413979e-21);
t7150 = ((et45+et46+et47+et48+et49).*(t1554+t2361+t2362+t2367+t2414+t3961+t3968+t4198+t4201+t11.*(-t1901+t3122+t3277).*5.68686e-3))./2.0;
t3206 = -t3203;
t3232 = t3227.*(3.0./5.0e+2);
t3233 = -t3230;
t3234 = t3229.*(3.0./5.0e+2);
t3249 = t2410+t2997;
t3252 = t3245.*(3.0./5.0e+2);
t3253 = -t3250;
t3254 = t3247.*(3.0./5.0e+2);
t3255 = -t3251;
t3282 = t3227.*1.247162e-2;
t3283 = t3229.*1.247162e-2;
t3284 = -t3279;
t3288 = -t3280;
t3289 = t3226.*5.84482e-3;
t3291 = -t3281;
t3292 = t3228.*5.84482e-3;
t3294 = t3227.*5.68686e-3;
t3295 = t3229.*5.68686e-3;
t3296 = -t3286;
t3297 = -t3287;
t3298 = t3226.*6.48e-5;
t3300 = -t3290;
t3301 = t3228.*6.48e-5;
t3308 = t3227.*3.131399999999998e-4;
t3309 = t3229.*3.131399999999998e-4;
t3310 = -t3306;
t3311 = t3226.*6.47e-6;
t3312 = t3228.*6.47e-6;
t3332 = t3245.*1.247162e-2;
t3333 = -t3328;
t3334 = t3247.*1.247162e-2;
t3335 = -t3329;
t3338 = -t3330;
t3339 = t3244.*5.84482e-3;
t3341 = -t3331;
t3342 = t3246.*5.84482e-3;
t3346 = t3244.*6.48e-5;
t3348 = -t3340;
t3349 = t3246.*6.48e-5;
t3352 = t3247.*3.131399999999998e-4;
t3353 = -t3344;
t3360 = t3245.*3.131399999999998e-4;
t3361 = -t3356;
t3362 = t3244.*6.47e-6;
t3363 = t3246.*6.47e-6;
t3364 = t3245.*4.36041e-5;
t3365 = t3247.*4.36041e-5;
t3366 = -t3359;
t3404 = t3245.*1.35652563578e-4;
t3405 = t3247.*1.35652563578e-4;
t3406 = -t3400;
t3407 = t3244.*1.688944904408e-4;
t3408 = t3246.*1.688944904408e-4;
t3409 = t3245.*6.1855407534e-5;
t3410 = t3247.*6.1855407534e-5;
t3411 = -t3403;
t3419 = -t3412;
t3420 = t3244.*7.0482312e-7;
t3421 = t3246.*7.0482312e-7;
t3422 = t3244.*1.869599668e-7;
t3423 = t3246.*1.869599668e-7;
t3430 = -t3428;
t3444 = -t3436;
t3480 = t3475./2.0;
t3481 = -t3479;
t3495 = -t3493;
t3498 = -t3497;
t3502 = t1865+t3226;
t3503 = t1868+t3228;
t3504 = t11.*t3500;
t3505 = t12.*t3500;
t3506 = t16.*t3500;
t3507 = t17.*t3500;
t3513 = t16.*t3508;
t3514 = t16.*t3509;
t3542 = -t3540;
t3547 = t1913+t3244;
t3548 = t50.*t202.*t3243.*9.733893447891495e-23;
t3550 = t1933+t3246;
t3553 = t50.*t202.*t3243.*8.588729512845436e-24;
t3554 = t21.*t3543;
t3555 = t22.*t3543;
t3556 = t27.*t3543;
t3557 = t28.*t3543;
t3570 = t27.*t3559;
t3571 = t27.*t3560;
t3582 = t27.*t3566;
t3616 = t16.*t3598;
t3619 = t3524.*(-1.838876e-2);
t3643 = t3566.*(-9.99471e-3);
t3645 = t3566.*(-1.838876e-2);
t3651 = t3566.*9.99471e-3;
t3668 = t27.*t3644;
t3680 = t3055.*t3063;
t3686 = t3683./2.0;
t3690 = -t3687;
t3697 = -t3695;
t3713 = t2363.*t3243.*1.02e-6;
t3722 = t3566.*(-1.33637554986e-4);
t3725 = t3566.*(-7.26350557185e-5);
t3728 = t2363.*t3243.*9.0e-8;
t3734 = t3566.*7.26350557185e-5;
t3748 = t27.*t3726;
t3766 = t3763.*(-1.0./2.0);
t3768 = t2363.*t3431;
t3775 = -t3773;
t3781 = t21.*t3771;
t3783 = -t3778;
t3786 = -t3782;
t3789 = t21.*t3774;
t3795 = -t3791;
t3801 = -t3799;
t3804 = -t3803;
t3818 = t3813./2.0;
t3822 = t3816./2.0;
t3825 = t3055.*t3243.*1.02e-6;
t3829 = t3055.*t3243.*9.0e-8;
t3841 = t2971.*t3543;
t3842 = t2972.*t3543;
t3843 = -t3839;
t3845 = -t3840;
t3847 = t2973.*t3543;
t3850 = -t3846;
t3887 = t27.*t2363.*t3815;
t3888 = -t3885;
t3904 = -t3711.*(t1477-t2502);
t3905 = t3711.*(t1477-t2502);
t3928 = t3155.*t3543;
t3952 = t2998.*t3815;
t3958 = -t3953;
t3959 = -t3954;
t3966 = -t3957;
t3973 = -t3970;
t3977 = t2904+t2929+t3033+t3034;
t3979 = t2864+t2938+t3032+t3035;
t3983 = -t3978;
t3988 = -t3981;
t3992 = -t3986;
t4009 = (t3236.*t3500)./1.0e+8;
t4012 = t11.*t4010;
t4021 = t3055.*t3815;
t4023 = -t3815.*(t1477-t2502);
t4029 = t3815.*(t1477-t2502);
t4033 = t4028.*(-1.0./2.0);
t4037 = -t4032;
t4039 = t4028./2.0;
t4041 = t4027./2.0;
t4058 = t3236.*t3500.*9.840000000000001e-6;
t4066 = t3236.*t3500.*6.2e-7;
t4067 = t3236.*t3500.*3.24e-6;
t4068 = t3236.*t3500.*7.83e-6;
t4125 = t12.*t4118;
t4126 = t17.*t4118;
t4169 = t22.*t4151;
t4171 = t28.*t4151;
t4176 = -t4166;
t4182 = t4166.*(3.0./5.0e+2);
t4192 = t21.*t2363.*t3893;
t4195 = t4140.*(-1.247162e-2);
t4200 = t4140.*1.247162e-2;
t4204 = -t3431.*(t1896-t3239);
t4216 = t4164.*1.247162e-2;
t4225 = t4166.*3.131399999999998e-4;
t4227 = t4166.*4.36041e-5;
t4236 = t3483.*t3543;
t4238 = t3055.*t3872;
t4245 = t4166.*6.1855407534e-5;
t4247 = t4164.*1.35652563578e-4;
t4253 = -t4248;
t4266 = t3395.*t3759;
t4268 = t3396.*t3760;
t4276 = t3500.*(t1896-t3239).*(-1.0e-8);
t4277 = t3543.*(t1861-t3221).*(-1.0e-8);
t4279 = t11.*t4278;
t4284 = t3003.*t3893;
t4293 = t3500.*(t1896-t3239).*(-6.2e-7);
t4294 = t3543.*(t1861-t3221).*(-6.2e-7);
t4306 = -t4302;
t4307 = -t4303;
t4316 = t3055.*t3893;
t4317 = -t3893.*(t1477-t2502);
t4318 = t3893.*(t1477-t2502).*(-1.0./2.0);
t4322 = t2290+t2312+t3281+t3306;
t4330 = -t27.*t3815.*(t1896-t3239);
t4331 = -t4329;
t4333 = t27.*t3815.*(t1896-t3239);
t4335 = t3395.*t3873;
t4336 = t3396.*t3874;
t4346 = t528+t1000+t2523+t2789+t2809+t3020+t3021;
t4352 = t562+t1003+t2636+t2902+t2921+t3040+t3041;
t4356 = t3216.*t3925;
t4358 = t3217.*t3925;
t4374 = t2732+t2791+t3401+t3417;
t4405 = t3236.*t3951.*7.26735e-3;
t4406 = t3237.*t3951.*7.26735e-3;
t4416 = t4414.*(-1.0./2.0);
t4417 = t4414./2.0;
t4419 = t523+t594+t1905+t1954+t3975;
t4420 = t3155.*t4151;
t4454 = t542+t644+t1945+t1992+t4018;
t4462 = -t21.*t3893.*(t1896-t3239);
t4463 = (t3236.*t4118)./1.0e+8;
t4473 = t3236.*t4118.*3.24e-6;
t4474 = t3236.*t4118.*7.83e-6;
t4475 = t3236.*t4118.*6.2e-7;
t4483 = -t3257.*(t2813-t2835+t12.*(t1456-t2355).*1.02e-6+t17.*(t1456-t2355).*9.0e-8);
t4485 = t3257.*(t2813-t2835+t12.*(t1456-t2355).*1.02e-6+t17.*(t1456-t2355).*9.0e-8);
t4487 = -t4484;
t4488 = t4484./2.0;
t4491 = t3236.*t4187.*7.26735e-3;
t4492 = t3500.*(t2694-t2701+t3036-t3043).*(-1.0e-8);
t4493 = t3237.*t4187.*7.26735e-3;
t4498 = t11.*t4494;
t4503 = t3500.*(t2694-t2701+t3036-t3043).*(-9.840000000000001e-6);
t4508 = t3500.*(t1959-t3313+t38.*t1022.*(t855-t878).*2.196325630278387e-1).*(-9.840000000000001e-6);
t4510 = t3500.*(t2694-t2701+t3036-t3043).*(-6.2e-7);
t4511 = t3500.*(t2694-t2701+t3036-t3043).*(-3.24e-6);
t4513 = t3500.*(t2694-t2701+t3036-t3043).*(-7.83e-6);
t4520 = t4504./2.0;
t4527 = -t4515;
t4539 = t4515./2.0;
t4541 = -t4533;
t4551 = -t4547;
t4636 = t3483.*t4151;
t4653 = t4118.*(t1896-t3239).*(-1.0e-8);
t4654 = (t4118.*(t1896-t3239))./1.0e+8;
t4666 = t4118.*(t1896-t3239).*(-6.2e-7);
t4667 = t4118.*(t1896-t3239).*6.2e-7;
t4673 = t4187.*(t1896-t3239).*(-7.26735e-3);
t4674 = t4187.*(t1896-t3239).*7.26735e-3;
t4710 = t528+t983+t1015+t1068+t1494+t1529+t2523+t2789+t2809+t3020+t3021;
t4711 = t2292+t3290+t3604+t3611;
t4714 = t1018+t1020+t1049+t1505+t2760+t2789+t2809+t2822+t3020+t3021;
t4715 = t562+t996+t1046+t1093+t1516+t1543+t2636+t2902+t2921+t3040+t3041;
t4723 = t1050+t1051+t1067+t1527+t2852+t2902+t2921+t2936+t3040+t3041;
t4736 = -t4350.*(t1861-t3221);
t4739 = t4350.*(t1861-t3221);
t4774 = t2757+t3413+t3727+t3730;
t4820 = t4371.*(t1896-t3239).*(-7.26735e-3);
t4835 = t3920+t4133;
t4838 = t3922+t4140;
t4843 = -t4418.*(t1861-t3221);
t4845 = t4418.*(t1861-t3221);
t4848 = t4118.*(t2694-t2701+t3036-t3043).*(-1.0e-8);
t4869 = t4841.*1.838876e-2;
t4871 = t4842.*9.99471e-3;
t4872 = t3942+t4164;
t4882 = t3948+t4175;
t4884 = t4118.*(t2694-t2701+t3036-t3043).*(-3.24e-6);
t4885 = t4118.*(t2694-t2701+t3036-t3043).*(-7.83e-6);
t4886 = t4118.*(t2694-t2701+t3036-t3043).*(-6.2e-7);
t4893 = t22.*t4874;
t4894 = t28.*t4874;
t4925 = t4452.*(t1896-t3239).*(-7.26735e-3);
t4926 = t4452.*(t1896-t3239).*7.26735e-3;
t5028 = t4252+t4259;
t5045 = t3216.*t4765;
t5046 = t3217.*t4765;
t5062 = t3236.*t4834.*7.26735e-3;
t5063 = t3237.*t4834.*7.26735e-3;
t5079 = -t5078;
t5108 = t3500.*t4814;
t5194 = t3543.*t4853.*7.26735e-3;
t5195 = t4853.*(t1896-t3239).*(-7.26735e-3);
t5209 = t3500.*t4920.*9.840000000000001e-6;
t5240 = t3815.*t4874;
t5250 = t50.*t189.*t5242.*4.771516396025243e-17;
t5252 = t3915.*t4765;
t5253 = -t4765.*(-t1901+t3122+t3277);
